simulink library "outp"  (R2021b)
(part 6 of 7)

      link override Signal_Override/_ovrdval: Value=KOUTP_FrUdcMax_V_ovrdval
  VTQD_FrUdcMin_V_Inproc : FVT_lib/outp/OverrideAndLimit  SystemSampleTime=-1  VariantActivationTime=update diagram  Latency=0  AutoFrameSizeCalculation=off
      link override Signal_Limit/_maxval: Value=KOUTP_FrUdcMin_V_maxval
      link override Signal_Limit/_minval: Value=KOUTP_FrUdcMin_V_minval
      link override Signal_Override/_ovrdflg: Value=KOUTP_FrUdcMin_V_ovrdflg
      link override Signal_Override/_ovrdval: Value=KOUTP_FrUdcMin_V_ovrdval
  VTQD_NFricPercTorq_pct_Inproc : FVT_lib/outp/OverrideAndLimit  SystemSampleTime=-1  VariantActivationTime=update diagram  Latency=0  AutoFrameSizeCalculation=off
      link override Signal_Limit/_maxval: Value=KOUTP_NFricPercTorq_pct_maxval
      link override Signal_Limit/_minval: Value=KOUTP_NFricPercTorq_pct_minval
      link override Signal_Override/_ovrdflg: Value=KOUTP_NFricPercTorq_pct_ovrdflg
      link override Signal_Override/_ovrdval: Value=KOUTP_NFricPercTorq_pct_ovrdval
  VTQD_PButtonSta_enum_Inproc : FVT_lib/outp/OverrideAndLimit  SystemSampleTime=-1  VariantActivationTime=update diagram  Latency=0  AutoFrameSizeCalculation=off
      link override Signal_Limit/_maxval: Value=KOUTP_PButtonSta_enum_maxval
      link override Signal_Limit/_minval: Value=KOUTP_PButtonSta_enum_minval
      link override Signal_Override/_ovrdflg: Value=KOUTP_PButtonSta_enum_ovrdflg
      link override Signal_Override/_ovrdval: Value=KOUTP_PButtonSta_enum_ovrdval
  VTQD_PTCSPermSta_flg_Inproc : FVT_lib/outp/OverrideAndLimit  SystemSampleTime=-1  VariantActivationTime=update diagram  Latency=0  AutoFrameSizeCalculation=off
      link override Signal_Limit/_maxval: Value=KOUTP_PTCSPermSta_flg_maxval
      link override Signal_Limit/_minval: Value=KOUTP_PTCSPermSta_flg_minval
      link override Signal_Override/_ovrdflg: Value=KOUTP_PTCSPermSta_flg_ovrdflg
      link override Signal_Override/_ovrdval: Value=KOUTP_PTCSPermSta_flg_ovrdval
  VTQD_ParkBrakeSW_enum_Inproc : FVT_lib/outp/OverrideAndLimit  SystemSampleTime=-1  VariantActivationTime=update diagram  Latency=0  AutoFrameSizeCalculation=off
      link override Signal_Limit/_maxval: Value=KOUTP_ParkBrakeSW_enum_maxval
      link override Signal_Limit/_minval: Value=KOUTP_ParkBrakeSW_enum_minval
      link override Signal_Override/_ovrdflg: Value=KOUTP_ParkBrakeSW_enum_ovrdflg
      link override Signal_Override/_ovrdval: Value=KOUTP_ParkBrakeSW_enum_ovrdval
  VTQD_ParkRequest_flg_Inproc : FVT_lib/outp/OverrideAndLimit  SystemSampleTime=-1  VariantActivationTime=update diagram  Latency=0  AutoFrameSizeCalculation=off
      link override Signal_Limit/_maxval: Value=KOUTP_ParkRequest_flg_maxval
      link override Signal_Limit/_minval: Value=KOUTP_ParkRequest_flg_minval
      link override Signal_Override/_ovrdflg: Value=KOUTP_ParkRequest_flg_ovrdflg
      link override Signal_Override/_ovrdval: Value=KOUTP_ParkRequest_flg_ovrdval
  VTQD_ReBrakeLPReq_flg_Inproc : FVT_lib/outp/OverrideAndLimit  SystemSampleTime=-1  VariantActivationTime=update diagram  Latency=0  AutoFrameSizeCalculation=off
      link override Signal_Limit/_maxval: Value=KOUTP_ReBrakeLPReq_flg_maxval
      link override Signal_Limit/_minval: Value=KOUTP_ReBrakeLPReq_flg_minval
      link override Signal_Override/_ovrdflg: Value=KOUTP_ReBrakeLPReq_flg_ovrdflg
      link override Signal_Override/_ovrdval: Value=KOUTP_ReBrakeLPReq_flg_ovrdval
  VTQD_RetSelNonEng_pct_Inproc : FVT_lib/outp/OverrideAndLimit  SystemSampleTime=-1  VariantActivationTime=update diagram  Latency=0  AutoFrameSizeCalculation=off
      link override Signal_Limit/_maxval: Value=KOUTP_RetSelNonEng_pct_maxval
      link override Signal_Limit/_minval: Value=KOUTP_RetSelNonEng_pct_minval
      link override Signal_Override/_ovrdflg: Value=KOUTP_RetSelNonEng_pct_ovrdflg
      link override Signal_Override/_ovrdval: Value=KOUTP_RetSelNonEng_pct_ovrdval
  VTQD_RgnAbnorSta_flg_Inproc : FVT_lib/outp/OverrideAndLimit  SystemSampleTime=-1  VariantActivationTime=update diagram  Latency=0  AutoFrameSizeCalculation=off
      link override Signal_Limit/_maxval: Value=KOUTP_RgnAbnorSta_flg_maxval
      link override Signal_Limit/_minval: Value=KOUTP_RgnAbnorSta_flg_minval
      link override Signal_Override/_ovrdflg: Value=KOUTP_RgnAbnorSta_flg_ovrdflg
      link override Signal_Override/_ovrdval: Value=KOUTP_RgnAbnorSta_flg_ovrdval
  VTQD_RrActvDmpDisabReq_flg_Inproc : FVT_lib/outp/OverrideAndLimit  SystemSampleTime=-1  VariantActivationTime=update diagram  Latency=0  AutoFrameSizeCalculation=off
      link override Signal_Limit/_maxval: Value=KOUTP_RrActvDmpDisabReq_flg_maxval
      link override Signal_Limit/_minval: Value=KOUTP_RrActvDmpDisabReq_flg_minval
      link override Signal_Override/_ovrdflg: Value=KOUTP_RrActvDmpDisabReq_flg_ovrdflg
      link override Signal_Override/_ovrdval: Value=KOUTP_RrActvDmpDisabReq_flg_ovrdval
  VTQD_RrEDUActTq_Nm_Inproc : FVT_lib/outp/OverrideAndLimit  SystemSampleTime=-1  VariantActivationTime=update diagram  Latency=0  AutoFrameSizeCalculation=off
      link override Signal_Limit/_maxval: Value=KOUTP_RrEDUActTq_Nm_maxval
      link override Signal_Limit/_minval: Value=KOUTP_RrEDUActTq_Nm_minval
      link override Signal_Override/_ovrdflg: Value=KOUTP_RrEDUActTq_Nm_ovrdflg
      link override Signal_Override/_ovrdval: Value=KOUTP_RrEDUActTq_Nm_ovrdval
  VTQD_RrEDUAvailBrkRgnTqV_flg_Inproc : FVT_lib/outp/OverrideAndLimit  SystemSampleTime=-1  VariantActivationTime=update diagram  Latency=0  AutoFrameSizeCalculation=off
      link override Signal_Limit/_maxval: Value=KOUTP_RrEDUAvailBrkRgnTqV_flg_maxval
      link override Signal_Limit/_minval: Value=KOUTP_RrEDUAvailBrkRgnTqV_flg_minval
      link override Signal_Override/_ovrdflg: Value=KOUTP_RrEDUAvailBrkRgnTqV_flg_ovrdflg
      link override Signal_Override/_ovrdval: Value=KOUTP_RrEDUAvailBrkRgnTqV_flg_ovrdval
  VTQD_RrEDUAvailBrkRgnTq_Nm_Inproc : FVT_lib/outp/OverrideAndLimit  SystemSampleTime=-1  VariantActivationTime=update diagram  Latency=0  AutoFrameSizeCalculation=off
      link override Signal_Limit/_maxval: Value=KOUTP_RrEDUAvailBrkRgnTq_Nm_maxval
      link override Signal_Limit/_minval: Value=KOUTP_RrEDUAvailBrkRgnTq_Nm_minval
      link override Signal_Override/_ovrdflg: Value=KOUTP_RrEDUAvailBrkRgnTq_Nm_ovrdflg
      link override Signal_Override/_ovrdval: Value=KOUTP_RrEDUAvailBrkRgnTq_Nm_ovrdval
  VTQD_RrEDURolRgnTq_Nm_Inproc : FVT_lib/outp/OverrideAndLimit  SystemSampleTime=-1  VariantActivationTime=update diagram  Latency=0  AutoFrameSizeCalculation=off
      link override Signal_Limit/_maxval: Value=KOUTP_RrEDURolRgnTq_Nm_maxval
      link override Signal_Limit/_minval: Value=KOUTP_RrEDURolRgnTq_Nm_minval
      link override Signal_Override/_ovrdflg: Value=KOUTP_RrEDURolRgnTq_Nm_ovrdflg
      link override Signal_Override/_ovrdval: Value=KOUTP_RrEDURolRgnTq_Nm_ovrdval
  VTQD_RrEDUSpdValid_flg_Inproc : FVT_lib/outp/OverrideAndLimit  SystemSampleTime=-1  VariantActivationTime=update diagram  Latency=0  AutoFrameSizeCalculation=off
      link override Signal_Limit/_maxval: Value=KOUTP_RrEDUSpdValid_flg_maxval
      link override Signal_Limit/_minval: Value=KOUTP_RrEDUSpdValid_flg_minval
      link override Signal_Override/_ovrdflg: Value=KOUTP_RrEDUSpdValid_flg_ovrdflg
      link override Signal_Override/_ovrdval: Value=KOUTP_RrEDUSpdValid_flg_ovrdval
  VTQD_RrEDUSpd_rpm_Inproc : FVT_lib/outp/OverrideAndLimit  SystemSampleTime=-1  VariantActivationTime=update diagram  Latency=0  AutoFrameSizeCalculation=off
      link override Signal_Limit/_maxval: Value=KOUTP_RrEDUSpd_rpm_maxval
      link override Signal_Limit/_minval: Value=KOUTP_RrEDUSpd_rpm_minval
      link override Signal_Override/_ovrdflg: Value=KOUTP_RrEDUSpd_rpm_ovrdflg
      link override Signal_Override/_ovrdval: Value=KOUTP_RrEDUSpd_rpm_ovrdval
  VTQD_RrIdcMax_A_Inproc : FVT_lib/outp/OverrideAndLimit  SystemSampleTime=-1  VariantActivationTime=update diagram  Latency=0  AutoFrameSizeCalculation=off
      link override Signal_Limit/_maxval: Value=KOUTP_RrIdcMax_A_maxval
      link override Signal_Limit/_minval: Value=KOUTP_RrIdcMax_A_minval
      link override Signal_Override/_ovrdflg: Value=KOUTP_RrIdcMax_A_ovrdflg
      link override Signal_Override/_ovrdval: Value=KOUTP_RrIdcMax_A_ovrdval
  VTQD_RrIdcMin_A_Inproc : FVT_lib/outp/OverrideAndLimit  SystemSampleTime=-1  VariantActivationTime=update diagram  Latency=0  AutoFrameSizeCalculation=off
      link override Signal_Limit/_maxval: Value=KOUTP_RrIdcMin_A_maxval
      link override Signal_Limit/_minval: Value=KOUTP_RrIdcMin_A_minval
      link override Signal_Override/_ovrdflg: Value=KOUTP_RrIdcMin_A_ovrdflg
      link override Signal_Override/_ovrdval: Value=KOUTP_RrIdcMin_A_ovrdval
  VTQD_RrRgnDecrSta_flg_Inproc : FVT_lib/outp/OverrideAndLimit  SystemSampleTime=-1  VariantActivationTime=update diagram  Latency=0  AutoFrameSizeCalculation=off
      link override Signal_Limit/_maxval: Value=KOUTP_RrRgnDecrSta_flg_maxval
      link override Signal_Limit/_minval: Value=KOUTP_RrRgnDecrSta_flg_minval
      link override Signal_Override/_ovrdflg: Value=KOUTP_RrRgnDecrSta_flg_ovrdflg
      link override Signal_Override/_ovrdval: Value=KOUTP_RrRgnDecrSta_flg_ovrdval
  VTQD_RrRgnPermSta_flg_Inproc : FVT_lib/outp/OverrideAndLimit  SystemSampleTime=-1  VariantActivationTime=update diagram  Latency=0  AutoFrameSizeCalculation=off
      link override Signal_Limit/_maxval: Value=KOUTP_RrRgnPermSta_flg_maxval
      link override Signal_Limit/_minval: Value=KOUTP_RrRgnPermSta_flg_minval
      link override Signal_Override/_ovrdflg: Value=KOUTP_RrRgnPermSta_flg_ovrdflg
      link override Signal_Override/_ovrdval: Value=KOUTP_RrRgnPermSta_flg_ovrdval
  VTQD_RrUdcMax_V_Inproc : FVT_lib/outp/OverrideAndLimit  SystemSampleTime=-1  VariantActivationTime=update diagram  Latency=0  AutoFrameSizeCalculation=off
      link override Signal_Limit/_maxval: Value=KOUTP_RrUdcMax_V_maxval
      link override Signal_Limit/_minval: Value=KOUTP_RrUdcMax_V_minval
      link override Signal_Override/_ovrdflg: Value=KOUTP_RrUdcMax_V_ovrdflg
      link override Signal_Override/_ovrdval: Value=KOUTP_RrUdcMax_V_ovrdval
  VTQD_RrUdcMin_V_Inproc : FVT_lib/outp/OverrideAndLimit  SystemSampleTime=-1  VariantActivationTime=update diagram  Latency=0  AutoFrameSizeCalculation=off
      link override Signal_Limit/_maxval: Value=KOUTP_RrUdcMin_V_maxval
      link override Signal_Limit/_minval: Value=KOUTP_RrUdcMin_V_minval
      link override Signal_Override/_ovrdflg: Value=KOUTP_RrUdcMin_V_ovrdflg
      link override Signal_Override/_ovrdval: Value=KOUTP_RrUdcMin_V_ovrdval
  VTQD_SACtrlDev_enum_Inproc : FVT_lib/outp/OverrideAndLimit  SystemSampleTime=-1  VariantActivationTime=update diagram  Latency=0  AutoFrameSizeCalculation=off
      link override Signal_Limit/_maxval: Value=KOUTP_SACtrlDev_enum_maxval
      link override Signal_Limit/_minval: Value=KOUTP_SACtrlDev_enum_minval
      link override Signal_Override/_ovrdflg: Value=KOUTP_SACtrlDev_enum_ovrdflg
      link override Signal_Override/_ovrdval: Value=KOUTP_SACtrlDev_enum_ovrdval
  VTQD_ShiftGearPosn_enum_Inproc : FVT_lib/outp/OverrideAndLimit  SystemSampleTime=-1  VariantActivationTime=update diagram  Latency=0  AutoFrameSizeCalculation=off
      link override Signal_Limit/_maxval: Value=KOUTP_ShiftGearPosn_enum_maxval
      link override Signal_Limit/_minval: Value=KOUTP_ShiftGearPosn_enum_minval
      link override Signal_Override/_ovrdflg: Value=KOUTP_ShiftGearPosn_enum_ovrdflg
      link override Signal_Override/_ovrdval: Value=KOUTP_ShiftGearPosn_enum_ovrdval
  VTQD_ShiftPgs_enum_Inproc : FVT_lib/outp/OverrideAndLimit  SystemSampleTime=-1  VariantActivationTime=update diagram  Latency=0  AutoFrameSizeCalculation=off
      link override Signal_Limit/_maxval: Value=KOUTP_ShiftPgs_enum_maxval
      link override Signal_Limit/_minval: Value=KOUTP_ShiftPgs_enum_minval
      link override Signal_Override/_ovrdflg: Value=KOUTP_ShiftPgs_enum_ovrdflg
      link override Signal_Override/_ovrdval: Value=KOUTP_ShiftPgs_enum_ovrdval
  VTQD_TqSourceFr_enum_Inproc : FVT_lib/outp/OverrideAndLimit  SystemSampleTime=-1  VariantActivationTime=update diagram  Latency=0  AutoFrameSizeCalculation=off
      link override Signal_Limit/_maxval: Value=KOUTP_TqSourceFr_enum_maxval
      link override Signal_Limit/_minval: Value=KOUTP_TqSourceFr_enum_minval
      link override Signal_Override/_ovrdflg: Value=KOUTP_TqSourceFr_enum_ovrdflg
      link override Signal_Override/_ovrdval: Value=KOUTP_TqSourceFr_enum_ovrdval
  VTQD_TqSourceRr_enum_Inproc : FVT_lib/outp/OverrideAndLimit  SystemSampleTime=-1  VariantActivationTime=update diagram  Latency=0  AutoFrameSizeCalculation=off
      link override Signal_Limit/_maxval: Value=KOUTP_TqSourceRr_enum_maxval
      link override Signal_Limit/_minval: Value=KOUTP_TqSourceRr_enum_minval
      link override Signal_Override/_ovrdflg: Value=KOUTP_TqSourceRr_enum_ovrdflg
      link override Signal_Override/_ovrdval: Value=KOUTP_TqSourceRr_enum_ovrdval
  VTQD_VCUVehSpd_kph_Inproc : FVT_lib/outp/OverrideAndLimit  SystemSampleTime=-1  VariantActivationTime=update diagram  Latency=0  AutoFrameSizeCalculation=off
      link override Signal_Limit/_maxval: Value=KOUTP_VCUVehSpd_kph_maxval
      link override Signal_Limit/_minval: Value=KOUTP_VCUVehSpd_kph_minval
      link override Signal_Override/_ovrdflg: Value=KOUTP_VCUVehSpd_kph_ovrdflg
      link override Signal_Override/_ovrdval: Value=KOUTP_VCUVehSpd_kph_ovrdval
  VTQR_FrTMTqReq_Nm_Inproc : FVT_lib/outp/OverrideAndLimit  SystemSampleTime=-1  VariantActivationTime=update diagram  Latency=0  AutoFrameSizeCalculation=off
      link override Signal_Limit/_maxval: Value=KOUTP_FrTMTqReq_Nm_maxval
      link override Signal_Limit/_minval: Value=KOUTP_FrTMTqReq_Nm_minval
      link override Signal_Override/_ovrdflg: Value=KOUTP_FrTMTqReq_Nm_ovrdflg
      link override Signal_Override/_ovrdval: Value=KOUTP_FrTMTqReq_Nm_ovrdval
  VTQR_RrTMTqReq_Nm_Inproc : FVT_lib/outp/OverrideAndLimit  SystemSampleTime=-1  VariantActivationTime=update diagram  Latency=0  AutoFrameSizeCalculation=off
      link override Signal_Limit/_maxval: Value=KOUTP_RrTMTqReq_Nm_maxval
      link override Signal_Limit/_minval: Value=KOUTP_RrTMTqReq_Nm_minval
      link override Signal_Override/_ovrdflg: Value=KOUTP_RrTMTqReq_Nm_ovrdflg
      link override Signal_Override/_ovrdval: Value=KOUTP_RrTMTqReq_Nm_ovrdval
  VV2L_ReqOBCV2LEna_enum_Inproc : FVT_lib/outp/OverrideAndLimit  SystemSampleTime=-1  VariantActivationTime=update diagram  Latency=0  AutoFrameSizeCalculation=off
      link override Signal_Limit/_maxval: Value=KOUTP_ReqOBCV2LEna_enum_maxval
      link override Signal_Limit/_minval: Value=KOUTP_ReqOBCV2LEna_enum_minval
      link override Signal_Override/_ovrdflg: Value=KOUTP_ReqOBCV2LEna_enum_ovrdflg
      link override Signal_Override/_ovrdval: Value=KOUTP_ReqOBCV2LEna_enum_ovrdval
  VV2L_ReqV2LIVIPopup_enum_Inproc : FVT_lib/outp/OverrideAndLimit  SystemSampleTime=-1  VariantActivationTime=update diagram  Latency=0  AutoFrameSizeCalculation=off
      link override Signal_Limit/_maxval: Value=KOUTP_ReqV2LIVIPopup_enum_maxval
      link override Signal_Limit/_minval: Value=KOUTP_ReqV2LIVIPopup_enum_minval
      link override Signal_Override/_ovrdflg: Value=KOUTP_ReqV2LIVIPopup_enum_ovrdflg
      link override Signal_Override/_ovrdval: Value=KOUTP_ReqV2LIVIPopup_enum_ovrdval
  VVMC_ACCComfortBandLower_mps2_Inproc : FVT_lib/outp/OverrideAndLimit  SystemSampleTime=-1  VariantActivationTime=update diagram  Latency=0  AutoFrameSizeCalculation=off
      link override Signal_Limit/_maxval: Value=KOUTP_ACCComfortBandLower_mps2_maxval
      link override Signal_Limit/_minval: Value=KOUTP_ACCComfortBandLower_mps2_minval
      link override Signal_Override/_ovrdflg: Value=KOUTP_ACCComfortBandLower_mps2_ovrdflg
      link override Signal_Override/_ovrdval: Value=KOUTP_ACCComfortBandLower_mps2_ovrdval
  VVMC_ACCComfortBandUpper_mps2_Inproc : FVT_lib/outp/OverrideAndLimit  SystemSampleTime=-1  VariantActivationTime=update diagram  Latency=0  AutoFrameSizeCalculation=off
      link override Signal_Limit/_maxval: Value=KOUTP_ACCComfortBandUpper_mps2_maxval
      link override Signal_Limit/_minval: Value=KOUTP_ACCComfortBandUpper_mps2_minval
      link override Signal_Override/_ovrdflg: Value=KOUTP_ACCComfortBandUpper_mps2_ovrdflg
      link override Signal_Override/_ovrdval: Value=KOUTP_ACCComfortBandUpper_mps2_ovrdval
  VVMC_ACCCtrlAvail_flg_Inproc : FVT_lib/outp/OverrideAndLimit  SystemSampleTime=-1  VariantActivationTime=update diagram  Latency=0  AutoFrameSizeCalculation=off
      link override Signal_Limit/_maxval: Value=KOUTP_ACCCtrlAvail_flg_maxval
      link override Signal_Limit/_minval: Value=KOUTP_ACCCtrlAvail_flg_minval
      link override Signal_Override/_ovrdflg: Value=KOUTP_ACCCtrlAvail_flg_ovrdflg
      link override Signal_Override/_ovrdval: Value=KOUTP_ACCCtrlAvail_flg_ovrdval
  VVMC_ACCJerkLowerLimit_mps3_Inproc : FVT_lib/outp/OverrideAndLimit  SystemSampleTime=-1  VariantActivationTime=update diagram  Latency=0  AutoFrameSizeCalculation=off
      link override Signal_Limit/_maxval: Value=KOUTP_ACCJerkLowerLimit_mps3_maxval
      link override Signal_Limit/_minval: Value=KOUTP_ACCJerkLowerLimit_mps3_minval
      link override Signal_Override/_ovrdflg: Value=KOUTP_ACCJerkLowerLimit_mps3_ovrdflg
      link override Signal_Override/_ovrdval: Value=KOUTP_ACCJerkLowerLimit_mps3_ovrdval
  VVMC_ACCJerkUpperLimit_mps3_Inproc : FVT_lib/outp/OverrideAndLimit  SystemSampleTime=-1  VariantActivationTime=update diagram  Latency=0  AutoFrameSizeCalculation=off
      link override Signal_Limit/_maxval: Value=KOUTP_ACCJerkUpperLimit_mps3_maxval
      link override Signal_Limit/_minval: Value=KOUTP_ACCJerkUpperLimit_mps3_minval
      link override Signal_Override/_ovrdflg: Value=KOUTP_ACCJerkUpperLimit_mps3_ovrdflg
      link override Signal_Override/_ovrdval: Value=KOUTP_ACCJerkUpperLimit_mps3_ovrdval
  VVMC_ACCObjDist_m_Inproc : FVT_lib/outp/OverrideAndLimit  SystemSampleTime=-1  VariantActivationTime=update diagram  Latency=0  AutoFrameSizeCalculation=off
      link override Signal_Limit/_maxval: Value=KOUTP_ACCObjDist_m_maxval
      link override Signal_Limit/_minval: Value=KOUTP_ACCObjDist_m_minval
      link override Signal_Override/_ovrdflg: Value=KOUTP_ACCObjDist_m_ovrdflg
      link override Signal_Override/_ovrdval: Value=KOUTP_ACCObjDist_m_ovrdval
  VVMC_ACCObjDstLvl_enum_Inproc : FVT_lib/outp/OverrideAndLimit  SystemSampleTime=-1  VariantActivationTime=update diagram  Latency=0  AutoFrameSizeCalculation=off
      link override Signal_Limit/_maxval: Value=KOUTP_ACCObjDstLvl_enum_maxval
      link override Signal_Limit/_minval: Value=KOUTP_ACCObjDstLvl_enum_minval
      link override Signal_Override/_ovrdflg: Value=KOUTP_ACCObjDstLvl_enum_ovrdflg
      link override Signal_Override/_ovrdval: Value=KOUTP_ACCObjDstLvl_enum_ovrdval
  VVMC_ACCObjRelSpd_mps_Inproc : FVT_lib/outp/OverrideAndLimit  SystemSampleTime=-1  VariantActivationTime=update diagram  Latency=0  AutoFrameSizeCalculation=off
      link override Signal_Limit/_maxval: Value=KOUTP_ACCObjRelSpd_mps_maxval
      link override Signal_Limit/_minval: Value=KOUTP_ACCObjRelSpd_mps_minval
      link override Signal_Override/_ovrdflg: Value=KOUTP_ACCObjRelSpd_mps_ovrdflg
      link override Signal_Override/_ovrdval: Value=KOUTP_ACCObjRelSpd_mps_ovrdval
  VVMC_ACCPedalOvrd_flg_Inproc : FVT_lib/outp/OverrideAndLimit  SystemSampleTime=-1  VariantActivationTime=update diagram  Latency=0  AutoFrameSizeCalculation=off
      link override Signal_Limit/_maxval: Value=KOUTP_ACCPedalOvrd_flg_maxval
      link override Signal_Limit/_minval: Value=KOUTP_ACCPedalOvrd_flg_minval
      link override Signal_Override/_ovrdflg: Value=KOUTP_ACCPedalOvrd_flg_ovrdflg
      link override Signal_Override/_ovrdval: Value=KOUTP_ACCPedalOvrd_flg_ovrdval
  VVMC_ACCRequiredAccel_mps2_Inproc : FVT_lib/outp/OverrideAndLimit  SystemSampleTime=-1  VariantActivationTime=update diagram  Latency=0  AutoFrameSizeCalculation=off
      link override Signal_Limit/_maxval: Value=KOUTP_ACCRequiredAccel_mps2_maxval
      link override Signal_Limit/_minval: Value=KOUTP_ACCRequiredAccel_mps2_minval
      link override Signal_Override/_ovrdflg: Value=KOUTP_ACCRequiredAccel_mps2_ovrdflg
      link override Signal_Override/_ovrdval: Value=KOUTP_ACCRequiredAccel_mps2_ovrdval
  VVMC_ACCTakeoverReq_flg_Inproc : FVT_lib/outp/OverrideAndLimit  SystemSampleTime=-1  VariantActivationTime=update diagram  Latency=0  AutoFrameSizeCalculation=off
      link override Signal_Limit/_maxval: Value=KOUTP_ACCTakeoverReq_flg_maxval
      link override Signal_Limit/_minval: Value=KOUTP_ACCTakeoverReq_flg_minval
      link override Signal_Override/_ovrdflg: Value=KOUTP_ACCTakeoverReq_flg_ovrdflg
      link override Signal_Override/_ovrdval: Value=KOUTP_ACCTakeoverReq_flg_ovrdval
  VVMC_ACCVehHoldReq_flg_Inproc : FVT_lib/outp/OverrideAndLimit  SystemSampleTime=-1  VariantActivationTime=update diagram  Latency=0  AutoFrameSizeCalculation=off
      link override Signal_Limit/_maxval: Value=KOUTP_ACCVehHoldReq_flg_maxval
      link override Signal_Limit/_minval: Value=KOUTP_ACCVehHoldReq_flg_minval
      link override Signal_Override/_ovrdflg: Value=KOUTP_ACCVehHoldReq_flg_ovrdflg
      link override Signal_Override/_ovrdval: Value=KOUTP_ACCVehHoldReq_flg_ovrdval
  VVMC_ADASACCSta_enum_Inproc : FVT_lib/outp/OverrideAndLimit  SystemSampleTime=-1  VariantActivationTime=update diagram  Latency=0  AutoFrameSizeCalculation=off
      link override Signal_Limit/_maxval: Value=KOUTP_ADASACCSta_enum_maxval
      link override Signal_Limit/_minval: Value=KOUTP_ADASACCSta_enum_minval
      link override Signal_Override/_ovrdflg: Value=KOUTP_ADASACCSta_enum_ovrdflg
      link override Signal_Override/_ovrdval: Value=KOUTP_ADASACCSta_enum_ovrdval
  VVMC_ADASAEBReq_enum_Inproc : FVT_lib/outp/OverrideAndLimit  SystemSampleTime=-1  VariantActivationTime=update diagram  Latency=0  AutoFrameSizeCalculation=off
      link override Signal_Limit/_maxval: Value=KOUTP_ADASAEBReq_enum_maxval
      link override Signal_Limit/_minval: Value=KOUTP_ADASAEBReq_enum_minval
      link override Signal_Override/_ovrdflg: Value=KOUTP_ADASAEBReq_enum_ovrdflg
      link override Signal_Override/_ovrdval: Value=KOUTP_ADASAEBReq_enum_ovrdval
  VVMC_ADASAEBSta_enum_Inproc : FVT_lib/outp/OverrideAndLimit  SystemSampleTime=-1  VariantActivationTime=update diagram  Latency=0  AutoFrameSizeCalculation=off
      link override Signal_Limit/_maxval: Value=KOUTP_ADASAEBSta_enum_maxval
      link override Signal_Limit/_minval: Value=KOUTP_ADASAEBSta_enum_minval
      link override Signal_Override/_ovrdflg: Value=KOUTP_ADASAEBSta_enum_ovrdflg
      link override Signal_Override/_ovrdval: Value=KOUTP_ADASAEBSta_enum_ovrdval
  VVMC_ADASCAMSpdLim_enum_Inproc : FVT_lib/outp/OverrideAndLimit  SystemSampleTime=-1  VariantActivationTime=update diagram  Latency=0  AutoFrameSizeCalculation=off
      link override Signal_Limit/_maxval: Value=KOUTP_ADASCAMSpdLim_enum_maxval
      link override Signal_Limit/_minval: Value=KOUTP_ADASCAMSpdLim_enum_minval
      link override Signal_Override/_ovrdflg: Value=KOUTP_ADASCAMSpdLim_enum_ovrdflg
      link override Signal_Override/_ovrdval: Value=KOUTP_ADASCAMSpdLim_enum_ovrdval
  VVMC_ADASDBSReq_enum_Inproc : FVT_lib/outp/OverrideAndLimit  SystemSampleTime=-1  VariantActivationTime=update diagram  Latency=0  AutoFrameSizeCalculation=off
      link override Signal_Limit/_maxval: Value=KOUTP_ADASDBSReq_enum_maxval
      link override Signal_Limit/_minval: Value=KOUTP_ADASDBSReq_enum_minval
      link override Signal_Override/_ovrdflg: Value=KOUTP_ADASDBSReq_enum_ovrdflg
      link override Signal_Override/_ovrdval: Value=KOUTP_ADASDBSReq_enum_ovrdval
  VVMC_ADASFCWMute_flg_Inproc : FVT_lib/outp/OverrideAndLimit  SystemSampleTime=-1  VariantActivationTime=update diagram  Latency=0  AutoFrameSizeCalculation=off
      link override Signal_Limit/_maxval: Value=KOUTP_ADASFCWMute_flg_maxval
      link override Signal_Limit/_minval: Value=KOUTP_ADASFCWMute_flg_minval
      link override Signal_Override/_ovrdflg: Value=KOUTP_ADASFCWMute_flg_ovrdflg
      link override Signal_Override/_ovrdval: Value=KOUTP_ADASFCWMute_flg_ovrdval
  VVMC_ADASFCWSta_enum_Inproc : FVT_lib/outp/OverrideAndLimit  SystemSampleTime=-1  VariantActivationTime=update diagram  Latency=0  AutoFrameSizeCalculation=off
      link override Signal_Limit/_maxval: Value=KOUTP_ADASFCWSta_enum_maxval
      link override Signal_Limit/_minval: Value=KOUTP_ADASFCWSta_enum_minval
      link override Signal_Override/_ovrdflg: Value=KOUTP_ADASFCWSta_enum_ovrdflg
      link override Signal_Override/_ovrdval: Value=KOUTP_ADASFCWSta_enum_ovrdval
  VVMC_ADASFaultSta_flg_Inproc : FVT_lib/outp/OverrideAndLimit  SystemSampleTime=-1  VariantActivationTime=update diagram  Latency=0  AutoFrameSizeCalculation=off
      link override Signal_Limit/_maxval: Value=KOUTP_ADASFaultSta_flg_maxval
      link override Signal_Limit/_minval: Value=KOUTP_ADASFaultSta_flg_minval
      link override Signal_Override/_ovrdflg: Value=KOUTP_ADASFaultSta_flg_ovrdflg
      link override Signal_Override/_ovrdval: Value=KOUTP_ADASFaultSta_flg_ovrdval
  VVMC_ADASFltWrnReq_flg_Inproc : FVT_lib/outp/OverrideAndLimit  SystemSampleTime=-1  VariantActivationTime=update diagram  Latency=0  AutoFrameSizeCalculation=off
      link override Signal_Limit/_maxval: Value=KOUTP_ADASFltWrnReq_flg_maxval
      link override Signal_Limit/_minval: Value=KOUTP_ADASFltWrnReq_flg_minval
      link override Signal_Override/_ovrdflg: Value=KOUTP_ADASFltWrnReq_flg_ovrdflg
      link override Signal_Override/_ovrdval: Value=KOUTP_ADASFltWrnReq_flg_ovrdval
  VVMC_ADASForceIdle_flg_Inproc : FVT_lib/outp/OverrideAndLimit  SystemSampleTime=-1  VariantActivationTime=update diagram  Latency=0  AutoFrameSizeCalculation=off
      link override Signal_Limit/_maxval: Value=KOUTP_ADASForceIdle_flg_maxval
      link override Signal_Limit/_minval: Value=KOUTP_ADASForceIdle_flg_minval
      link override Signal_Override/_ovrdflg: Value=KOUTP_ADASForceIdle_flg_ovrdflg
      link override Signal_Override/_ovrdval: Value=KOUTP_ADASForceIdle_flg_ovrdval
  VVMC_ADASISASta_enum_Inproc : FVT_lib/outp/OverrideAndLimit  SystemSampleTime=-1  VariantActivationTime=update diagram  Latency=0  AutoFrameSizeCalculation=off
      link override Signal_Limit/_maxval: Value=KOUTP_ADASISASta_enum_maxval
      link override Signal_Limit/_minval: Value=KOUTP_ADASISASta_enum_minval
      link override Signal_Override/_ovrdflg: Value=KOUTP_ADASISASta_enum_ovrdflg
      link override Signal_Override/_ovrdval: Value=KOUTP_ADASISASta_enum_ovrdval
  VVMC_ADASLDWMute_flg_Inproc : FVT_lib/outp/OverrideAndLimit  SystemSampleTime=-1  VariantActivationTime=update diagram  Latency=0  AutoFrameSizeCalculation=off
      link override Signal_Limit/_maxval: Value=KOUTP_ADASLDWMute_flg_maxval
      link override Signal_Limit/_minval: Value=KOUTP_ADASLDWMute_flg_minval
      link override Signal_Override/_ovrdflg: Value=KOUTP_ADASLDWMute_flg_ovrdflg
      link override Signal_Override/_ovrdval: Value=KOUTP_ADASLDWMute_flg_ovrdval
  VVMC_ADASLDWSta_enum_Inproc : FVT_lib/outp/OverrideAndLimit  SystemSampleTime=-1  VariantActivationTime=update diagram  Latency=0  AutoFrameSizeCalculation=off
      link override Signal_Limit/_maxval: Value=KOUTP_ADASLDWSta_enum_maxval
      link override Signal_Limit/_minval: Value=KOUTP_ADASLDWSta_enum_minval
      link override Signal_Override/_ovrdflg: Value=KOUTP_ADASLDWSta_enum_ovrdflg
      link override Signal_Override/_ovrdval: Value=KOUTP_ADASLDWSta_enum_ovrdval
  VVMC_ADASLFCHandsOffWarning_enum_Inproc : FVT_lib/outp/OverrideAndLimit  SystemSampleTime=-1  VariantActivationTime=update diagram  Latency=0  AutoFrameSizeCalculation=off
      link override Signal_Limit/_maxval: Value=KOUTP_ADASLFCHandsOffWarning_enum_maxval
      link override Signal_Limit/_minval: Value=KOUTP_ADASLFCHandsOffWarning_enum_minval
      link override Signal_Override/_ovrdflg: Value=KOUTP_ADASLFCHandsOffWarning_enum_ovrdflg
      link override Signal_Override/_ovrdval: Value=KOUTP_ADASLFCHandsOffWarning_enum_ovrdval
  VVMC_ADASLFCSta_enum_Inproc : FVT_lib/outp/OverrideAndLimit  SystemSampleTime=-1  VariantActivationTime=update diagram  Latency=0  AutoFrameSizeCalculation=off
      link override Signal_Limit/_maxval: Value=KOUTP_ADASLFCSta_enum_maxval
      link override Signal_Limit/_minval: Value=KOUTP_ADASLFCSta_enum_minval
      link override Signal_Override/_ovrdflg: Value=KOUTP_ADASLFCSta_enum_ovrdflg
      link override Signal_Override/_ovrdval: Value=KOUTP_ADASLFCSta_enum_ovrdval
  VVMC_ADASLFCWarnSound_enum_Inproc : FVT_lib/outp/OverrideAndLimit  SystemSampleTime=-1  VariantActivationTime=update diagram  Latency=0  AutoFrameSizeCalculation=off
      link override Signal_Limit/_maxval: Value=KOUTP_ADASLFCWarnSound_enum_maxval
      link override Signal_Limit/_minval: Value=KOUTP_ADASLFCWarnSound_enum_minval
      link override Signal_Override/_ovrdflg: Value=KOUTP_ADASLFCWarnSound_enum_ovrdflg
      link override Signal_Override/_ovrdval: Value=KOUTP_ADASLFCWarnSound_enum_ovrdval
  VVMC_ADASLKASta_enum_Inproc : FVT_lib/outp/OverrideAndLimit  SystemSampleTime=-1  VariantActivationTime=update diagram  Latency=0  AutoFrameSizeCalculation=off
      link override Signal_Limit/_maxval: Value=KOUTP_ADASLKASta_enum_maxval
      link override Signal_Limit/_minval: Value=KOUTP_ADASLKASta_enum_minval
      link override Signal_Override/_ovrdflg: Value=KOUTP_ADASLKASta_enum_ovrdflg
      link override Signal_Override/_ovrdval: Value=KOUTP_ADASLKASta_enum_ovrdval
  VVMC_ADASLaneModeL_enum_Inproc : FVT_lib/outp/OverrideAndLimit  SystemSampleTime=-1  VariantActivationTime=update diagram  Latency=0  AutoFrameSizeCalculation=off
      link override Signal_Limit/_maxval: Value=KOUTP_ADASLaneModeL_enum_maxval
      link override Signal_Limit/_minval: Value=KOUTP_ADASLaneModeL_enum_minval
      link override Signal_Override/_ovrdflg: Value=KOUTP_ADASLaneModeL_enum_ovrdflg
      link override Signal_Override/_ovrdval: Value=KOUTP_ADASLaneModeL_enum_ovrdval
  VVMC_ADASLaneModeR_enum_Inproc : FVT_lib/outp/OverrideAndLimit  SystemSampleTime=-1  VariantActivationTime=update diagram  Latency=0  AutoFrameSizeCalculation=off
      link override Signal_Limit/_maxval: Value=KOUTP_ADASLaneModeR_enum_maxval
      link override Signal_Limit/_minval: Value=KOUTP_ADASLaneModeR_enum_minval
      link override Signal_Override/_ovrdflg: Value=KOUTP_ADASLaneModeR_enum_ovrdflg
      link override Signal_Override/_ovrdval: Value=KOUTP_ADASLaneModeR_enum_ovrdval
  VVMC_ADASLanecurveL_raw32_Inproc : FVT_lib/outp/OverrideAndLimit  SystemSampleTime=-1  VariantActivationTime=update diagram  Latency=0  AutoFrameSizeCalculation=off
      link override Signal_Limit/_maxval: Value=KOUTP_ADASLanecurveL_raw32_maxval
      link override Signal_Limit/_minval: Value=KOUTP_ADASLanecurveL_raw32_minval
      link override Signal_Override/_ovrdflg: Value=KOUTP_ADASLanecurveL_raw32_ovrdflg
      link override Signal_Override/_ovrdval: Value=KOUTP_ADASLanecurveL_raw32_ovrdval
  VVMC_ADASLanecurveR_raw32_Inproc : FVT_lib/outp/OverrideAndLimit  SystemSampleTime=-1  VariantActivationTime=update diagram  Latency=0  AutoFrameSizeCalculation=off
      link override Signal_Limit/_maxval: Value=KOUTP_ADASLanecurveR_raw32_maxval
      link override Signal_Limit/_minval: Value=KOUTP_ADASLanecurveR_raw32_minval
      link override Signal_Override/_ovrdflg: Value=KOUTP_ADASLanecurveR_raw32_ovrdflg
      link override Signal_Override/_ovrdval: Value=KOUTP_ADASLanecurveR_raw32_ovrdval
  VVMC_ADASLanetypeL_enum_Inproc : FVT_lib/outp/OverrideAndLimit  SystemSampleTime=-1  VariantActivationTime=update diagram  Latency=0  AutoFrameSizeCalculation=off
      link override Signal_Limit/_maxval: Value=KOUTP_ADASLanetypeL_enum_maxval
      link override Signal_Limit/_minval: Value=KOUTP_ADASLanetypeL_enum_minval
      link override Signal_Override/_ovrdflg: Value=KOUTP_ADASLanetypeL_enum_ovrdflg
      link override Signal_Override/_ovrdval: Value=KOUTP_ADASLanetypeL_enum_ovrdval
  VVMC_ADASLanetypeR_enum_Inproc : FVT_lib/outp/OverrideAndLimit  SystemSampleTime=-1  VariantActivationTime=update diagram  Latency=0  AutoFrameSizeCalculation=off
      link override Signal_Limit/_maxval: Value=KOUTP_ADASLanetypeR_enum_maxval
      link override Signal_Limit/_minval: Value=KOUTP_ADASLanetypeR_enum_minval
      link override Signal_Override/_ovrdflg: Value=KOUTP_ADASLanetypeR_enum_ovrdflg
      link override Signal_Override/_ovrdval: Value=KOUTP_ADASLanetypeR_enum_ovrdval
  VVMC_ADASSLIFSpdLim_enum_Inproc : FVT_lib/outp/OverrideAndLimit  SystemSampleTime=-1  VariantActivationTime=update diagram  Latency=0  AutoFrameSizeCalculation=off
      link override Signal_Limit/_maxval: Value=KOUTP_ADASSLIFSpdLim_enum_maxval
      link override Signal_Limit/_minval: Value=KOUTP_ADASSLIFSpdLim_enum_minval
      link override Signal_Override/_ovrdflg: Value=KOUTP_ADASSLIFSpdLim_enum_ovrdflg
      link override Signal_Override/_ovrdval: Value=KOUTP_ADASSLIFSpdLim_enum_ovrdval
  VVMC_ADASSLIFSta_enum_Inproc : FVT_lib/outp/OverrideAndLimit  SystemSampleTime=-1  VariantActivationTime=update diagram  Latency=0  AutoFrameSizeCalculation=off
      link override Signal_Limit/_maxval: Value=KOUTP_ADASSLIFSta_enum_maxval
      link override Signal_Limit/_minval: Value=KOUTP_ADASSLIFSta_enum_minval
      link override Signal_Override/_ovrdflg: Value=KOUTP_ADASSLIFSta_enum_ovrdflg
      link override Signal_Override/_ovrdval: Value=KOUTP_ADASSLIFSta_enum_ovrdval
  VVMC_ADASShftPosnReqA_flg_Inproc : FVT_lib/outp/OverrideAndLimit  SystemSampleTime=-1  VariantActivationTime=update diagram  Latency=0  AutoFrameSizeCalculation=off
      link override Signal_Limit/_maxval: Value=KOUTP_ADASShftPosnReqA_flg_maxval
      link override Signal_Limit/_minval: Value=KOUTP_ADASShftPosnReqA_flg_minval
      link override Signal_Override/_ovrdflg: Value=KOUTP_ADASShftPosnReqA_flg_ovrdflg
      link override Signal_Override/_ovrdval: Value=KOUTP_ADASShftPosnReqA_flg_ovrdval
  VVMC_ADASShftPosnReq_enum_Inproc : FVT_lib/outp/OverrideAndLimit  SystemSampleTime=-1  VariantActivationTime=update diagram  Latency=0  AutoFrameSizeCalculation=off
      link override Signal_Limit/_maxval: Value=KOUTP_ADASShftPosnReq_enum_maxval
      link override Signal_Limit/_minval: Value=KOUTP_ADASShftPosnReq_enum_minval
      link override Signal_Override/_ovrdflg: Value=KOUTP_ADASShftPosnReq_enum_ovrdflg
      link override Signal_Override/_ovrdval: Value=KOUTP_ADASShftPosnReq_enum_ovrdval
  VVMC_ADASVehSpdLim_raw32_Inproc : FVT_lib/outp/OverrideAndLimit  SystemSampleTime=-1  VariantActivationTime=update diagram  Latency=0  AutoFrameSizeCalculation=off
      link override Signal_Limit/_maxval: Value=KOUTP_ADASVehSpdLim_raw32_maxval
      link override Signal_Limit/_minval: Value=KOUTP_ADASVehSpdLim_raw32_minval
      link override Signal_Override/_ovrdflg: Value=KOUTP_ADASVehSpdLim_raw32_ovrdflg
      link override Signal_Override/_ovrdval: Value=KOUTP_ADASVehSpdLim_raw32_ovrdval
  VVMC_ADASWarningMsg_enum_Inproc : FVT_lib/outp/OverrideAndLimit  SystemSampleTime=-1  VariantActivationTime=update diagram  Latency=0  AutoFrameSizeCalculation=off
      link override Signal_Limit/_maxval: Value=KOUTP_ADASWarningMsg_enum_maxval
      link override Signal_Limit/_minval: Value=KOUTP_ADASWarningMsg_enum_minval
      link override Signal_Override/_ovrdflg: Value=KOUTP_ADASWarningMsg_enum_ovrdflg
      link override Signal_Override/_ovrdval: Value=KOUTP_ADASWarningMsg_enum_ovrdval
  VVMC_AEBVehHoldReq_flg_Inproc : FVT_lib/outp/OverrideAndLimit  SystemSampleTime=-1  VariantActivationTime=update diagram  Latency=0  AutoFrameSizeCalculation=off
      link override Signal_Limit/_maxval: Value=KOUTP_AEBVehHoldReq_flg_maxval
      link override Signal_Limit/_minval: Value=KOUTP_AEBVehHoldReq_flg_minval
      link override Signal_Override/_ovrdflg: Value=KOUTP_AEBVehHoldReq_flg_ovrdflg
      link override Signal_Override/_ovrdval: Value=KOUTP_AEBVehHoldReq_flg_ovrdval
  VVMC_APSCtrlAvail_flg_Inproc : FVT_lib/outp/OverrideAndLimit  SystemSampleTime=-1  VariantActivationTime=update diagram  Latency=0  AutoFrameSizeCalculation=off
      link override Signal_Limit/_maxval: Value=KOUTP_APSCtrlAvail_flg_maxval
      link override Signal_Limit/_minval: Value=KOUTP_APSCtrlAvail_flg_minval
      link override Signal_Override/_ovrdflg: Value=KOUTP_APSCtrlAvail_flg_ovrdflg
      link override Signal_Override/_ovrdval: Value=KOUTP_APSCtrlAvail_flg_ovrdval
  VVMC_APSDecReqA_flg_Inproc : FVT_lib/outp/OverrideAndLimit  SystemSampleTime=-1  VariantActivationTime=update diagram  Latency=0  AutoFrameSizeCalculation=off
      link override Signal_Limit/_maxval: Value=KOUTP_APSDecReqA_flg_maxval
      link override Signal_Limit/_minval: Value=KOUTP_APSDecReqA_flg_minval
      link override Signal_Override/_ovrdflg: Value=KOUTP_APSDecReqA_flg_ovrdflg
      link override Signal_Override/_ovrdval: Value=KOUTP_APSDecReqA_flg_ovrdval
  VVMC_APSDecReq_mps2_Inproc : FVT_lib/outp/OverrideAndLimit  SystemSampleTime=-1  VariantActivationTime=update diagram  Latency=0  AutoFrameSizeCalculation=off
      link override Signal_Limit/_maxval: Value=KOUTP_APSDecReq_mps2_maxval
      link override Signal_Limit/_minval: Value=KOUTP_APSDecReq_mps2_minval
      link override Signal_Override/_ovrdflg: Value=KOUTP_APSDecReq_mps2_ovrdflg
      link override Signal_Override/_ovrdval: Value=KOUTP_APSDecReq_mps2_ovrdval
  VVMC_APSReq_enum_Inproc : FVT_lib/outp/OverrideAndLimit  SystemSampleTime=-1  VariantActivationTime=update diagram  Latency=0  AutoFrameSizeCalculation=off
      link override Signal_Limit/_maxval: Value=KOUTP_APSReq_enum_maxval
      link override Signal_Limit/_minval: Value=KOUTP_APSReq_enum_minval
      link override Signal_Override/_ovrdflg: Value=KOUTP_APSReq_enum_ovrdflg
      link override Signal_Override/_ovrdval: Value=KOUTP_APSReq_enum_ovrdval
  VVMC_APSStaSys_enum_Inproc : FVT_lib/outp/OverrideAndLimit  SystemSampleTime=-1  VariantActivationTime=update diagram  Latency=0  AutoFrameSizeCalculation=off
      link override Signal_Limit/_maxval: Value=KOUTP_APSStaSys_enum_maxval
      link override Signal_Limit/_minval: Value=KOUTP_APSStaSys_enum_minval
      link override Signal_Override/_ovrdflg: Value=KOUTP_APSStaSys_enum_ovrdflg
      link override Signal_Override/_ovrdval: Value=KOUTP_APSStaSys_enum_ovrdval
  VVMC_AccCalcuPID_mps2_Inproc : FVT_lib/outp/OverrideAndLimit  SystemSampleTime=-1  VariantActivationTime=update diagram  Latency=0  AutoFrameSizeCalculation=off
      link override Signal_Limit/_maxval: Value=KOUTP_AccCalcuPID_mps2_maxval
      link override Signal_Limit/_minval: Value=KOUTP_AccCalcuPID_mps2_minval
      link override Signal_Override/_ovrdflg: Value=KOUTP_AccCalcuPID_mps2_ovrdflg
      link override Signal_Override/_ovrdval: Value=KOUTP_AccCalcuPID_mps2_ovrdval
  VVMC_CCCtrlSta_enum_Inproc : FVT_lib/outp/OverrideAndLimit  SystemSampleTime=-1  VariantActivationTime=update diagram  Latency=0  AutoFrameSizeCalculation=off
      link override Signal_Limit/_maxval: Value=KOUTP_CCCtrlSta_enum_maxval
      link override Signal_Limit/_minval: Value=KOUTP_CCCtrlSta_enum_minval
      link override Signal_Override/_ovrdflg: Value=KOUTP_CCCtrlSta_enum_ovrdflg
      link override Signal_Override/_ovrdval: Value=KOUTP_CCCtrlSta_enum_ovrdval
  VVMC_CCMSASpdWar_flg_Inproc : FVT_lib/outp/OverrideAndLimit  SystemSampleTime=-1  VariantActivationTime=update diagram  Latency=0  AutoFrameSizeCalculation=off
      link override Signal_Limit/_maxval: Value=KOUTP_CCMSASpdWar_flg_maxval
      link override Signal_Limit/_minval: Value=KOUTP_CCMSASpdWar_flg_minval
      link override Signal_Override/_ovrdflg: Value=KOUTP_CCMSASpdWar_flg_ovrdflg
      link override Signal_Override/_ovrdval: Value=KOUTP_CCMSASpdWar_flg_ovrdval
  VVMC_DISCReqAcc_mps2_Inproc : FVT_lib/outp/OverrideAndLimit  SystemSampleTime=-1  VariantActivationTime=update diagram  Latency=0  AutoFrameSizeCalculation=off
      link override Signal_Limit/_maxval: Value=KOUTP_DISCReqAcc_mps2_maxval
      link override Signal_Limit/_minval: Value=KOUTP_DISCReqAcc_mps2_minval
      link override Signal_Override/_ovrdflg: Value=KOUTP_DISCReqAcc_mps2_ovrdflg
      link override Signal_Override/_ovrdval: Value=KOUTP_DISCReqAcc_mps2_ovrdval
  VVMC_FCMACCmode_enum_Inproc : FVT_lib/outp/OverrideAndLimit  SystemSampleTime=-1  VariantActivationTime=update diagram  Latency=0  AutoFrameSizeCalculation=off
      link override Signal_Limit/_maxval: Value=KOUTP_FCMACCmode_enum_maxval
      link override Signal_Limit/_minval: Value=KOUTP_FCMACCmode_enum_minval
      link override Signal_Override/_ovrdflg: Value=KOUTP_FCMACCmode_enum_ovrdflg
      link override Signal_Override/_ovrdval: Value=KOUTP_FCMACCmode_enum_ovrdval
  VVMC_FCMLDWFault_flg_Inproc : FVT_lib/outp/OverrideAndLimit  SystemSampleTime=-1  VariantActivationTime=update diagram  Latency=0  AutoFrameSizeCalculation=off
      link override Signal_Limit/_maxval: Value=KOUTP_FCMLDWFault_flg_maxval
      link override Signal_Limit/_minval: Value=KOUTP_FCMLDWFault_flg_minval
      link override Signal_Override/_ovrdflg: Value=KOUTP_FCMLDWFault_flg_ovrdflg
      link override Signal_Override/_ovrdval: Value=KOUTP_FCMLDWFault_flg_ovrdval
  VVMC_FCMLDWRequest_enum_Inproc : FVT_lib/outp/OverrideAndLimit  SystemSampleTime=-1  VariantActivationTime=update diagram  Latency=0  AutoFrameSizeCalculation=off
      link override Signal_Limit/_maxval: Value=KOUTP_FCMLDWRequest_enum_maxval
      link override Signal_Limit/_minval: Value=KOUTP_FCMLDWRequest_enum_minval
      link override Signal_Override/_ovrdflg: Value=KOUTP_FCMLDWRequest_enum_ovrdflg
      link override Signal_Override/_ovrdval: Value=KOUTP_FCMLDWRequest_enum_ovrdval
  VVMC_FeatArbitrFinal_enum_Inproc : FVT_lib/outp/OverrideAndLimit  SystemSampleTime=-1  VariantActivationTime=update diagram  Latency=0  AutoFrameSizeCalculation=off
      link override Signal_Limit/_maxval: Value=KOUTP_FeatArbitrFinal_enum_maxval
      link override Signal_Limit/_minval: Value=KOUTP_FeatArbitrFinal_enum_minval
      link override Signal_Override/_ovrdflg: Value=KOUTP_FeatArbitrFinal_enum_ovrdflg
      link override Signal_Override/_ovrdval: Value=KOUTP_FeatArbitrFinal_enum_ovrdval
  VVMC_FeatArbitrSta_enum_Inproc : FVT_lib/outp/OverrideAndLimit  SystemSampleTime=-1  VariantActivationTime=update diagram  Latency=0  AutoFrameSizeCalculation=off
      link override Signal_Limit/_maxval: Value=KOUTP_FeatArbitrSta_enum_maxval
      link override Signal_Limit/_minval: Value=KOUTP_FeatArbitrSta_enum_minval
      link override Signal_Override/_ovrdflg: Value=KOUTP_FeatArbitrSta_enum_ovrdflg
      link override Signal_Override/_ovrdval: Value=KOUTP_FeatArbitrSta_enum_ovrdval
  VVMC_FeatReqSpd_kph_Inproc : FVT_lib/outp/OverrideAndLimit  SystemSampleTime=-1  VariantActivationTime=update diagram  Latency=0  AutoFrameSizeCalculation=off
      link override Signal_Limit/_maxval: Value=KOUTP_FeatReqSpd_kph_maxval
      link override Signal_Limit/_minval: Value=KOUTP_FeatReqSpd_kph_minval
      link override Signal_Override/_ovrdflg: Value=KOUTP_FeatReqSpd_kph_ovrdflg
      link override Signal_Override/_ovrdval: Value=KOUTP_FeatReqSpd_kph_ovrdval
  VVMC_FeatSetSpdFinal_raw32_Inproc : FVT_lib/outp/OverrideAndLimit  SystemSampleTime=-1  VariantActivationTime=update diagram  Latency=0  AutoFrameSizeCalculation=off
      link override Signal_Limit/_maxval: Value=KOUTP_FeatSetSpdFinal_raw32_maxval
      link override Signal_Limit/_minval: Value=KOUTP_FeatSetSpdFinal_raw32_minval
      link override Signal_Override/_ovrdflg: Value=KOUTP_FeatSetSpdFinal_raw32_ovrdflg
      link override Signal_Override/_ovrdval: Value=KOUTP_FeatSetSpdFinal_raw32_ovrdval
  VVMC_ForceLowBeam_enum_Inproc : FVT_lib/outp/OverrideAndLimit  SystemSampleTime=-1  VariantActivationTime=update diagram  Latency=0  AutoFrameSizeCalculation=off
      link override Signal_Limit/_maxval: Value=KOUTP_ForceLowBeam_enum_maxval
      link override Signal_Limit/_minval: Value=KOUTP_ForceLowBeam_enum_minval
      link override Signal_Override/_ovrdflg: Value=KOUTP_ForceLowBeam_enum_ovrdflg
      link override Signal_Override/_ovrdval: Value=KOUTP_ForceLowBeam_enum_ovrdval
  VVMC_FrontRearSlipRatioCtrl_flg_Inproc : FVT_lib/outp/OverrideAndLimit  SystemSampleTime=-1  VariantActivationTime=update diagram  Latency=0  AutoFrameSizeCalculation=off
      link override Signal_Limit/_maxval: Value=KOUTP_FrontRearSlipRatioCtrl_flg_maxval
      link override Signal_Limit/_minval: Value=KOUTP_FrontRearSlipRatioCtrl_flg_minval
      link override Signal_Override/_ovrdflg: Value=KOUTP_FrontRearSlipRatioCtrl_flg_ovrdflg
      link override Signal_Override/_ovrdval: Value=KOUTP_FrontRearSlipRatioCtrl_flg_ovrdval
  VVMC_HazardWarningReq_flg_Inproc : FVT_lib/outp/OverrideAndLimit  SystemSampleTime=-1  VariantActivationTime=update diagram  Latency=0  AutoFrameSizeCalculation=off
      link override Signal_Limit/_maxval: Value=KOUTP_HazardWarningReq_flg_maxval
      link override Signal_Limit/_minval: Value=KOUTP_HazardWarningReq_flg_minval
      link override Signal_Override/_ovrdflg: Value=KOUTP_HazardWarningReq_flg_ovrdflg
      link override Signal_Override/_ovrdval: Value=KOUTP_HazardWarningReq_flg_ovrdval
  VVMC_IMUEnaCmd_flg_Inproc : FVT_lib/outp/OverrideAndLimit  SystemSampleTime=-1  VariantActivationTime=update diagram  Latency=0  AutoFrameSizeCalculation=off
      link override Signal_Limit/_maxval: Value=KOUTP_IMUEnaCmd_flg_maxval
      link override Signal_Limit/_minval: Value=KOUTP_IMUEnaCmd_flg_minval
      link override Signal_Override/_ovrdflg: Value=KOUTP_IMUEnaCmd_flg_ovrdflg
      link override Signal_Override/_ovrdval: Value=KOUTP_IMUEnaCmd_flg_ovrdval
  VVMC_ISOAccLimit_mps2_Inproc : FVT_lib/outp/OverrideAndLimit  SystemSampleTime=-1  VariantActivationTime=update diagram  Latency=0  AutoFrameSizeCalculation=off
      link override Signal_Limit/_maxval: Value=KOUTP_ISOAccLimit_mps2_maxval
      link override Signal_Limit/_minval: Value=KOUTP_ISOAccLimit_mps2_minval
      link override Signal_Override/_ovrdflg: Value=KOUTP_ISOAccLimit_mps2_ovrdflg
      link override Signal_Override/_ovrdval: Value=KOUTP_ISOAccLimit_mps2_ovrdval
  VVMC_ISODecLimit_mps2_Inproc : FVT_lib/outp/OverrideAndLimit  SystemSampleTime=-1  VariantActivationTime=update diagram  Latency=0  AutoFrameSizeCalculation=off
      link override Signal_Limit/_maxval: Value=KOUTP_ISODecLimit_mps2_maxval
      link override Signal_Limit/_minval: Value=KOUTP_ISODecLimit_mps2_minval
      link override Signal_Override/_ovrdflg: Value=KOUTP_ISODecLimit_mps2_ovrdflg
      link override Signal_Override/_ovrdval: Value=KOUTP_ISODecLimit_mps2_ovrdval
  VVMC_ISOJerkLimit_mps3_Inproc : FVT_lib/outp/OverrideAndLimit  SystemSampleTime=-1  VariantActivationTime=update diagram  Latency=0  AutoFrameSizeCalculation=off
      link override Signal_Limit/_maxval: Value=KOUTP_ISOJerkLimit_mps3_maxval
      link override Signal_Limit/_minval: Value=KOUTP_ISOJerkLimit_mps3_minval
      link override Signal_Override/_ovrdflg: Value=KOUTP_ISOJerkLimit_mps3_ovrdflg
      link override Signal_Override/_ovrdval: Value=KOUTP_ISOJerkLimit_mps3_ovrdval
  VVMC_JerkPCT_pct_Inproc : FVT_lib/outp/OverrideAndLimit  SystemSampleTime=-1  VariantActivationTime=update diagram  Latency=0  AutoFrameSizeCalculation=off
      link override Signal_Limit/_maxval: Value=KOUTP_JerkPCT_pct_maxval
      link override Signal_Limit/_minval: Value=KOUTP_JerkPCT_pct_minval
      link override Signal_Override/_ovrdflg: Value=KOUTP_JerkPCT_pct_ovrdflg
      link override Signal_Override/_ovrdval: Value=KOUTP_JerkPCT_pct_ovrdval
  VVMC_LKAHODDisplayWarning_flg_Inproc : FVT_lib/outp/OverrideAndLimit  SystemSampleTime=-1  VariantActivationTime=update diagram  Latency=0  AutoFrameSizeCalculation=off
      link override Signal_Limit/_maxval: Value=KOUTP_LKAHODDisplayWarning_flg_maxval
      link override Signal_Limit/_minval: Value=KOUTP_LKAHODDisplayWarning_flg_minval
      link override Signal_Override/_ovrdflg: Value=KOUTP_LKAHODDisplayWarning_flg_ovrdflg
      link override Signal_Override/_ovrdval: Value=KOUTP_LKAHODDisplayWarning_flg_ovrdval
  VVMC_LKAHODSoundWarning_flg_Inproc : FVT_lib/outp/OverrideAndLimit  SystemSampleTime=-1  VariantActivationTime=update diagram  Latency=0  AutoFrameSizeCalculation=off
      link override Signal_Limit/_maxval: Value=KOUTP_LKAHODSoundWarning_flg_maxval
      link override Signal_Limit/_minval: Value=KOUTP_LKAHODSoundWarning_flg_minval
      link override Signal_Override/_ovrdflg: Value=KOUTP_LKAHODSoundWarning_flg_ovrdflg
      link override Signal_Override/_ovrdval: Value=KOUTP_LKAHODSoundWarning_flg_ovrdval
  VVMC_LKAStrToqReq_Nm_Inproc : FVT_lib/outp/OverrideAndLimit  SystemSampleTime=-1  VariantActivationTime=update diagram  Latency=0  AutoFrameSizeCalculation=off
      link override Signal_Limit/_maxval: Value=KOUTP_LKAStrToqReq_Nm_maxval
      link override Signal_Limit/_minval: Value=KOUTP_LKAStrToqReq_Nm_minval
      link override Signal_Override/_ovrdflg: Value=KOUTP_LKAStrToqReq_Nm_ovrdflg
      link override Signal_Override/_ovrdval: Value=KOUTP_LKAStrToqReq_Nm_ovrdval
  VVMC_LKATOIAct_enum_Inproc : FVT_lib/outp/OverrideAndLimit  SystemSampleTime=-1  VariantActivationTime=update diagram  Latency=0  AutoFrameSizeCalculation=off
      link override Signal_Limit/_maxval: Value=KOUTP_LKATOIAct_enum_maxval
      link override Signal_Limit/_minval: Value=KOUTP_LKATOIAct_enum_minval
      link override Signal_Override/_ovrdflg: Value=KOUTP_LKATOIAct_enum_ovrdflg
      link override Signal_Override/_ovrdval: Value=KOUTP_LKATOIAct_enum_ovrdval
  VVMC_LKATOIFault_flg_Inproc : FVT_lib/outp/OverrideAndLimit  SystemSampleTime=-1  VariantActivationTime=update diagram  Latency=0  AutoFrameSizeCalculation=off
      link override Signal_Limit/_maxval: Value=KOUTP_LKATOIFault_flg_maxval
      link override Signal_Limit/_minval: Value=KOUTP_LKATOIFault_flg_minval
      link override Signal_Override/_ovrdflg: Value=KOUTP_LKATOIFault_flg_ovrdflg
      link override Signal_Override/_ovrdval: Value=KOUTP_LKATOIFault_flg_ovrdval
  VVMC_LVDAACCStatusInformation_flg_Inproc : FVT_lib/outp/OverrideAndLimit  SystemSampleTime=-1  VariantActivationTime=update diagram  Latency=0  AutoFrameSizeCalculation=off
      link override Signal_Limit/_maxval: Value=KOUTP_LVDAACCStatusInformation_flg_maxval
      link override Signal_Limit/_minval: Value=KOUTP_LVDAACCStatusInformation_flg_minval
      link override Signal_Override/_ovrdflg: Value=KOUTP_LVDAACCStatusInformation_flg_ovrdflg
      link override Signal_Override/_ovrdval: Value=KOUTP_LVDAACCStatusInformation_flg_ovrdval
  VVMC_LVDADisabled_flg_Inproc : FVT_lib/outp/OverrideAndLimit  SystemSampleTime=-1  VariantActivationTime=update diagram  Latency=0  AutoFrameSizeCalculation=off
      link override Signal_Limit/_maxval: Value=KOUTP_LVDADisabled_flg_maxval
      link override Signal_Limit/_minval: Value=KOUTP_LVDADisabled_flg_minval
      link override Signal_Override/_ovrdflg: Value=KOUTP_LVDADisabled_flg_ovrdflg
      link override Signal_Override/_ovrdval: Value=KOUTP_LVDADisabled_flg_ovrdval
  VVMC_LVDAFailinfo_flg_Inproc : FVT_lib/outp/OverrideAndLimit  SystemSampleTime=-1  VariantActivationTime=update diagram  Latency=0  AutoFrameSizeCalculation=off
      link override Signal_Limit/_maxval: Value=KOUTP_LVDAFailinfo_flg_maxval
      link override Signal_Limit/_minval: Value=KOUTP_LVDAFailinfo_flg_minval
      link override Signal_Override/_ovrdflg: Value=KOUTP_LVDAFailinfo_flg_ovrdflg
      link override Signal_Override/_ovrdval: Value=KOUTP_LVDAFailinfo_flg_ovrdval
  VVMC_LVDAMuteSta_enum_Inproc : FVT_lib/outp/OverrideAndLimit  SystemSampleTime=-1  VariantActivationTime=update diagram  Latency=0  AutoFrameSizeCalculation=off
      link override Signal_Limit/_maxval: Value=KOUTP_LVDAMuteSta_enum_maxval
      link override Signal_Limit/_minval: Value=KOUTP_LVDAMuteSta_enum_minval
      link override Signal_Override/_ovrdflg: Value=KOUTP_LVDAMuteSta_enum_ovrdflg
      link override Signal_Override/_ovrdval: Value=KOUTP_LVDAMuteSta_enum_ovrdval
  VVMC_LVDAWarning_flg_Inproc : FVT_lib/outp/OverrideAndLimit  SystemSampleTime=-1  VariantActivationTime=update diagram  Latency=0  AutoFrameSizeCalculation=off
      link override Signal_Limit/_maxval: Value=KOUTP_LVDAWarning_flg_maxval
      link override Signal_Limit/_minval: Value=KOUTP_LVDAWarning_flg_minval
      link override Signal_Override/_ovrdflg: Value=KOUTP_LVDAWarning_flg_ovrdflg
      link override Signal_Override/_ovrdval: Value=KOUTP_LVDAWarning_flg_ovrdval
  VVMC_LatAccCtrl_flg_Inproc : FVT_lib/outp/OverrideAndLimit  SystemSampleTime=-1  VariantActivationTime=update diagram  Latency=0  AutoFrameSizeCalculation=off
      link override Signal_Limit/_maxval: Value=KOUTP_LatAccCtrl_flg_maxval
      link override Signal_Limit/_minval: Value=KOUTP_LatAccCtrl_flg_minval
      link override Signal_Override/_ovrdflg: Value=KOUTP_LatAccCtrl_flg_ovrdflg
      link override Signal_Override/_ovrdval: Value=KOUTP_LatAccCtrl_flg_ovrdval
  VVMC_LateralCtrl_flg_Inproc : FVT_lib/outp/OverrideAndLimit  SystemSampleTime=-1  VariantActivationTime=update diagram  Latency=0  AutoFrameSizeCalculation=off
      link override Signal_Limit/_maxval: Value=KOUTP_LateralCtrl_flg_maxval
      link override Signal_Limit/_minval: Value=KOUTP_LateralCtrl_flg_minval
      link override Signal_Override/_ovrdflg: Value=KOUTP_LateralCtrl_flg_ovrdflg
      link override Signal_Override/_ovrdval: Value=KOUTP_LateralCtrl_flg_ovrdval
  VVMC_LeftTurnLightReq_flg_Inproc : FVT_lib/outp/OverrideAndLimit  SystemSampleTime=-1  VariantActivationTime=update diagram  Latency=0  AutoFrameSizeCalculation=off
      link override Signal_Limit/_maxval: Value=KOUTP_LeftTurnLightReq_flg_maxval
      link override Signal_Limit/_minval: Value=KOUTP_LeftTurnLightReq_flg_minval
      link override Signal_Override/_ovrdflg: Value=KOUTP_LeftTurnLightReq_flg_ovrdflg
      link override Signal_Override/_ovrdval: Value=KOUTP_LeftTurnLightReq_flg_ovrdval
  VVMC_LimitPCT_pct_Inproc : FVT_lib/outp/OverrideAndLimit  SystemSampleTime=-1  VariantActivationTime=update diagram  Latency=0  AutoFrameSizeCalculation=off
      link override Signal_Limit/_maxval: Value=KOUTP_LimitPCT_pct_maxval
      link override Signal_Limit/_minval: Value=KOUTP_LimitPCT_pct_minval
      link override Signal_Override/_ovrdflg: Value=KOUTP_LimitPCT_pct_ovrdflg
      link override Signal_Override/_ovrdval: Value=KOUTP_LimitPCT_pct_ovrdval
  VVMC_MSACtrlSta_enum_Inproc : FVT_lib/outp/OverrideAndLimit  SystemSampleTime=-1  VariantActivationTime=update diagram  Latency=0  AutoFrameSizeCalculation=off
      link override Signal_Limit/_maxval: Value=KOUTP_MSACtrlSta_enum_maxval
      link override Signal_Limit/_minval: Value=KOUTP_MSACtrlSta_enum_minval
      link override Signal_Override/_ovrdflg: Value=KOUTP_MSACtrlSta_enum_ovrdflg
      link override Signal_Override/_ovrdval: Value=KOUTP_MSACtrlSta_enum_ovrdval
  VVMC_MeterIndSpeed_raw32_Inproc : FVT_lib/outp/OverrideAndLimit  SystemSampleTime=-1  VariantActivationTime=update diagram  Latency=0  AutoFrameSizeCalculation=off
      link override Signal_Limit/_maxval: Value=KOUTP_MeterIndSpeed_raw32_maxval
      link override Signal_Limit/_minval: Value=KOUTP_MeterIndSpeed_raw32_minval
      link override Signal_Override/_ovrdflg: Value=KOUTP_MeterIndSpeed_raw32_ovrdflg
      link override Signal_Override/_ovrdval: Value=KOUTP_MeterIndSpeed_raw32_ovrdval
  VVMC_RearWhlSlipRatioCtrl_flg_Inproc : FVT_lib/outp/OverrideAndLimit  SystemSampleTime=-1  VariantActivationTime=update diagram  Latency=0  AutoFrameSizeCalculation=off
      link override Signal_Limit/_maxval: Value=KOUTP_RearWhlSlipRatioCtrl_flg_maxval
      link override Signal_Limit/_minval: Value=KOUTP_RearWhlSlipRatioCtrl_flg_minval
      link override Signal_Override/_ovrdflg: Value=KOUTP_RearWhlSlipRatioCtrl_flg_ovrdflg
      link override Signal_Override/_ovrdval: Value=KOUTP_RearWhlSlipRatioCtrl_flg_ovrdval
  VVMC_RightTurnLightReq_flg_Inproc : FVT_lib/outp/OverrideAndLimit  SystemSampleTime=-1  VariantActivationTime=update diagram  Latency=0  AutoFrameSizeCalculation=off
      link override Signal_Limit/_maxval: Value=KOUTP_RightTurnLightReq_flg_maxval
      link override Signal_Limit/_minval: Value=KOUTP_RightTurnLightReq_flg_minval
      link override Signal_Override/_ovrdflg: Value=KOUTP_RightTurnLightReq_flg_ovrdflg
      link override Signal_Override/_ovrdval: Value=KOUTP_RightTurnLightReq_flg_ovrdval
  VVMC_SPD2ACCAct_flg_Inproc : FVT_lib/outp/OverrideAndLimit  SystemSampleTime=-1  VariantActivationTime=update diagram  Latency=0  AutoFrameSizeCalculation=off
      link override Signal_Limit/_maxval: Value=KOUTP_SPD2ACCAct_flg_maxval
      link override Signal_Limit/_minval: Value=KOUTP_SPD2ACCAct_flg_minval
      link override Signal_Override/_ovrdflg: Value=KOUTP_SPD2ACCAct_flg_ovrdflg
      link override Signal_Override/_ovrdval: Value=KOUTP_SPD2ACCAct_flg_ovrdval
  VVMC_SafetyCtrl_flg_Inproc : FVT_lib/outp/OverrideAndLimit  SystemSampleTime=-1  VariantActivationTime=update diagram  Latency=0  AutoFrameSizeCalculation=off
      link override Signal_Limit/_maxval: Value=KOUTP_SafetyCtrl_flg_maxval
      link override Signal_Limit/_minval: Value=KOUTP_SafetyCtrl_flg_minval
      link override Signal_Override/_ovrdflg: Value=KOUTP_SafetyCtrl_flg_ovrdflg
      link override Signal_Override/_ovrdval: Value=KOUTP_SafetyCtrl_flg_ovrdval
  VVMC_SingleWhlSlipRatioCtrl_flg_Inproc : FVT_lib/outp/OverrideAndLimit  SystemSampleTime=-1  VariantActivationTime=update diagram  Latency=0  AutoFrameSizeCalculation=off
      link override Signal_Limit/_maxval: Value=KOUTP_SingleWhlSlipRatioCtrl_flg_maxval
      link override Signal_Limit/_minval: Value=KOUTP_SingleWhlSlipRatioCtrl_flg_minval
      link override Signal_Override/_ovrdflg: Value=KOUTP_SingleWhlSlipRatioCtrl_flg_ovrdflg
      link override Signal_Override/_ovrdval: Value=KOUTP_SingleWhlSlipRatioCtrl_flg_ovrdval
  VVMC_TargetType_enum_Inproc : FVT_lib/outp/OverrideAndLimit  SystemSampleTime=-1  VariantActivationTime=update diagram  Latency=0  AutoFrameSizeCalculation=off
      link override Signal_Limit/_maxval: Value=KOUTP_TargetType_enum_maxval
      link override Signal_Limit/_minval: Value=KOUTP_TargetType_enum_minval
      link override Signal_Override/_ovrdflg: Value=KOUTP_TargetType_enum_ovrdflg
      link override Signal_Override/_ovrdval: Value=KOUTP_TargetType_enum_ovrdval
  VVMC_TimeGapCalcu_s_Inproc : FVT_lib/outp/OverrideAndLimit  SystemSampleTime=-1  VariantActivationTime=update diagram  Latency=0  AutoFrameSizeCalculation=off
      link override Signal_Limit/_maxval: Value=KOUTP_TimeGapCalcu_s_maxval
      link override Signal_Limit/_minval: Value=KOUTP_TimeGapCalcu_s_minval
      link override Signal_Override/_ovrdflg: Value=KOUTP_TimeGapCalcu_s_ovrdflg
      link override Signal_Override/_ovrdval: Value=KOUTP_TimeGapCalcu_s_ovrdval
  VVMC_TimeGapLevel_enum_Inproc : FVT_lib/outp/OverrideAndLimit  SystemSampleTime=-1  VariantActivationTime=update diagram  Latency=0  AutoFrameSizeCalculation=off
      link override Signal_Limit/_maxval: Value=KOUTP_TimeGapLevel_enum_maxval
      link override Signal_Limit/_minval: Value=KOUTP_TimeGapLevel_enum_minval
      link override Signal_Override/_ovrdflg: Value=KOUTP_TimeGapLevel_enum_ovrdflg
      link override Signal_Override/_ovrdval: Value=KOUTP_TimeGapLevel_enum_ovrdval
  VVMC_VMCACCCtrlAvail_flg_Inproc : FVT_lib/outp/OverrideAndLimit  SystemSampleTime=-1  VariantActivationTime=update diagram  Latency=0  AutoFrameSizeCalculation=off
      link override Signal_Limit/_maxval: Value=KOUTP_VMCACCCtrlAvail_flg_maxval
      link override Signal_Limit/_minval: Value=KOUTP_VMCACCCtrlAvail_flg_minval
      link override Signal_Override/_ovrdflg: Value=KOUTP_VMCACCCtrlAvail_flg_ovrdflg
      link override Signal_Override/_ovrdval: Value=KOUTP_VMCACCCtrlAvail_flg_ovrdval
  VVMC_VMCAEBCtrlAvail_flg_Inproc : FVT_lib/outp/OverrideAndLimit  SystemSampleTime=-1  VariantActivationTime=update diagram  Latency=0  AutoFrameSizeCalculation=off
      link override Signal_Limit/_maxval: Value=KOUTP_VMCAEBCtrlAvail_flg_maxval
      link override Signal_Limit/_minval: Value=KOUTP_VMCAEBCtrlAvail_flg_minval
      link override Signal_Override/_ovrdflg: Value=KOUTP_VMCAEBCtrlAvail_flg_ovrdflg
      link override Signal_Override/_ovrdval: Value=KOUTP_VMCAEBCtrlAvail_flg_ovrdval
  VVMC_VMCCCCtrlAvail_flg_Inproc : FVT_lib/outp/OverrideAndLimit  SystemSampleTime=-1  VariantActivationTime=update diagram  Latency=0  AutoFrameSizeCalculation=off
      link override Signal_Limit/_maxval: Value=KOUTP_VMCCCCtrlAvail_flg_maxval
      link override Signal_Limit/_minval: Value=KOUTP_VMCCCCtrlAvail_flg_minval
      link override Signal_Override/_ovrdflg: Value=KOUTP_VMCCCCtrlAvail_flg_ovrdflg
      link override Signal_Override/_ovrdval: Value=KOUTP_VMCCCCtrlAvail_flg_ovrdval
  VVMC_VMCMSACtrlAvail_flg_Inproc : FVT_lib/outp/OverrideAndLimit  SystemSampleTime=-1  VariantActivationTime=update diagram  Latency=0  AutoFrameSizeCalculation=off
      link override Signal_Limit/_maxval: Value=KOUTP_VMCMSACtrlAvail_flg_maxval
      link override Signal_Limit/_minval: Value=KOUTP_VMCMSACtrlAvail_flg_minval
      link override Signal_Override/_ovrdflg: Value=KOUTP_VMCMSACtrlAvail_flg_ovrdflg
      link override Signal_Override/_ovrdval: Value=KOUTP_VMCMSACtrlAvail_flg_ovrdval
  VVMC_VehicleSpeed_kph_Inproc : FVT_lib/outp/OverrideAndLimit  SystemSampleTime=-1  VariantActivationTime=update diagram  Latency=0  AutoFrameSizeCalculation=off
      link override Signal_Limit/_maxval: Value=KOUTP_VehicleSpeed_kph_maxval
      link override Signal_Limit/_minval: Value=KOUTP_VehicleSpeed_kph_minval
      link override Signal_Override/_ovrdflg: Value=KOUTP_VehicleSpeed_kph_ovrdflg
      link override Signal_Override/_ovrdval: Value=KOUTP_VehicleSpeed_kph_ovrdval
  VVMC_VehicleSpeed_mph_Inproc : FVT_lib/outp/OverrideAndLimit  SystemSampleTime=-1  VariantActivationTime=update diagram  Latency=0  AutoFrameSizeCalculation=off
      link override Signal_Limit/_maxval: Value=KOUTP_VehicleSpeed_mph_maxval
      link override Signal_Limit/_minval: Value=KOUTP_VehicleSpeed_mph_minval
      link override Signal_Override/_ovrdflg: Value=KOUTP_VehicleSpeed_mph_ovrdflg
      link override Signal_Override/_ovrdval: Value=KOUTP_VehicleSpeed_mph_ovrdval
  VOUTP_HVTHCMSysAvail_enum : Outport
  VOUTP_LVBattVoltSta_enum : Outport  Port=2
  VOUTP_VehHVPwrAvail4THCM_W : Outport  Port=3
  VOUTP_EHPSEnDem_enum : Outport  Port=4
  VOUTP_CACPresWarnSta_flg : Outport  Port=5
  VOUTP_CACTempWarnSta_flg : Outport  Port=6
  VOUTP_EACEnDem_enum : Outport  Port=7
  VOUTP_VehSpeedToAPM_kph : Outport  Port=8
  VOUTP_VehSpeedTimeOut_flg : Outport  Port=9
  VOUTP_FSOffSw_enum : Outport  Port=10
  VOUTP_FSOffSwTimeOut_flg : Outport  Port=11
  VOUTP_ChrgPlugSta_enum : Outport  Port=12
  VOUTP_PASDRMR_cm : Outport  Port=13
  VOUTP_PASDRML_cm : Outport  Port=14
  VOUTP_PASDRCR_cm : Outport  Port=15
  VOUTP_PASDRCL_cm : Outport  Port=16
  VOUTP_PASDFMR_cm : Outport  Port=17
  VOUTP_PASDFML_cm : Outport  Port=18
  VOUTP_PASDFCR_cm : Outport  Port=19
  VOUTP_PASDFCL_cm : Outport  Port=20
  VOUTP_APSDRLR_cm : Outport  Port=21
  VOUTP_APSDRLL_cm : Outport  Port=22
  VOUTP_APSDFLR_cm : Outport  Port=23
  VOUTP_APSDFLL_cm : Outport  Port=24
  VOUTP_PASAFCL_enum : Outport  Port=25
  VOUTP_PASARMR_enum : Outport  Port=26
  VOUTP_PASARML_enum : Outport  Port=27
  VOUTP_PASARCR_enum : Outport  Port=28
  VOUTP_PASARCL_enum : Outport  Port=29
  VOUTP_PASAFMR_enum : Outport  Port=30
  VOUTP_PASAFML_enum : Outport  Port=31
  VOUTP_PASAFCR_enum : Outport  Port=32
  VOUTP_USSStaRMR_flg : Outport  Port=33
  VOUTP_USSStaRML_flg : Outport  Port=34
  VOUTP_USSStaRLR_flg : Outport  Port=35
  VOUTP_USSStaRLL_flg : Outport  Port=36
  VOUTP_USSStaRCR_flg : Outport  Port=37
  VOUTP_USSStaRCL_flg : Outport  Port=38
  VOUTP_USSStaFMR_flg : Outport  Port=39
  VOUTP_USSStaFML_flg : Outport  Port=40
  VOUTP_USSStaFLR_flg : Outport  Port=41
  VOUTP_USSStaFLL_flg : Outport  Port=42
  VOUTP_USSStaFCR_flg : Outport  Port=43
  VOUTP_USSStaFCL_flg : Outport  Port=44
  VOUTP_Chime_enum : Outport  Port=45
  VOUTP_SNSRLayout_enum : Outport  Port=46
  VOUTP_StaFSya_flg : Outport  Port=47
  VOUTP_ModOperation_enum : Outport  Port=48
  VOUTP_BrkPedalPosToAPM_pct : Outport  Port=49
  VOUTP_BrkPedalPosTimeOut_flg : Outport  Port=50
  VOUTP_LFRawWhlSpeed_kph : Outport  Port=51
  VOUTP_LFRawWhlSpeedTimeOut_flg : Outport  Port=52
  VOUTP_RFRawWhlSpeed_kph : Outport  Port=53
  VOUTP_RFRawWhlSpeedTimeOut_flg : Outport  Port=54
  VOUTP_LRRawWhlSpeed_kph : Outport  Port=55
  VOUTP_LRRawWhlSpeedTimeOut_flg : Outport  Port=56
  VOUTP_RRRawWhlSpeed_kph : Outport  Port=57
  VOUTP_RRRawWhlSpeedTimeOut_flg : Outport  Port=58
  VOUTP_LFRawWhlSpeedV_flg : Outport  Port=59
  VOUTP_LFRawWhlSpeedVTimeOut_flg : Outport  Port=60
  VOUTP_RFRawWhlSpeedV_flg : Outport  Port=61
  VOUTP_RFRawWhlSpeedVTimeOut_flg : Outport  Port=62
  VOUTP_LRRawWhlSpeedV_flg : Outport  Port=63
  VOUTP_LRRawWhlSpeedVTimeOut_flg : Outport  Port=64
  VOUTP_RRRawWhlSpeedV_flg : Outport  Port=65
  VOUTP_RRRawWhlSpeedVTimeOut_flg : Outport  Port=66
  VOUTP_LFWhlRotDir_enum : Outport  Port=67
  VOUTP_LFWhlRotDirTimeOut_flg : Outport  Port=68
  VOUTP_RFWhlRotDir_enum : Outport  Port=69
  VOUTP_RFWhlRotDirTimeOut_flg : Outport  Port=70
  VOUTP_LRWhlRotDir_enum : Outport  Port=71
  VOUTP_LRWhlRotDirTimeOut_flg : Outport  Port=72
  VOUTP_RRWhlRotDir_enum : Outport  Port=73
  VOUTP_RRWhlRotDirTimeOut_flg : Outport  Port=74
  VOUTP_LFPulseCountV_flg : Outport  Port=75
  VOUTP_LFPulseCountVTimeOut_flg : Outport  Port=76
  VOUTP_RFPulseCountV_flg : Outport  Port=77
  VOUTP_RFPulseCountVTimeOut_flg : Outport  Port=78
  VOUTP_LRPulseCountV_flg : Outport  Port=79
  VOUTP_LRPulseCountVTimeOut_flg : Outport  Port=80
  VOUTP_RRPulseCountV_flg : Outport  Port=81
  VOUTP_RRPulseCountVTimeOut_flg : Outport  Port=82
  VOUTP_LFPulseCount_enum : Outport  Port=83
  VOUTP_LFPulseCountTimeOut_flg : Outport  Port=84
  VOUTP_RFPulseCount_enum : Outport  Port=85
  VOUTP_RFPulseCountTimeOut_flg : Outport  Port=86
  VOUTP_LRPulseCount_enum : Outport  Port=87
  VOUTP_LRPulseCountTimeOut_flg : Outport  Port=88
  VOUTP_RRPulseCount_enum : Outport  Port=89
  VOUTP_RRPulseCountTimeOut_flg : Outport  Port=90
  VOUTP_ShifterHandleCmd_enum : Outport  Port=91
  VOUTP_ShifterHandleCmdTimeOut_flg : Outport  Port=92
  VOUTP_DriIntend_enum : Outport  Port=93
  VOUTP_DriIntendTimeOut_flg : Outport  Port=94
  VOUTP_EPSAOIControl_enum : Outport  Port=95
  VOUTP_EPSAOIControlTimeOut_flg : Outport  Port=96
  VOUTP_SASAngle_Deg : Outport  Port=97
  VOUTP_SASAngleTimeOut_flg : Outport  Port=98
  VOUTP_SASSpeed_degps : Outport  Port=99
  VOUTP_SASSpeedTimeOut_flg : Outport  Port=100
  VOUTP_SASSpeedValid_flg : Outport  Port=101
  VOUTP_SASSpeedValidTimeOut_flg : Outport  Port=102
  VOUTP_SASCAL_flg : Outport  Port=103
  VOUTP_SASCALTimeOut_flg : Outport  Port=104
  VOUTP_SASV_flg : Outport  Port=105
  VOUTP_SASVTimeOut_flg : Outport  Port=106
  VOUTP_GRADE_Deg : Outport  Port=107
  VOUTP_GRADETimeOut_flg : Outport  Port=108
  VOUTP_YawRate_degps : Outport  Port=109
  VOUTP_YawRateTimeOut_flg : Outport  Port=110
  VOUTP_LatAccel_Gps : Outport  Port=111
  VOUTP_LatAccelTimeOut_flg : Outport  Port=112
  VOUTP_LongAccel_Gps : Outport  Port=113
  VOUTP_LongAccelTimeOut_flg : Outport  Port=114
  VOUTP_MCPressure_bar : Outport  Port=115
  VOUTP_MCPressureTimeOut_flg : Outport  Port=116
  VOUTP_YawRateV_flg : Outport  Port=117
  VOUTP_YawRateVTimeOut_flg : Outport  Port=118
  VOUTP_LatAccelV_flg : Outport  Port=119
  VOUTP_LatAccelVTimeOut_flg : Outport  Port=120
  VOUTP_LongAccelV_flg : Outport  Port=121
  VOUTP_LongAccelVTimeOut_flg : Outport  Port=122
  VOUTP_MCPressureV_bar : Outport  Port=123
  VOUTP_MCPressureVTimeOut_flg : Outport  Port=124
  VOUTP_BrkSwSta_flg : Outport  Port=125
  VOUTP_BrkSwStaTimeOut_flg : Outport  Port=126
  VOUTP_BrkSwV_flg : Outport  Port=127
  VOUTP_BrkSwVTimeOut_flg : Outport  Port=128
  VOUTP_ESCStandstill_flg : Outport  Port=129
  VOUTP_ESCStandstillTimeOut_flg : Outport  Port=130
  VOUTP_ESCAPSSta_enum : Outport  Port=131
  VOUTP_ESCAPSStaTimeOut_flg : Outport  Port=132
  VOUTP_EPBExtReleaseAvail_flg : Outport  Port=133
  VOUTP_EPBExtReleaseAvailTimeOut_flg : Outport  Port=134
  VOUTP_EPBExtApplyAvail_flg : Outport  Port=135
  VOUTP_EPBExtApplyAvailTimeOut_flg : Outport  Port=136
  VOUTP_EPBErrSta_enum : Outport  Port=137
  VOUTP_EPBErrStaTimeOut_flg : Outport  Port=138
  VOUTP_EPBSta_enum : Outport  Port=139
  VOUTP_EPBStaTimeOut_flg : Outport  Port=140
  VOUTP_AVMparkingcancel_enum : Outport  Port=141
  VOUTP_AVMparkingcancelTimeOut_flg : Outport  Port=142
  VOUTP_AVMparkingexcute_enum : Outport  Port=143
  VOUTP_AVMparkingexcuteTimeOut_flg : Outport  Port=144
  VOUTP_AVMParkingmode_enum : Outport  Port=145
  VOUTP_AVMParkingmodeTimeOut_flg : Outport  Port=146
  VOUTP_AVMErrSTA_flg : Outport  Port=147
  VOUTP_AVMErrSTATimeOut_flg : Outport  Port=148
  VOUTP_IVIStatus_flg : Outport  Port=149
  VOUTP_IVIStatusTimeOut_flg : Outport  Port=150
  VOUTP_CAASSw_enum : Outport  Port=151
  VOUTP_CAASSwTimeOut_flg : Outport  Port=152
  VOUTP_IVIScreen_enum : Outport  Port=153
  VOUTP_IVIScreenTimeOut_flg : Outport  Port=154
  VOUTP_ABSActiveToAPM_flg : Outport  Port=155
  VOUTP_ABSActiveTimeOut_flg : Outport  Port=156
  VOUTP_TCSActiveToAPM_flg : Outport  Port=157
  VOUTP_TCSActiveTimeOut_flg : Outport  Port=158
  VOUTP_DriverSeatBeltCmd_flg : Outport  Port=159
  VOUTP_DriverSeatBeltCmdTimeOut_flg : Outport  Port=160
  VOUTP_APSProgressPCT_pct : Outport  Port=161
  VOUTP_APSRQDisplay_enum : Outport  Port=162
  VOUTP_APSSWVer_enum : Outport  Port=163
  VOUTP_APSHWVer_enum : Outport  Port=164
  VOUTP_APSExitCondition_enum : Outport  Port=165
  VOUTP_APSAngleTarget_Deg : Outport  Port=166
  VOUTP_APSVRqEPASCtrl_flg : Outport  Port=167
  VOUTP_APSRqEPASCtrl_flg : Outport  Port=168
  VOUTP_CAASSta_enum : Outport  Port=169
  VOUTP_HornCtrl_flg : Outport  Port=170
  VOUTP_FRHaltBrakeSta_enum : Outport  Port=171
  VOUTP_FRDisIntEmCmd_flg : Outport  Port=172
  VOUTP_FROpenClosePBCmd_enum : Outport  Port=173
  VOUTP_DoorStaSta_enum : Outport  Port=174
  VOUTP_BrakeLamp_flg : Outport  Port=175
  VOUTP_LDRL_flg : Outport  Port=176
  VOUTP_RDRL_flg : Outport  Port=177
  VOUTP_ReverseLamp_flg : Outport  Port=178
  VOUTP_RrFogLamp_flg : Outport  Port=179
  VOUTP_HBeam_flg : Outport  Port=180
  VOUTP_LBeam_flg : Outport  Port=181
  VOUTP_PosLamp_flg : Outport  Port=182
  VOUTP_HazardSW_flg : Outport  Port=183
  VOUTP_LTurnLP_flg : Outport  Port=184
  VOUTP_RTurnLP_flg : Outport  Port=185
  VOUTP_LSMLPCmd_flg : Outport  Port=186
  VOUTP_RSMLPCmd_flg : Outport  Port=187
  VOUTP_TurnLpLActiveCmd_flg : Outport  Port=188
  VOUTP_TurnLpRActiveCmd_flg : Outport  Port=189
  VOUTP_BBuzzerCmd_flg : Outport  Port=190
  VOUTP_FrWiperL_flg : Outport  Port=191
  VOUTP_FrWiperH_flg : Outport  Port=192
  VOUTP_WasherCtrl_enum : Outport  Port=193
  VOUTP_RrRmLampBrightCmd_enum : Outport  Port=194
  VOUTP_WelcomeDemoSta_flg : Outport  Port=195
  VOUTP_FrAtmoLampCmd_flg : Outport  Port=196
  VOUTP_RrAtmoLampCmd_flg : Outport  Port=197
  VOUTP_TgateHDSWLSta_flg : Outport  Port=198
  VOUTP_TgateHDSWRSta_flg : Outport  Port=199
  VOUTP_TgateSWLSta_flg : Outport  Port=200
  VOUTP_TgateSWRSta_flg : Outport  Port=201
  VOUTP_LTgateRelCmd_flg : Outport  Port=202
  VOUTP_RTgateRelCmd_flg : Outport  Port=203
  VOUTP_FDDoorOpen_enum : Outport  Port=204
  VOUTP_FDDoorstate_enum : Outport  Port=205
  VOUTP_ActAPSPosn_pct : Outport  Port=206
  VOUTP_EAPS1MIN_pct : Outport  Port=207
  VOUTP_EAPS2MIN_pct : Outport  Port=208
  VOUTP_DKCTimeSN_cnt : Outport  Port=209
  VOUTP_DKCAuthSta_enum : Outport  Port=210
  VOUTP_DISCTurn_flg : Outport  Port=211
  VOUTP_DISCTargetSpd_kph : Outport  Port=212
  VOUTP_DISCSta_enum : Outport  Port=213
  VOUTP_DISCButtSta_flg : Outport  Port=214
  VOUTP_AllCANTxReq_flg : Outport  Port=215
  VOUTP_NMmTxReq_flg : Outport  Port=216
  VOUTP_Awake_enum : Outport  Port=217
  VOUTP_CSB_flg : Outport  Port=218
  VOUTP_ErrorState_enum : Outport  Port=219
  VOUTP_NodeID_enum : Outport  Port=220
  VOUTP_PNI_flg : Outport  Port=221
  VOUTP_RptMsgReq_flg : Outport  Port=222
  VOUTP_WakeUp_enum : Outport  Port=223
  VOUTP_ActiveWU_flg : Outport  Port=224
  VOUTP_SysNMmSta_enum : Outport  Port=225
  VOUTP_NetworkReq_flg : Outport  Port=226
  VOUTP_PowerUpState_enum : Outport  Port=227
  VOUTP_PowerDownState_enum : Outport  Port=228
  VOUTP_PowerUpFault_enum : Outport  Port=229
  VOUTP_PowerDownFault_enum : Outport  Port=230
  VOUTP_ActiveDischargeReq_flg : Outport  Port=231
  VOUTP_DCDCEnaReq_flg : Outport  Port=232
  VOUTP_DCDCVoltSetpoint_V : Outport  Port=233
  VOUTP_HVBatCnctReq_flg : Outport  Port=234
  VOUTP_HVSysReadyToCharge_enum : Outport  Port=235
  VOUTP_PowerSta_enum : Outport  Port=236
  VOUTP_LVPwrSta_flg : Outport  Port=237
  VOUTP_HVPwrSta_flg : Outport  Port=238
  VOUTP_SysPowerMode_enum : Outport  Port=239
  VOUTP_FrMCUEnaReq_flg : Outport  Port=240
  VOUTP_RrMCUEnaReq_flg : Outport  Port=241
  VOUTP_DrivetrainSelect_enum : Outport  Port=242
  VOUTP_DrSeatSta_enum : Outport  Port=243
  VOUTP_PwrStaSelect_enum : Outport  Port=244
  VOUTP_PwrStaConstraint_enum : Outport  Port=245
  VOUTP_TCountSta_enum : Outport  Port=246
  VOUTP_PwrUpReq_enum : Outport  Port=247
  VOUTP_PwrDownReq_enum : Outport  Port=248
  VOUTP_LowSOCWarn_enum : Outport  Port=249
  VOUTP_ReVehThdChkSta_enum : Outport  Port=250
  VOUTP_LVSysErrPwrOutErr_flg : Outport  Port=251
  VOUTP_EvccAplusPwrUpReq_flg : Outport  Port=252
  VOUTP_PwrStaONTOPopReq_flg : Outport  Port=253
  VOUTP_IVIPwrStaONTOPopT_s : Outport  Port=254
  VOUTP_LVChrgHoldTtimer_s : Outport  Port=255
  VOUTP_LVBattChrgTimeCnt_s : Outport  Port=256
  VOUTP_SilentChkAllowSleep_flg : Outport  Port=257
  VOUTP_TimerAllowSleep_flg : Outport  Port=258
  VOUTP_FDADC12VDetAvg_mV : Outport  Port=259
  VOUTP_PMMAllowECUSleep_flg : Outport  Port=260
  VOUTP_LVSilentChrgSta_enum : Outport  Port=261
  VOUTP_LVSilentChrgReq_flg : Outport  Port=262
  VOUTP_LVSilentChrgLv_enum : Outport  Port=263
  VOUTP_CtrlFrPwrStbA1P_flg : Outport  Port=264
  VOUTP_CtrlFrRC1_flg : Outport  Port=265
  VOUTP_CtrlFrBMSCCUCIR_flg : Outport  Port=266
  VOUTP_CtrlFrEDUINVERTER_flg : Outport  Port=267
  VOUTP_HWResetSta_enum : Outport  Port=268
  VOUTP_CtrlDrPwrStbA2_flg : Outport  Port=269
  VOUTP_PwrStaTOSta_enum : Outport  Port=270
  VOUTP_DCDCRlyDem_enum : Outport  Port=271
  VOUTP_EACRlyDem_enum : Outport  Port=272
  VOUTP_EHPSRlyDem_enum : Outport  Port=273
  VOUTP_DCDCEnDem_enum : Outport  Port=274
  VOUTP_Vehspeed_kph : Outport  Port=275
  VOUTP_SCPBrkSwSta_flg : Outport  Port=276
  VOUTP_AmberWnlmpSta_flg : Outport  Port=277
  VOUTP_ABSWnlmpSta_flg : Outport  Port=278
  VOUTP_HSAFailed_flg : Outport  Port=279
  VOUTP_MeterIndVehSpeed_kph : Outport  Port=280
  VOUTP_ABSFailed_flg : Outport  Port=281
  VOUTP_ABSActive_flg : Outport  Port=282
  VOUTP_HSAActive_flg : Outport  Port=283
  VOUTP_RedWnlmpSta_flg : Outport  Port=284
  VOUTP_BrkPedalPos_pct : Outport  Port=285
  VOUTP_OpenStatusOfDoor1_enum : Outport  Port=286
  VOUTP_OpenStatusOfDoor2_enum : Outport  Port=287
  VOUTP_SeatBeltSwitch_enum : Outport  Port=288
  VOUTP_triggerBAM_flg : Outport  Port=289
  VOUTP_CFGEM1Ctrl_raw : Outport  Port=290
  VOUTP_CFGEM1BAMTSize_raw : Outport  Port=291
  VOUTP_CFGEM1BAMTNum_raw : Outport  Port=292
  VOUTP_CFGEM1BAMRsv_raw : Outport  Port=293
  VOUTP_CFGEM1BAMPGN_raw : Outport  Port=294
  VOUTP_triggerDT_flg : Outport  Port=295
  VOUTP_DTbyte0_raw : Outport  Port=296
  VOUTP_DTbyte1_raw : Outport  Port=297
  VOUTP_DTbyte2_raw : Outport  Port=298
  VOUTP_DTbyte3_raw : Outport  Port=299
  VOUTP_DTbyte4_raw : Outport  Port=300
  VOUTP_DTbyte5_raw : Outport  Port=301
  VOUTP_DTbyte6_raw : Outport  Port=302
  VOUTP_DTbyte7_raw : Outport  Port=303
  VOUTP_HWVer1_cnt : Outport  Port=304
  VOUTP_HWVer2_cnt : Outport  Port=305
  VOUTP_HWVer3_cnt : Outport  Port=306
  VOUTP_CarModel1_cnt : Outport  Port=307
  VOUTP_CarModel2_cnt : Outport  Port=308
  VOUTP_CarModel3_cnt : Outport  Port=309
  VOUTP_ECU1_cnt : Outport  Port=310
  VOUTP_ECU2_cnt : Outport  Port=311
  VOUTP_Major1_cnt : Outport  Port=312
  VOUTP_Major2_cnt : Outport  Port=313
  VOUTP_Minor1_cnt : Outport  Port=314
  VOUTP_Minor2_cnt : Outport  Port=315
  VOUTP_Patch1_cnt : Outport  Port=316
  VOUTP_Patch2_cnt : Outport  Port=317
  VOUTP_Country1_cnt : Outport  Port=318
  VOUTP_Country2_cnt : Outport  Port=319
  VOUTP_Variation_cnt : Outport  Port=320
  VOUTP_Dash1_cnt : Outport  Port=321
  VOUTP_Change1_cnt : Outport  Port=322
  VOUTP_Change2_cnt : Outport  Port=323
  VOUTP_Dash2_cnt : Outport  Port=324
  VOUTP_SHA1_cnt : Outport  Port=325
  VOUTP_SHA2_cnt : Outport  Port=326
  VOUTP_SHA3_cnt : Outport  Port=327
  VOUTP_SHA4_cnt : Outport  Port=328
  VOUTP_SHA5_cnt : Outport  Port=329
  VOUTP_SHA6_cnt : Outport  Port=330
  VOUTP_SHA7_cnt : Outport  Port=331
  VOUTP_SHA8_cnt : Outport  Port=332
  VOUTP_NvWriteReqRisingEdge_flg : Outport  Port=333
  VOUTP_FdcSlpReqRisingEdge_flg : Outport  Port=334
  VOUTP_FdcSlpTime_sec : Outport  Port=335
  VOUTP_PmicBootReason_enum : Outport  Port=336
  VOUTP_WisrBootReason_raw32 : Outport  Port=337
  VOUTP_AcoreRebootCmdACK_flg : Outport  Port=338
  VOUTP_CurrentNmState_enum : Outport  Port=339
  VOUTP_FDCompCmd_rpm : Outport  Port=340
  VOUTP_FDSOV1Cmd_flg : Outport  Port=341
  VOUTP_FDSOV2Cmd_flg : Outport  Port=342
  VOUTP_FDSOV3Cmd_flg : Outport  Port=343
  VOUTP_FDEXV1Cmd_step : Outport  Port=344
  VOUTP_FDEXV2Cmd_step : Outport  Port=345
  VOUTP_FDSOTXVCmd_flg : Outport  Port=346
  VOUTP_FDFWVCmd_flg : Outport  Port=347
  VOUTP_FDTWVCmd_pct : Outport  Port=348
  VOUTP_FDFrWPTCHeatPwrCmd_W : Outport  Port=349
  VOUTP_CoolgFanActDuty_pct : Outport  Port=350
  VOUTP_FDAGSCmd_enum : Outport  Port=351
  VOUTP_FDEWP1Cmd_enum : Outport  Port=352
  VOUTP_FDEWP2Cmd_enum : Outport  Port=353
  VOUTP_FDEWP3Cmd_enum : Outport  Port=354
  VOUTP_FDFrLeAPTCHeatPwrCmd_W : Outport  Port=355
  VOUTP_FDFrRiAPTCHeatPwrCmd_W : Outport  Port=356
  VOUTP_FDRrAPTCHeatPwrCmd_W : Outport  Port=357
  VOUTP_FDBlowerCmd_pct : Outport  Port=358
  VOUTP_BatteryMode_enum : Outport  Port=359
  VOUTP_EDriveMode_enum : Outport  Port=360
  VOUTP_CabinMode_enum : Outport  Port=361
  VOUTP_CCUACLampSts_flg : Outport  Port=362
  VOUTP_CCUAutoLampSts_flg : Outport  Port=363
  VOUTP_CCUACMaxLampSts_flg : Outport  Port=364
  VOUTP_CCUSyncLampSts_flg : Outport  Port=365
  VOUTP_sigAirIntenZon1St_enum : Outport  Port=366
  VOUTP_sigWindDirZon1St_enum : Outport  Port=367
  VOUTP_sigRecircSt_flg : Outport  Port=368
  VOUTP_sigSetTempZon1St_C : Outport  Port=369
  VOUTP_sigSetTempZon2St_C : Outport  Port=370
  VOUTP_sigClntTHvBattOut_C : Outport  Port=371
  VOUTP_sigCbnSolarLeft_W : Outport  Port=372
  VOUTP_sigClntTHvBattIn_C : Outport  Port=373
  VOUTP_sigCbnSolarRight_W : Outport  Port=374
  VOUTP_sigAmbAirT_C : Outport  Port=375
  VOUTP_sigCbnAirT_C : Outport  Port=376
  VOUTP_ACSubMode_enum : Outport  Port=377
  VOUTP_FDRecyAutoCmd_enum : Outport  Port=378
  VOUTP_ACModeMem_enum : Outport  Port=379
  VOUTP_Face_flg : Outport  Port=380
  VOUTP_Foot_flg : Outport  Port=381
  VOUTP_Frost_flg : Outport  Port=382
  VOUTP_FaceM_flg : Outport  Port=383
  VOUTP_FootM_flg : Outport  Port=384
  VOUTP_CCUSyncSts_flg : Outport  Port=385
  VOUTP_ACForceOFF_flg : Outport  Port=386
  VOUTP_RecAutoFlg_flg : Outport  Port=387
  VOUTP_AirIntenZone1M_enum : Outport  Port=388
  VOUTP_fdefog_flg : Outport  Port=389
  VOUTP_sigSetTempZon2StM_C : Outport  Port=390
  VOUTP_FDCTHCMAPTCWarningSta_flg : Outport  Port=391
  VOUTP_LFBatWarn_flg : Outport  Port=392
  VOUTP_RFBatWarn_flg : Outport  Port=393
  VOUTP_LRBatWarn_flg : Outport  Port=394
  VOUTP_RRBatWarn_flg : Outport  Port=395
  VOUTP_LFWheelPress_raw8 : Outport  Port=396
  VOUTP_RFWheelPress_raw8 : Outport  Port=397
  VOUTP_LRWheelPress_raw8 : Outport  Port=398
  VOUTP_RRWheelPress_raw8 : Outport  Port=399
  VOUTP_LFWheelTemp_C : Outport  Port=400
  VOUTP_RFWheelTemp_C : Outport  Port=401
  VOUTP_LRWheelTemp_C : Outport  Port=402
  VOUTP_RRWheelTemp_C : Outport  Port=403
  VOUTP_LFSensorFail_flg : Outport  Port=404
  VOUTP_RFSensorFail_flg : Outport  Port=405
  VOUTP_LRSensorFail_flg : Outport  Port=406
  VOUTP_RRSensorFail_flg : Outport  Port=407
  VOUTP_LFWheelDebug_flg : Outport  Port=408
  VOUTP_LRWheelDebug_flg : Outport  Port=409
  VOUTP_RFWheelDebug_flg : Outport  Port=410
  VOUTP_RRWheelDebug_flg : Outport  Port=411
  VOUTP_TPMSResButtAllow_flg : Outport  Port=412
  VOUTP_TPMSCaliButtAllow_flg : Outport  Port=413
  VOUTP_LFPressIndi_enum : Outport  Port=414
  VOUTP_RFPressIndi_enum : Outport  Port=415
  VOUTP_LRPressIndi_enum : Outport  Port=416
  VOUTP_RRPressIndi_enum : Outport  Port=417
  VOUTP_TPMSWarnIndi_enum : Outport  Port=418
  VOUTP_LFWheelTmpIndi_flg : Outport  Port=419
  VOUTP_RFWheelTmpIndi_flg : Outport  Port=420
  VOUTP_LRWheelTmpIndi_flg : Outport  Port=421
  VOUTP_RRWheelTmpIndi_flg : Outport  Port=422
  VOUTP_LFWheelPSW_raw8 : Outport  Port=423
  VOUTP_LRWheelPSW_raw8 : Outport  Port=424
  VOUTP_RFWheelPSW_raw8 : Outport  Port=425
  VOUTP_RRWheelPSW_raw8 : Outport  Port=426
  VOUTP_CWheelTips_enum : Outport  Port=427
  VOUTP_AutoLTips_enum : Outport  Port=428
  VOUTP_LFSensorMode_flg : Outport  Port=429
  VOUTP_RFSensorMode_flg : Outport  Port=430
  VOUTP_LRSensorMode_flg : Outport  Port=431
  VOUTP_RRSensorMode_flg : Outport  Port=432
  VOUTP_S1ID_raw32 : Outport  Port=433
  VOUTP_S2ID_raw32 : Outport  Port=434
  VOUTP_S3ID_raw32 : Outport  Port=435
  VOUTP_S4ID_raw32 : Outport  Port=436
  VOUTP_S1L_enum : Outport  Port=437
  VOUTP_S2L_enum : Outport  Port=438
  VOUTP_S3L_enum : Outport  Port=439
  VOUTP_S4L_enum : Outport  Port=440
  VOUTP_ALFin_flg : Outport  Port=441
  VOUTP_LFP20_raw8 : Outport  Port=442
  VOUTP_RFP20_raw8 : Outport  Port=443
  VOUTP_LRP20_raw8 : Outport  Port=444
  VOUTP_RRP20_raw8 : Outport  Port=445
  VOUTP_FAT_flg : Outport  Port=446
  VOUTP_IDin_raw32 : Outport  Port=447
  VOUTP_S1WheelDebugALTU_pct : Outport  Port=448
  VOUTP_S2WheelDebugALTU_pct : Outport  Port=449
  VOUTP_S3WheelDebugALTU_pct : Outport  Port=450
  VOUTP_S4WheelDebugALTU_pct : Outport  Port=451
  VOUTP_ID1messageALTU_raw8 : Outport  Port=452
  VOUTP_ID2messageALTU_raw8 : Outport  Port=453
  VOUTP_ID3messageALTU_raw8 : Outport  Port=454
  VOUTP_ID4messageALTU_raw8 : Outport  Port=455
  VOUTP_Chkfin_flg : Outport  Port=456
  VOUTP_SetIDLoc_flg : Outport  Port=457
  VOUTP_TPMSStorge_flg : Outport  Port=458
  VOUTP_ChkStorge_flg : Outport  Port=459
  VOUTP_TPMSResButt_flg : Outport  Port=460
  VOUTP_LFPindi_enum : Outport  Port=461
  VOUTP_RFPind_enum : Outport  Port=462
  VOUTP_LRPindi_enum : Outport  Port=463
  VOUTP_RRPindi_enum : Outport  Port=464
  VOUTP_WriteChkLFID_raw : Outport  Port=465
  VOUTP_WriteChkRFID_raw : Outport  Port=466
  VOUTP_WriteChkLRID_raw : Outport  Port=467
  VOUTP_WriteChkRRID_raw : Outport  Port=468
  VOUTP_WriteChkfinLFID_raw : Outport  Port=469
  VOUTP_WriteChkfinRFID_raw : Outport  Port=470
  VOUTP_WriteChkfinLRID_raw : Outport  Port=471
  VOUTP_WriteChkfinRRID_raw : Outport  Port=472
  VOUTP_Flashchkdatavalid_enum : Outport  Port=473
  VOUTP_Flashdatavalid_enum : Outport  Port=474
  VOUTP_unlearnSfali_flg : Outport  Port=475
  VOUTP_unlearnSfailvalid_enum : Outport  Port=476
  VOUTP_Prepresstempvalid_enum : Outport  Port=477
  VOUTP_FlashS1ID_raw : Outport  Port=478
  VOUTP_FlashS2ID_raw : Outport  Port=479
  VOUTP_FlashS3ID_raw : Outport  Port=480
  VOUTP_FlashS4ID_raw : Outport  Port=481
  VOUTP_FlashIDvalid_enum : Outport  Port=482
  VOUTP_ParkRequest_flg : Outport  Port=483
  VOUTP_TqSourceFr_enum : Outport  Port=484
  VOUTP_TqSourceRr_enum : Outport  Port=485
  VOUTP_FrEDUAvailBrkRgnTq_Nm : Outport  Port=486
  VOUTP_RrEDUAvailBrkRgnTq_Nm : Outport  Port=487
  VOUTP_EVDriveMode_enum : Outport  Port=488
  VOUTP_ShiftGearPosn_enum : Outport  Port=489
  VOUTP_PButtonSta_enum : Outport  Port=490
  VOUTP_FrActvDmpDisabReq_flg : Outport  Port=491
  VOUTP_RrActvDmpDisabReq_flg : Outport  Port=492
  VOUTP_FrRgnDecrSta_flg : Outport  Port=493
  VOUTP_RrRgnDecrSta_flg : Outport  Port=494
  VOUTP_DriverWhlTqDemFr_Nm : Outport  Port=495
  VOUTP_DriverWhlTqDemRr_Nm : Outport  Port=496
  VOUTP_FrEDUActTq_Nm : Outport  Port=497
  VOUTP_RrEDUActTq_Nm : Outport  Port=498
  VOUTP_FrEDURolRgnTq_Nm : Outport  Port=499
  VOUTP_RrEDURolRgnTq_Nm : Outport  Port=500
  VOUTP_FrEDUSpd_rpm : Outport  Port=501
  VOUTP_RrEDUSpd_rpm : Outport  Port=502
  VOUTP_FrEDUSpdValid_flg : Outport  Port=503
  VOUTP_FrEDUAvailBrkRgnTqV_flg : Outport  Port=504
  VOUTP_RrEDUSpdValid_flg : Outport  Port=505
  VOUTP_RrEDUAvailBrkRgnTqV_flg : Outport  Port=506
  VOUTP_RgnAbnorSta_flg : Outport  Port=507
  VOUTP_PTCSPermSta_flg : Outport  Port=508
  VOUTP_FrRgnPermSta_flg : Outport  Port=509
  VOUTP_RrRgnPermSta_flg : Outport  Port=510
  VOUTP_FrIdcMin_A : Outport  Port=511
  VOUTP_FrIdcMax_A : Outport  Port=512
  VOUTP_FrUdcMin_V : Outport  Port=513
  VOUTP_FrUdcMax_V : Outport  Port=514
  VOUTP_RrIdcMin_A : Outport  Port=515
  VOUTP_RrIdcMax_A : Outport  Port=516
  VOUTP_RrUdcMin_V : Outport  Port=517
  VOUTP_RrUdcMax_V : Outport  Port=518
  VOUTP_ReBrakeLPReq_flg : Outport  Port=519
  VOUTP_CreepON_flg : Outport  Port=520
  VOUTP_ActEMpTrq_pct : Outport  Port=521
  VOUTP_ActMaxAvaEMRecpTrq_pct : Outport  Port=522
  VOUTP_ActDriveDirect_enum : Outport  Port=523
  VOUTP_DLEngaged_enum : Outport  Port=524
  VOUTP_EMTrqModeDrvBrk_enum : Outport  Port=525
  VOUTP_ActEMpTrqHrls_pct : Outport  Port=526
  VOUTP_ActEMOutSftSpd_rpm : Outport  Port=527
  VOUTP_DrvDemEMRtapTrq_pct : Outport  Port=528
  VOUTP_SACtrlDev_enum : Outport  Port=529
  VOUTP_RetSelNonEng_pct : Outport  Port=530
  VOUTP_ShiftPgs_enum : Outport  Port=531
  VOUTP_AccPedal1LowSW_enum : Outport  Port=532
  VOUTP_AccPedalPos1_pct : Outport  Port=533
  VOUTP_ParkBrakeSW_enum : Outport  Port=534
  VOUTP_VCUVehSpd_kph : Outport  Port=535
  VOUTP_BrakeSW_enum : Outport  Port=536
  VOUTP_NFricPercTorq_pct : Outport  Port=537
  VOUTP_EMParasLoss_pct : Outport  Port=538
  VOUTP_EEC2MSGCnt_raw : Outport  Port=539
  VOUTP_EEC2MSGCS_raw : Outport  Port=540
  VOUTP_FDCCHAEBSRd4BRSta_enum : Outport  Port=541
  VOUTP_FDCCHAEBSHBSwSta_enum : Outport  Port=542
  VOUTP_FDCCHAEBSHHSwSta_enum : Outport  Port=543
  VOUTP_FDCVCUTUpAStaSta_enum : Outport  Port=544
  VOUTP_FDCVCUDACStatusSta_enum : Outport  Port=545
  VOUTP_FrTMTqReq_Nm : Outport  Port=546
  VOUTP_RrTMTqReq_Nm : Outport  Port=547
  VOUTP_ReqOBCV2LEna_enum : Outport  Port=548
  VOUTP_ReqV2LIVIPopup_enum : Outport  Port=549
  VOUTP_FeatSetSpdFinal_raw32 : Outport  Port=550
  VOUTP_VehicleSpeed_mph : Outport  Port=551
  VOUTP_VehicleSpeed_kph : Outport  Port=552
  VOUTP_MeterIndSpeed_raw32 : Outport  Port=553
  VOUTP_VMCAEBCtrlAvail_flg : Outport  Port=554
  VOUTP_VMCACCCtrlAvail_flg : Outport  Port=555
  VOUTP_VMCCCCtrlAvail_flg : Outport  Port=556
  VOUTP_VMCMSACtrlAvail_flg : Outport  Port=557
  VOUTP_FeatArbitrSta_enum : Outport  Port=558
  VOUTP_FeatReqSpd_kph : Outport  Port=559
  VOUTP_JerkPCT_pct : Outport  Port=560
  VOUTP_LimitPCT_pct : Outport  Port=561
  VOUTP_FrontRearSlipRatioCtrl_flg : Outport  Port=562
  VOUTP_RearWhlSlipRatioCtrl_flg : Outport  Port=563
  VOUTP_SingleWhlSlipRatioCtrl_flg : Outport  Port=564
  VOUTP_LatAccCtrl_flg : Outport  Port=565
  VOUTP_SafetyCtrl_flg : Outport  Port=566
  VOUTP_SPD2ACCAct_flg : Outport  Port=567
  VOUTP_AccCalcuPID_mps2 : Outport  Port=568
  VOUTP_ISOAccLimit_mps2 : Outport  Port=569
  VOUTP_ISODecLimit_mps2 : Outport  Port=570
  VOUTP_ISOJerkLimit_mps3 : Outport  Port=571
  VOUTP_ACCRequiredAccel_mps2 : Outport  Port=572
  VOUTP_DISCReqAcc_mps2 : Outport  Port=573
  VOUTP_FeatArbitrFinal_enum : Outport  Port=574
  VOUTP_LateralCtrl_flg : Outport  Port=575
  VOUTP_ADASLKASta_enum : Outport  Port=576
  VOUTP_LKAStrToqReq_Nm : Outport  Port=577
  VOUTP_LKATOIFault_flg : Outport  Port=578
  VOUTP_LKATOIAct_enum : Outport  Port=579
  VOUTP_ADASAEBReq_enum : Outport  Port=580
  VOUTP_ADASFaultSta_flg : Outport  Port=581
  VOUTP_AEBVehHoldReq_flg : Outport  Port=582
  VOUTP_ACCVehHoldReq_flg : Outport  Port=583
  VOUTP_ADASDBSReq_enum : Outport  Port=584
  VOUTP_ADASACCSta_enum : Outport  Port=585
  VOUTP_ACCObjDist_m : Outport  Port=586
  VOUTP_ACCObjRelSpd_mps : Outport  Port=587
  VOUTP_TimeGapLevel_enum : Outport  Port=588
  VOUTP_ACCJerkUpperLimit_mps3 : Outport  Port=589
  VOUTP_ACCComfortBandUpper_mps2 : Outport  Port=590
  VOUTP_ACCJerkLowerLimit_mps3 : Outport  Port=591
  VOUTP_ACCComfortBandLower_mps2 : Outport  Port=592
  VOUTP_ADASVehSpdLim_raw32 : Outport  Port=593
  VOUTP_ADASShftPosnReqA_flg : Outport  Port=594
  VOUTP_ADASShftPosnReq_enum : Outport  Port=595
  VOUTP_ADASForceIdle_flg : Outport  Port=596
  VOUTP_HazardWarningReq_flg : Outport  Port=597
  VOUTP_RightTurnLightReq_flg : Outport  Port=598
  VOUTP_LeftTurnLightReq_flg : Outport  Port=599
  VOUTP_ADASFCWSta_enum : Outport  Port=600
  VOUTP_ADASLDWSta_enum : Outport  Port=601
  VOUTP_ADASFltWrnReq_flg : Outport  Port=602
  VOUTP_ACCObjDstLvl_enum : Outport  Port=603
  VOUTP_ForceLowBeam_enum : Outport  Port=604
  VOUTP_ACCTakeoverReq_flg : Outport  Port=605
  VOUTP_ADASWarningMsg_enum : Outport  Port=606
  VOUTP_ADASCAMSpdLim_enum : Outport  Port=607
  VOUTP_TargetType_enum : Outport  Port=608
  VOUTP_ADASSLIFSpdLim_enum : Outport  Port=609
  VOUTP_LKAHODDisplayWarning_flg : Outport  Port=610
  VOUTP_LKAHODSoundWarning_flg : Outport  Port=611
  VOUTP_ADASLFCSta_enum : Outport  Port=612
  VOUTP_ADASLaneModeL_enum : Outport  Port=613
  VOUTP_ADASLaneModeR_enum : Outport  Port=614
  VOUTP_ADASSLIFSta_enum : Outport  Port=615
  VOUTP_ADASISASta_enum : Outport  Port=616
  VOUTP_ADASLDWMute_flg : Outport  Port=617
  VOUTP_ADASFCWMute_flg : Outport  Port=618
  VOUTP_ADASLFCHandsOffWarning_enum : Outport  Port=619
  VOUTP_LVDADisabled_flg : Outport  Port=620
  VOUTP_LVDAMuteSta_enum : Outport  Port=621
  VOUTP_LVDAFailinfo_flg : Outport  Port=622
  VOUTP_LVDAWarning_flg : Outport  Port=623
  VOUTP_LVDAACCStatusInformation_flg : Outport  Port=624
  VOUTP_ADASLFCWarnSound_enum : Outport  Port=625
  VOUTP_FCMACCmode_enum : Outport  Port=626
  VOUTP_ADASLanetypeR_enum : Outport  Port=627
  VOUTP_ADASLanetypeL_enum : Outport  Port=628
  VOUTP_ADASLanecurveL_raw32 : Outport  Port=629
  VOUTP_ADASLanecurveR_raw32 : Outport  Port=630
  VOUTP_ADASAEBSta_enum : Outport  Port=631
  VOUTP_FCMLDWRequest_enum : Outport  Port=632
  VOUTP_FCMLDWFault_flg : Outport  Port=633
  VOUTP_ACCCtrlAvail_flg : Outport  Port=634
  VOUTP_ACCPedalOvrd_flg : Outport  Port=635
  VOUTP_TimeGapCalcu_s : Outport  Port=636
  VOUTP_CCCtrlSta_enum : Outport  Port=637
  VOUTP_MSACtrlSta_enum : Outport  Port=638
  VOUTP_APSCtrlAvail_flg : Outport  Port=639
  VOUTP_APSStaSys_enum : Outport  Port=640
  VOUTP_APSDecReqA_flg : Outport  Port=641
  VOUTP_APSDecReq_mps2 : Outport  Port=642
  VOUTP_APSReq_enum : Outport  Port=643
  VOUTP_CCMSASpdWar_flg : Outport  Port=644
  VOUTP_IMUEnaCmd_flg : Outport  Port=645
  wires:
  VACC_HVTHCMSysAvail_enum/1 -> VACC_HVTHCMSysAvail_enum_Inproc/1  "VACC_HVTHCMSysAvail_enum"
  VACC_HVTHCMSysAvail_enum_Inproc/1 -> UnitConverter1/1
  UnitConverter1/1 -> VOUTP_HVTHCMSysAvail_enum/1  "VOUTP_HVTHCMSysAvail_enum"
  VACC_LVBattVoltSta_enum/1 -> VACC_LVBattVoltSta_enum_Inproc/1  "VACC_LVBattVoltSta_enum"
  VACC_LVBattVoltSta_enum_Inproc/1 -> UnitConverter2/1
  UnitConverter2/1 -> VOUTP_LVBattVoltSta_enum/1  "VOUTP_LVBattVoltSta_enum"
  VACC_VehHVPwrAvail4THCM_W/1 -> VACC_VehHVPwrAvail4THCM_W_Inproc/1  "VACC_VehHVPwrAvail4THCM_W"
  VACC_VehHVPwrAvail4THCM_W_Inproc/1 -> UnitConverter3/1
  UnitConverter3/1 -> VOUTP_VehHVPwrAvail4THCM_W/1  "VOUTP_VehHVPwrAvail4THCM_W"
  VACC_EHPSEnDem_enum/1 -> VACC_EHPSEnDem_enum_Inproc/1  "VACC_EHPSEnDem_enum"
  VACC_EHPSEnDem_enum_Inproc/1 -> UnitConverter4/1
  UnitConverter4/1 -> VOUTP_EHPSEnDem_enum/1  "VOUTP_EHPSEnDem_enum"
  VACC_CACPresWarnSta_flg/1 -> VACC_CACPresWarnSta_flg_Inproc/1  "VACC_CACPresWarnSta_flg"
  VACC_CACPresWarnSta_flg_Inproc/1 -> UnitConverter5/1
  UnitConverter5/1 -> VOUTP_CACPresWarnSta_flg/1  "VOUTP_CACPresWarnSta_flg"
  VACC_CACTempWarnSta_flg/1 -> VACC_CACTempWarnSta_flg_Inproc/1  "VACC_CACTempWarnSta_flg"
  VACC_CACTempWarnSta_flg_Inproc/1 -> UnitConverter6/1
  UnitConverter6/1 -> VOUTP_CACTempWarnSta_flg/1  "VOUTP_CACTempWarnSta_flg"
  VACC_EACEnDem_enum/1 -> VACC_EACEnDem_enum_Inproc/1  "VACC_EACEnDem_enum"
  VACC_EACEnDem_enum_Inproc/1 -> UnitConverter7/1
  UnitConverter7/1 -> VOUTP_EACEnDem_enum/1  "VOUTP_EACEnDem_enum"
  VAPM_VehSpeedToAPM_kph/1 -> VAPM_VehSpeedToAPM_kph_Inproc/1  "VAPM_VehSpeedToAPM_kph"
  VAPM_VehSpeedToAPM_kph_Inproc/1 -> UnitConverter8/1
  UnitConverter8/1 -> VOUTP_VehSpeedToAPM_kph/1  "VOUTP_VehSpeedToAPM_kph"
  VAPM_VehSpeedTimeOut_flg/1 -> VAPM_VehSpeedTimeOut_flg_Inproc/1  "VAPM_VehSpeedTimeOut_flg"
  VAPM_VehSpeedTimeOut_flg_Inproc/1 -> UnitConverter9/1
  UnitConverter9/1 -> VOUTP_VehSpeedTimeOut_flg/1  "VOUTP_VehSpeedTimeOut_flg"
  VAPM_FSOffSw_enum/1 -> VAPM_FSOffSw_enum_Inproc/1  "VAPM_FSOffSw_enum"
  VAPM_FSOffSw_enum_Inproc/1 -> UnitConverter10/1
  UnitConverter10/1 -> VOUTP_FSOffSw_enum/1  "VOUTP_FSOffSw_enum"
  VAPM_FSOffSwTimeOut_flg/1 -> VAPM_FSOffSwTimeOut_flg_Inproc/1  "VAPM_FSOffSwTimeOut_flg"
  VAPM_FSOffSwTimeOut_flg_Inproc/1 -> UnitConverter11/1
  UnitConverter11/1 -> VOUTP_FSOffSwTimeOut_flg/1  "VOUTP_FSOffSwTimeOut_flg"
  VAPM_ChrgPlugSta_enum/1 -> VAPM_ChrgPlugSta_enum_Inproc/1  "VAPM_ChrgPlugSta_enum"
  VAPM_ChrgPlugSta_enum_Inproc/1 -> UnitConverter12/1
  UnitConverter12/1 -> VOUTP_ChrgPlugSta_enum/1  "VOUTP_ChrgPlugSta_enum"
  VAPM_PASDRMR_cm/1 -> VAPM_PASDRMR_cm_Inproc/1  "VAPM_PASDRMR_cm"
  VAPM_PASDRMR_cm_Inproc/1 -> UnitConverter13/1
  UnitConverter13/1 -> VOUTP_PASDRMR_cm/1  "VOUTP_PASDRMR_cm"
  VAPM_PASDRML_cm/1 -> VAPM_PASDRML_cm_Inproc/1  "VAPM_PASDRML_cm"
  VAPM_PASDRML_cm_Inproc/1 -> UnitConverter14/1
  UnitConverter14/1 -> VOUTP_PASDRML_cm/1  "VOUTP_PASDRML_cm"
  VAPM_PASDRCR_cm/1 -> VAPM_PASDRCR_cm_Inproc/1  "VAPM_PASDRCR_cm"
  VAPM_PASDRCR_cm_Inproc/1 -> UnitConverter15/1
  UnitConverter15/1 -> VOUTP_PASDRCR_cm/1  "VOUTP_PASDRCR_cm"
  VAPM_PASDRCL_cm/1 -> VAPM_PASDRCL_cm_Inproc/1  "VAPM_PASDRCL_cm"
  VAPM_PASDRCL_cm_Inproc/1 -> UnitConverter16/1
  UnitConverter16/1 -> VOUTP_PASDRCL_cm/1  "VOUTP_PASDRCL_cm"
  VAPM_PASDFMR_cm/1 -> VAPM_PASDFMR_cm_Inproc/1  "VAPM_PASDFMR_cm"
  VAPM_PASDFMR_cm_Inproc/1 -> UnitConverter17/1
  UnitConverter17/1 -> VOUTP_PASDFMR_cm/1  "VOUTP_PASDFMR_cm"
  VAPM_PASDFML_cm/1 -> VAPM_PASDFML_cm_Inproc/1  "VAPM_PASDFML_cm"
  VAPM_PASDFML_cm_Inproc/1 -> UnitConverter18/1
  UnitConverter18/1 -> VOUTP_PASDFML_cm/1  "VOUTP_PASDFML_cm"
  VAPM_PASDFCR_cm/1 -> VAPM_PASDFCR_cm_Inproc/1  "VAPM_PASDFCR_cm"
  VAPM_PASDFCR_cm_Inproc/1 -> UnitConverter19/1
  UnitConverter19/1 -> VOUTP_PASDFCR_cm/1  "VOUTP_PASDFCR_cm"
  VAPM_PASDFCL_cm/1 -> VAPM_PASDFCL_cm_Inproc/1  "VAPM_PASDFCL_cm"
  VAPM_PASDFCL_cm_Inproc/1 -> UnitConverter20/1
  UnitConverter20/1 -> VOUTP_PASDFCL_cm/1  "VOUTP_PASDFCL_cm"
  VAPM_APSDRLR_cm/1 -> VAPM_APSDRLR_cm_Inproc/1  "VAPM_APSDRLR_cm"
  VAPM_APSDRLR_cm_Inproc/1 -> UnitConverter21/1
  UnitConverter21/1 -> VOUTP_APSDRLR_cm/1  "VOUTP_APSDRLR_cm"
  VAPM_APSDRLL_cm/1 -> VAPM_APSDRLL_cm_Inproc/1  "VAPM_APSDRLL_cm"
  VAPM_APSDRLL_cm_Inproc/1 -> UnitConverter22/1
  UnitConverter22/1 -> VOUTP_APSDRLL_cm/1  "VOUTP_APSDRLL_cm"
  VAPM_APSDFLR_cm/1 -> VAPM_APSDFLR_cm_Inproc/1  "VAPM_APSDFLR_cm"
  VAPM_APSDFLR_cm_Inproc/1 -> UnitConverter23/1
  UnitConverter23/1 -> VOUTP_APSDFLR_cm/1  "VOUTP_APSDFLR_cm"
  VAPM_APSDFLL_cm/1 -> VAPM_APSDFLL_cm_Inproc/1  "VAPM_APSDFLL_cm"
  VAPM_APSDFLL_cm_Inproc/1 -> UnitConverter24/1
  UnitConverter24/1 -> VOUTP_APSDFLL_cm/1  "VOUTP_APSDFLL_cm"
  VAPM_PASAFCL_enum/1 -> VAPM_PASAFCL_enum_Inproc/1  "VAPM_PASAFCL_enum"
  VAPM_PASAFCL_enum_Inproc/1 -> UnitConverter25/1
  UnitConverter25/1 -> VOUTP_PASAFCL_enum/1  "VOUTP_PASAFCL_enum"
  VAPM_PASARMR_enum/1 -> VAPM_PASARMR_enum_Inproc/1  "VAPM_PASARMR_enum"
  VAPM_PASARMR_enum_Inproc/1 -> UnitConverter26/1
  UnitConverter26/1 -> VOUTP_PASARMR_enum/1  "VOUTP_PASARMR_enum"
  VAPM_PASARML_enum/1 -> VAPM_PASARML_enum_Inproc/1  "VAPM_PASARML_enum"
  VAPM_PASARML_enum_Inproc/1 -> UnitConverter27/1
  UnitConverter27/1 -> VOUTP_PASARML_enum/1  "VOUTP_PASARML_enum"
  VAPM_PASARCR_enum/1 -> VAPM_PASARCR_enum_Inproc/1  "VAPM_PASARCR_enum"
  VAPM_PASARCR_enum_Inproc/1 -> UnitConverter28/1
  UnitConverter28/1 -> VOUTP_PASARCR_enum/1  "VOUTP_PASARCR_enum"
  VAPM_PASARCL_enum/1 -> VAPM_PASARCL_enum_Inproc/1  "VAPM_PASARCL_enum"
  VAPM_PASARCL_enum_Inproc/1 -> UnitConverter29/1
  UnitConverter29/1 -> VOUTP_PASARCL_enum/1  "VOUTP_PASARCL_enum"
  VAPM_PASAFMR_enum/1 -> VAPM_PASAFMR_enum_Inproc/1  "VAPM_PASAFMR_enum"
  VAPM_PASAFMR_enum_Inproc/1 -> UnitConverter30/1
  UnitConverter30/1 -> VOUTP_PASAFMR_enum/1  "VOUTP_PASAFMR_enum"
  VAPM_PASAFML_enum/1 -> VAPM_PASAFML_enum_Inproc/1  "VAPM_PASAFML_enum"
  VAPM_PASAFML_enum_Inproc/1 -> UnitConverter31/1
  UnitConverter31/1 -> VOUTP_PASAFML_enum/1  "VOUTP_PASAFML_enum"
  VAPM_PASAFCR_enum/1 -> VAPM_PASAFCR_enum_Inproc/1  "VAPM_PASAFCR_enum"
  VAPM_PASAFCR_enum_Inproc/1 -> UnitConverter32/1
  UnitConverter32/1 -> VOUTP_PASAFCR_enum/1  "VOUTP_PASAFCR_enum"
  VAPM_USSStaRMR_flg/1 -> VAPM_USSStaRMR_flg_Inproc/1  "VAPM_USSStaRMR_flg"
  VAPM_USSStaRMR_flg_Inproc/1 -> UnitConverter33/1
  UnitConverter33/1 -> VOUTP_USSStaRMR_flg/1  "VOUTP_USSStaRMR_flg"
  VAPM_USSStaRML_flg/1 -> VAPM_USSStaRML_flg_Inproc/1  "VAPM_USSStaRML_flg"
  VAPM_USSStaRML_flg_Inproc/1 -> UnitConverter34/1
  UnitConverter34/1 -> VOUTP_USSStaRML_flg/1  "VOUTP_USSStaRML_flg"
  VAPM_USSStaRLR_flg/1 -> VAPM_USSStaRLR_flg_Inproc/1  "VAPM_USSStaRLR_flg"
  VAPM_USSStaRLR_flg_Inproc/1 -> UnitConverter35/1
  UnitConverter35/1 -> VOUTP_USSStaRLR_flg/1  "VOUTP_USSStaRLR_flg"
  VAPM_USSStaRLL_flg/1 -> VAPM_USSStaRLL_flg_Inproc/1  "VAPM_USSStaRLL_flg"
  VAPM_USSStaRLL_flg_Inproc/1 -> UnitConverter36/1
  UnitConverter36/1 -> VOUTP_USSStaRLL_flg/1  "VOUTP_USSStaRLL_flg"
  VAPM_USSStaRCR_flg/1 -> VAPM_USSStaRCR_flg_Inproc/1  "VAPM_USSStaRCR_flg"
  VAPM_USSStaRCR_flg_Inproc/1 -> UnitConverter37/1
  UnitConverter37/1 -> VOUTP_USSStaRCR_flg/1  "VOUTP_USSStaRCR_flg"
  VAPM_USSStaRCL_flg/1 -> VAPM_USSStaRCL_flg_Inproc/1  "VAPM_USSStaRCL_flg"
  VAPM_USSStaRCL_flg_Inproc/1 -> UnitConverter38/1
  UnitConverter38/1 -> VOUTP_USSStaRCL_flg/1  "VOUTP_USSStaRCL_flg"
  VAPM_USSStaFMR_flg/1 -> VAPM_USSStaFMR_flg_Inproc/1  "VAPM_USSStaFMR_flg"
  VAPM_USSStaFMR_flg_Inproc/1 -> UnitConverter39/1
  UnitConverter39/1 -> VOUTP_USSStaFMR_flg/1  "VOUTP_USSStaFMR_flg"
  VAPM_USSStaFML_flg/1 -> VAPM_USSStaFML_flg_Inproc/1  "VAPM_USSStaFML_flg"
  VAPM_USSStaFML_flg_Inproc/1 -> UnitConverter40/1
  UnitConverter40/1 -> VOUTP_USSStaFML_flg/1  "VOUTP_USSStaFML_flg"
  VAPM_USSStaFLR_flg/1 -> VAPM_USSStaFLR_flg_Inproc/1  "VAPM_USSStaFLR_flg"
  VAPM_USSStaFLR_flg_Inproc/1 -> UnitConverter41/1
  UnitConverter41/1 -> VOUTP_USSStaFLR_flg/1  "VOUTP_USSStaFLR_flg"
  VAPM_USSStaFLL_flg/1 -> VAPM_USSStaFLL_flg_Inproc/1  "VAPM_USSStaFLL_flg"
  VAPM_USSStaFLL_flg_Inproc/1 -> UnitConverter42/1
  UnitConverter42/1 -> VOUTP_USSStaFLL_flg/1  "VOUTP_USSStaFLL_flg"
  VAPM_USSStaFCR_flg/1 -> VAPM_USSStaFCR_flg_Inproc/1  "VAPM_USSStaFCR_flg"
  VAPM_USSStaFCR_flg_Inproc/1 -> UnitConverter43/1
  UnitConverter43/1 -> VOUTP_USSStaFCR_flg/1  "VOUTP_USSStaFCR_flg"
  VAPM_USSStaFCL_flg/1 -> VAPM_USSStaFCL_flg_Inproc/1  "VAPM_USSStaFCL_flg"
  VAPM_USSStaFCL_flg_Inproc/1 -> UnitConverter44/1
  UnitConverter44/1 -> VOUTP_USSStaFCL_flg/1  "VOUTP_USSStaFCL_flg"
  VAPM_Chime_enum/1 -> VAPM_Chime_enum_Inproc/1  "VAPM_Chime_enum"
  VAPM_Chime_enum_Inproc/1 -> UnitConverter45/1
  UnitConverter45/1 -> VOUTP_Chime_enum/1  "VOUTP_Chime_enum"
  VAPM_SNSRLayout_enum/1 -> VAPM_SNSRLayout_enum_Inproc/1  "VAPM_SNSRLayout_enum"
  VAPM_SNSRLayout_enum_Inproc/1 -> UnitConverter46/1
  UnitConverter46/1 -> VOUTP_SNSRLayout_enum/1  "VOUTP_SNSRLayout_enum"
  VAPM_StaFSya_flg/1 -> VAPM_StaFSya_flg_Inproc/1  "VAPM_StaFSya_flg"
  VAPM_StaFSya_flg_Inproc/1 -> UnitConverter47/1
  UnitConverter47/1 -> VOUTP_StaFSya_flg/1  "VOUTP_StaFSya_flg"
  VAPM_ModOperation_enum/1 -> VAPM_ModOperation_enum_Inproc/1  "VAPM_ModOperation_enum"
  VAPM_ModOperation_enum_Inproc/1 -> UnitConverter48/1
  UnitConverter48/1 -> VOUTP_ModOperation_enum/1  "VOUTP_ModOperation_enum"
  VAPM_BrkPedalPosToAPM_pct/1 -> VAPM_BrkPedalPosToAPM_pct_Inproc/1  "VAPM_BrkPedalPosToAPM_pct"
  VAPM_BrkPedalPosToAPM_pct_Inproc/1 -> UnitConverter49/1
  UnitConverter49/1 -> VOUTP_BrkPedalPosToAPM_pct/1  "VOUTP_BrkPedalPosToAPM_pct"
  VAPM_BrkPedalPosTimeOut_flg/1 -> VAPM_BrkPedalPosTimeOut_flg_Inproc/1  "VAPM_BrkPedalPosTimeOut_flg"
  VAPM_BrkPedalPosTimeOut_flg_Inproc/1 -> UnitConverter50/1
  UnitConverter50/1 -> VOUTP_BrkPedalPosTimeOut_flg/1  "VOUTP_BrkPedalPosTimeOut_flg"
  VAPM_LFRawWhlSpeed_kph/1 -> VAPM_LFRawWhlSpeed_kph_Inproc/1  "VAPM_LFRawWhlSpeed_kph"
  VAPM_LFRawWhlSpeed_kph_Inproc/1 -> UnitConverter51/1
  UnitConverter51/1 -> VOUTP_LFRawWhlSpeed_kph/1  "VOUTP_LFRawWhlSpeed_kph"
  VAPM_LFRawWhlSpeedTimeOut_flg/1 -> VAPM_LFRawWhlSpeedTimeOut_flg_Inproc/1  "VAPM_LFRawWhlSpeedTimeOut_flg"
  VAPM_LFRawWhlSpeedTimeOut_flg_Inproc/1 -> UnitConverter52/1
  UnitConverter52/1 -> VOUTP_LFRawWhlSpeedTimeOut_flg/1  "VOUTP_LFRawWhlSpeedTimeOut_flg"
  VAPM_RFRawWhlSpeed_kph/1 -> VAPM_RFRawWhlSpeed_kph_Inproc/1  "VAPM_RFRawWhlSpeed_kph"
  VAPM_RFRawWhlSpeed_kph_Inproc/1 -> UnitConverter53/1
  UnitConverter53/1 -> VOUTP_RFRawWhlSpeed_kph/1  "VOUTP_RFRawWhlSpeed_kph"
  VAPM_RFRawWhlSpeedTimeOut_flg/1 -> VAPM_RFRawWhlSpeedTimeOut_flg_Inproc/1  "VAPM_RFRawWhlSpeedTimeOut_flg"
  VAPM_RFRawWhlSpeedTimeOut_flg_Inproc/1 -> UnitConverter54/1
  UnitConverter54/1 -> VOUTP_RFRawWhlSpeedTimeOut_flg/1  "VOUTP_RFRawWhlSpeedTimeOut_flg"
  VAPM_LRRawWhlSpeed_kph/1 -> VAPM_LRRawWhlSpeed_kph_Inproc/1  "VAPM_LRRawWhlSpeed_kph"
  VAPM_LRRawWhlSpeed_kph_Inproc/1 -> UnitConverter55/1
  UnitConverter55/1 -> VOUTP_LRRawWhlSpeed_kph/1  "VOUTP_LRRawWhlSpeed_kph"
  VAPM_LRRawWhlSpeedTimeOut_flg/1 -> VAPM_LRRawWhlSpeedTimeOut_flg_Inproc/1  "VAPM_LRRawWhlSpeedTimeOut_flg"
  VAPM_LRRawWhlSpeedTimeOut_flg_Inproc/1 -> UnitConverter56/1
  UnitConverter56/1 -> VOUTP_LRRawWhlSpeedTimeOut_flg/1  "VOUTP_LRRawWhlSpeedTimeOut_flg"
  VAPM_RRRawWhlSpeed_kph/1 -> VAPM_RRRawWhlSpeed_kph_Inproc/1  "VAPM_RRRawWhlSpeed_kph"
  VAPM_RRRawWhlSpeed_kph_Inproc/1 -> UnitConverter57/1
  UnitConverter57/1 -> VOUTP_RRRawWhlSpeed_kph/1  "VOUTP_RRRawWhlSpeed_kph"
  VAPM_RRRawWhlSpeedTimeOut_flg/1 -> VAPM_RRRawWhlSpeedTimeOut_flg_Inproc/1  "VAPM_RRRawWhlSpeedTimeOut_flg"
  VAPM_RRRawWhlSpeedTimeOut_flg_Inproc/1 -> UnitConverter58/1
  UnitConverter58/1 -> VOUTP_RRRawWhlSpeedTimeOut_flg/1  "VOUTP_RRRawWhlSpeedTimeOut_flg"
  VAPM_LFRawWhlSpeedV_flg/1 -> VAPM_LFRawWhlSpeedV_flg_Inproc/1  "VAPM_LFRawWhlSpeedV_flg"
  VAPM_LFRawWhlSpeedV_flg_Inproc/1 -> UnitConverter59/1
  UnitConverter59/1 -> VOUTP_LFRawWhlSpeedV_flg/1  "VOUTP_LFRawWhlSpeedV_flg"
  VAPM_LFRawWhlSpeedVTimeOut_flg/1 -> VAPM_LFRawWhlSpeedVTimeOut_flg_Inproc/1  "VAPM_LFRawWhlSpeedVTimeOut_flg"
  VAPM_LFRawWhlSpeedVTimeOut_flg_Inproc/1 -> UnitConverter60/1
  UnitConverter60/1 -> VOUTP_LFRawWhlSpeedVTimeOut_flg/1  "VOUTP_LFRawWhlSpeedVTimeOut_flg"
  VAPM_RFRawWhlSpeedV_flg/1 -> VAPM_RFRawWhlSpeedV_flg_Inproc/1  "VAPM_RFRawWhlSpeedV_flg"
  VAPM_RFRawWhlSpeedV_flg_Inproc/1 -> UnitConverter61/1
  UnitConverter61/1 -> VOUTP_RFRawWhlSpeedV_flg/1  "VOUTP_RFRawWhlSpeedV_flg"
  VAPM_RFRawWhlSpeedVTimeOut_flg/1 -> VAPM_RFRawWhlSpeedVTimeOut_flg_Inproc/1  "VAPM_RFRawWhlSpeedVTimeOut_flg"
  VAPM_RFRawWhlSpeedVTimeOut_flg_Inproc/1 -> UnitConverter62/1
  UnitConverter62/1 -> VOUTP_RFRawWhlSpeedVTimeOut_flg/1  "VOUTP_RFRawWhlSpeedVTimeOut_flg"
  VAPM_LRRawWhlSpeedV_flg/1 -> VAPM_LRRawWhlSpeedV_flg_Inproc/1  "VAPM_LRRawWhlSpeedV_flg"
  VAPM_LRRawWhlSpeedV_flg_Inproc/1 -> UnitConverter63/1
  UnitConverter63/1 -> VOUTP_LRRawWhlSpeedV_flg/1  "VOUTP_LRRawWhlSpeedV_flg"
  VAPM_LRRawWhlSpeedVTimeOut_flg/1 -> VAPM_LRRawWhlSpeedVTimeOut_flg_Inproc/1  "VAPM_LRRawWhlSpeedVTimeOut_flg"
  VAPM_LRRawWhlSpeedVTimeOut_flg_Inproc/1 -> UnitConverter64/1
  UnitConverter64/1 -> VOUTP_LRRawWhlSpeedVTimeOut_flg/1  "VOUTP_LRRawWhlSpeedVTimeOut_flg"
  VAPM_RRRawWhlSpeedV_flg/1 -> VAPM_RRRawWhlSpeedV_flg_Inproc/1  "VAPM_RRRawWhlSpeedV_flg"
  VAPM_RRRawWhlSpeedV_flg_Inproc/1 -> UnitConverter65/1
  UnitConverter65/1 -> VOUTP_RRRawWhlSpeedV_flg/1  "VOUTP_RRRawWhlSpeedV_flg"
  VAPM_RRRawWhlSpeedVTimeOut_flg/1 -> VAPM_RRRawWhlSpeedVTimeOut_flg_Inproc/1  "VAPM_RRRawWhlSpeedVTimeOut_flg"
  VAPM_RRRawWhlSpeedVTimeOut_flg_Inproc/1 -> UnitConverter66/1
  UnitConverter66/1 -> VOUTP_RRRawWhlSpeedVTimeOut_flg/1  "VOUTP_RRRawWhlSpeedVTimeOut_flg"
  VAPM_LFWhlRotDir_enum/1 -> VAPM_LFWhlRotDir_enum_Inproc/1  "VAPM_LFWhlRotDir_enum"
  VAPM_LFWhlRotDir_enum_Inproc/1 -> UnitConverter67/1
  UnitConverter67/1 -> VOUTP_LFWhlRotDir_enum/1  "VOUTP_LFWhlRotDir_enum"
  VAPM_LFWhlRotDirTimeOut_flg/1 -> VAPM_LFWhlRotDirTimeOut_flg_Inproc/1  "VAPM_LFWhlRotDirTimeOut_flg"
  VAPM_LFWhlRotDirTimeOut_flg_Inproc/1 -> UnitConverter68/1
  UnitConverter68/1 -> VOUTP_LFWhlRotDirTimeOut_flg/1  "VOUTP_LFWhlRotDirTimeOut_flg"
  VAPM_RFWhlRotDir_enum/1 -> VAPM_RFWhlRotDir_enum_Inproc/1  "VAPM_RFWhlRotDir_enum"
  VAPM_RFWhlRotDir_enum_Inproc/1 -> UnitConverter69/1
  UnitConverter69/1 -> VOUTP_RFWhlRotDir_enum/1  "VOUTP_RFWhlRotDir_enum"
  VAPM_RFWhlRotDirTimeOut_flg/1 -> VAPM_RFWhlRotDirTimeOut_flg_Inproc/1  "VAPM_RFWhlRotDirTimeOut_flg"
  VAPM_RFWhlRotDirTimeOut_flg_Inproc/1 -> UnitConverter70/1
  UnitConverter70/1 -> VOUTP_RFWhlRotDirTimeOut_flg/1  "VOUTP_RFWhlRotDirTimeOut_flg"
  VAPM_LRWhlRotDir_enum/1 -> VAPM_LRWhlRotDir_enum_Inproc/1  "VAPM_LRWhlRotDir_enum"
  VAPM_LRWhlRotDir_enum_Inproc/1 -> UnitConverter71/1
  UnitConverter71/1 -> VOUTP_LRWhlRotDir_enum/1  "VOUTP_LRWhlRotDir_enum"
  VAPM_LRWhlRotDirTimeOut_flg/1 -> VAPM_LRWhlRotDirTimeOut_flg_Inproc/1  "VAPM_LRWhlRotDirTimeOut_flg"
  VAPM_LRWhlRotDirTimeOut_flg_Inproc/1 -> UnitConverter72/1
  UnitConverter72/1 -> VOUTP_LRWhlRotDirTimeOut_flg/1  "VOUTP_LRWhlRotDirTimeOut_flg"
  VAPM_RRWhlRotDir_enum/1 -> VAPM_RRWhlRotDir_enum_Inproc/1  "VAPM_RRWhlRotDir_enum"
  VAPM_RRWhlRotDir_enum_Inproc/1 -> UnitConverter73/1
  UnitConverter73/1 -> VOUTP_RRWhlRotDir_enum/1  "VOUTP_RRWhlRotDir_enum"
  VAPM_RRWhlRotDirTimeOut_flg/1 -> VAPM_RRWhlRotDirTimeOut_flg_Inproc/1  "VAPM_RRWhlRotDirTimeOut_flg"
  VAPM_RRWhlRotDirTimeOut_flg_Inproc/1 -> UnitConverter74/1
  UnitConverter74/1 -> VOUTP_RRWhlRotDirTimeOut_flg/1  "VOUTP_RRWhlRotDirTimeOut_flg"
  VAPM_LFPulseCountV_flg/1 -> VAPM_LFPulseCountV_flg_Inproc/1  "VAPM_LFPulseCountV_flg"
  VAPM_LFPulseCountV_flg_Inproc/1 -> UnitConverter75/1
  UnitConverter75/1 -> VOUTP_LFPulseCountV_flg/1  "VOUTP_LFPulseCountV_flg"
  VAPM_LFPulseCountVTimeOut_flg/1 -> VAPM_LFPulseCountVTimeOut_flg_Inproc/1  "VAPM_LFPulseCountVTimeOut_flg"
  VAPM_LFPulseCountVTimeOut_flg_Inproc/1 -> UnitConverter76/1
  UnitConverter76/1 -> VOUTP_LFPulseCountVTimeOut_flg/1  "VOUTP_LFPulseCountVTimeOut_flg"
  VAPM_RFPulseCountV_flg/1 -> VAPM_RFPulseCountV_flg_Inproc/1  "VAPM_RFPulseCountV_flg"
  VAPM_RFPulseCountV_flg_Inproc/1 -> UnitConverter77/1
  UnitConverter77/1 -> VOUTP_RFPulseCountV_flg/1  "VOUTP_RFPulseCountV_flg"
  VAPM_RFPulseCountVTimeOut_flg/1 -> VAPM_RFPulseCountVTimeOut_flg_Inproc/1  "VAPM_RFPulseCountVTimeOut_flg"
  VAPM_RFPulseCountVTimeOut_flg_Inproc/1 -> UnitConverter78/1
  UnitConverter78/1 -> VOUTP_RFPulseCountVTimeOut_flg/1  "VOUTP_RFPulseCountVTimeOut_flg"
  VAPM_LRPulseCountV_flg/1 -> VAPM_LRPulseCountV_flg_Inproc/1  "VAPM_LRPulseCountV_flg"
  VAPM_LRPulseCountV_flg_Inproc/1 -> UnitConverter79/1
  UnitConverter79/1 -> VOUTP_LRPulseCountV_flg/1  "VOUTP_LRPulseCountV_flg"
  VAPM_LRPulseCountVTimeOut_flg/1 -> VAPM_LRPulseCountVTimeOut_flg_Inproc/1  "VAPM_LRPulseCountVTimeOut_flg"
  VAPM_LRPulseCountVTimeOut_flg_Inproc/1 -> UnitConverter80/1
  UnitConverter80/1 -> VOUTP_LRPulseCountVTimeOut_flg/1  "VOUTP_LRPulseCountVTimeOut_flg"
  VAPM_RRPulseCountV_flg/1 -> VAPM_RRPulseCountV_flg_Inproc/1  "VAPM_RRPulseCountV_flg"
  VAPM_RRPulseCountV_flg_Inproc/1 -> UnitConverter81/1
  UnitConverter81/1 -> VOUTP_RRPulseCountV_flg/1  "VOUTP_RRPulseCountV_flg"
  VAPM_RRPulseCountVTimeOut_flg/1 -> VAPM_RRPulseCountVTimeOut_flg_Inproc/1  "VAPM_RRPulseCountVTimeOut_flg"
  VAPM_RRPulseCountVTimeOut_flg_Inproc/1 -> UnitConverter82/1
  UnitConverter82/1 -> VOUTP_RRPulseCountVTimeOut_flg/1  "VOUTP_RRPulseCountVTimeOut_flg"
  VAPM_LFPulseCount_enum/1 -> VAPM_LFPulseCount_enum_Inproc/1  "VAPM_LFPulseCount_enum"
  VAPM_LFPulseCount_enum_Inproc/1 -> UnitConverter83/1
  UnitConverter83/1 -> VOUTP_LFPulseCount_enum/1  "VOUTP_LFPulseCount_enum"
  VAPM_LFPulseCountTimeOut_flg/1 -> VAPM_LFPulseCountTimeOut_flg_Inproc/1  "VAPM_LFPulseCountTimeOut_flg"
  VAPM_LFPulseCountTimeOut_flg_Inproc/1 -> UnitConverter84/1
  UnitConverter84/1 -> VOUTP_LFPulseCountTimeOut_flg/1  "VOUTP_LFPulseCountTimeOut_flg"
  VAPM_RFPulseCount_enum/1 -> VAPM_RFPulseCount_enum_Inproc/1  "VAPM_RFPulseCount_enum"
  VAPM_RFPulseCount_enum_Inproc/1 -> UnitConverter85/1
  UnitConverter85/1 -> VOUTP_RFPulseCount_enum/1  "VOUTP_RFPulseCount_enum"
  VAPM_RFPulseCountTimeOut_flg/1 -> VAPM_RFPulseCountTimeOut_flg_Inproc/1  "VAPM_RFPulseCountTimeOut_flg"
  VAPM_RFPulseCountTimeOut_flg_Inproc/1 -> UnitConverter86/1
  UnitConverter86/1 -> VOUTP_RFPulseCountTimeOut_flg/1  "VOUTP_RFPulseCountTimeOut_flg"
  VAPM_LRPulseCount_enum/1 -> VAPM_LRPulseCount_enum_Inproc/1  "VAPM_LRPulseCount_enum"
  VAPM_LRPulseCount_enum_Inproc/1 -> UnitConverter87/1
  UnitConverter87/1 -> VOUTP_LRPulseCount_enum/1  "VOUTP_LRPulseCount_enum"
  VAPM_LRPulseCountTimeOut_flg/1 -> VAPM_LRPulseCountTimeOut_flg_Inproc/1  "VAPM_LRPulseCountTimeOut_flg"
  VAPM_LRPulseCountTimeOut_flg_Inproc/1 -> UnitConverter88/1
  UnitConverter88/1 -> VOUTP_LRPulseCountTimeOut_flg/1  "VOUTP_LRPulseCountTimeOut_flg"
  VAPM_RRPulseCount_enum/1 -> VAPM_RRPulseCount_enum_Inproc/1  "VAPM_RRPulseCount_enum"
  VAPM_RRPulseCount_enum_Inproc/1 -> UnitConverter89/1
  UnitConverter89/1 -> VOUTP_RRPulseCount_enum/1  "VOUTP_RRPulseCount_enum"
  VAPM_RRPulseCountTimeOut_flg/1 -> VAPM_RRPulseCountTimeOut_flg_Inproc/1  "VAPM_RRPulseCountTimeOut_flg"
  VAPM_RRPulseCountTimeOut_flg_Inproc/1 -> UnitConverter90/1
  UnitConverter90/1 -> VOUTP_RRPulseCountTimeOut_flg/1  "VOUTP_RRPulseCountTimeOut_flg"
  VAPM_ShifterHandleCmd_enum/1 -> VAPM_ShifterHandleCmd_enum_Inproc/1  "VAPM_ShifterHandleCmd_enum"
  VAPM_ShifterHandleCmd_enum_Inproc/1 -> UnitConverter91/1
  UnitConverter91/1 -> VOUTP_ShifterHandleCmd_enum/1  "VOUTP_ShifterHandleCmd_enum"
  VAPM_ShifterHandleCmdTimeOut_flg/1 -> VAPM_ShifterHandleCmdTimeOut_flg_Inproc/1  "VAPM_ShifterHandleCmdTimeOut_flg"
  VAPM_ShifterHandleCmdTimeOut_flg_Inproc/1 -> UnitConverter92/1
  UnitConverter92/1 -> VOUTP_ShifterHandleCmdTimeOut_flg/1  "VOUTP_ShifterHandleCmdTimeOut_flg"
  VAPM_DriIntend_enum/1 -> VAPM_DriIntend_enum_Inproc/1  "VAPM_DriIntend_enum"
  VAPM_DriIntend_enum_Inproc/1 -> UnitConverter93/1
  UnitConverter93/1 -> VOUTP_DriIntend_enum/1  "VOUTP_DriIntend_enum"
  VAPM_DriIntendTimeOut_flg/1 -> VAPM_DriIntendTimeOut_flg_Inproc/1  "VAPM_DriIntendTimeOut_flg"
  VAPM_DriIntendTimeOut_flg_Inproc/1 -> UnitConverter94/1
  UnitConverter94/1 -> VOUTP_DriIntendTimeOut_flg/1  "VOUTP_DriIntendTimeOut_flg"
  VAPM_EPSAOIControl_enum/1 -> VAPM_EPSAOIControl_enum_Inproc/1  "VAPM_EPSAOIControl_enum"
  VAPM_EPSAOIControl_enum_Inproc/1 -> UnitConverter95/1
  UnitConverter95/1 -> VOUTP_EPSAOIControl_enum/1  "VOUTP_EPSAOIControl_enum"
  VAPM_EPSAOIControlTimeOut_flg/1 -> VAPM_EPSAOIControlTimeOut_flg_Inproc/1  "VAPM_EPSAOIControlTimeOut_flg"
  VAPM_EPSAOIControlTimeOut_flg_Inproc/1 -> UnitConverter96/1
  UnitConverter96/1 -> VOUTP_EPSAOIControlTimeOut_flg/1  "VOUTP_EPSAOIControlTimeOut_flg"
  VAPM_SASAngle_Deg/1 -> VAPM_SASAngle_Deg_Inproc/1  "VAPM_SASAngle_Deg"
  VAPM_SASAngle_Deg_Inproc/1 -> UnitConverter97/1
  UnitConverter97/1 -> VOUTP_SASAngle_Deg/1  "VOUTP_SASAngle_Deg"
  VAPM_SASAngleTimeOut_flg/1 -> VAPM_SASAngleTimeOut_flg_Inproc/1  "VAPM_SASAngleTimeOut_flg"
  VAPM_SASAngleTimeOut_flg_Inproc/1 -> UnitConverter98/1
  UnitConverter98/1 -> VOUTP_SASAngleTimeOut_flg/1  "VOUTP_SASAngleTimeOut_flg"
  VAPM_SASSpeed_degps/1 -> VAPM_SASSpeed_degps_Inproc/1  "VAPM_SASSpeed_degps"
  VAPM_SASSpeed_degps_Inproc/1 -> UnitConverter99/1
  UnitConverter99/1 -> VOUTP_SASSpeed_degps/1  "VOUTP_SASSpeed_degps"
  VAPM_SASSpeedTimeOut_flg/1 -> VAPM_SASSpeedTimeOut_flg_Inproc/1  "VAPM_SASSpeedTimeOut_flg"
  VAPM_SASSpeedTimeOut_flg_Inproc/1 -> UnitConverter100/1
  UnitConverter100/1 -> VOUTP_SASSpeedTimeOut_flg/1  "VOUTP_SASSpeedTimeOut_flg"
  VAPM_SASSpeedValid_flg/1 -> VAPM_SASSpeedValid_flg_Inproc/1  "VAPM_SASSpeedValid_flg"
  VAPM_SASSpeedValid_flg_Inproc/1 -> UnitConverter101/1
  UnitConverter101/1 -> VOUTP_SASSpeedValid_flg/1  "VOUTP_SASSpeedValid_flg"
  VAPM_SASSpeedValidTimeOut_flg/1 -> VAPM_SASSpeedValidTimeOut_flg_Inproc/1  "VAPM_SASSpeedValidTimeOut_flg"
  VAPM_SASSpeedValidTimeOut_flg_Inproc/1 -> UnitConverter102/1
  UnitConverter102/1 -> VOUTP_SASSpeedValidTimeOut_flg/1  "VOUTP_SASSpeedValidTimeOut_flg"
  VAPM_SASCAL_flg/1 -> VAPM_SASCAL_flg_Inproc/1  "VAPM_SASCAL_flg"
  VAPM_SASCAL_flg_Inproc/1 -> UnitConverter103/1
  UnitConverter103/1 -> VOUTP_SASCAL_flg/1  "VOUTP_SASCAL_flg"
  VAPM_SASCALTimeOut_flg/1 -> VAPM_SASCALTimeOut_flg_Inproc/1  "VAPM_SASCALTimeOut_flg"
  VAPM_SASCALTimeOut_flg_Inproc/1 -> UnitConverter104/1
  UnitConverter104/1 -> VOUTP_SASCALTimeOut_flg/1  "VOUTP_SASCALTimeOut_flg"
  VAPM_SASV_flg/1 -> VAPM_SASV_flg_Inproc/1  "VAPM_SASV_flg"
  VAPM_SASV_flg_Inproc/1 -> UnitConverter105/1
  UnitConverter105/1 -> VOUTP_SASV_flg/1  "VOUTP_SASV_flg"
  VAPM_SASVTimeOut_flg/1 -> VAPM_SASVTimeOut_flg_Inproc/1  "VAPM_SASVTimeOut_flg"
  VAPM_SASVTimeOut_flg_Inproc/1 -> UnitConverter106/1
  UnitConverter106/1 -> VOUTP_SASVTimeOut_flg/1  "VOUTP_SASVTimeOut_flg"
  VAPM_GRADE_Deg/1 -> VAPM_GRADE_Deg_Inproc/1  "VAPM_GRADE_Deg"
  VAPM_GRADE_Deg_Inproc/1 -> UnitConverter107/1
  UnitConverter107/1 -> VOUTP_GRADE_Deg/1  "VOUTP_GRADE_Deg"
  VAPM_GRADETimeOut_flg/1 -> VAPM_GRADETimeOut_flg_Inproc/1  "VAPM_GRADETimeOut_flg"
  VAPM_GRADETimeOut_flg_Inproc/1 -> UnitConverter108/1
  UnitConverter108/1 -> VOUTP_GRADETimeOut_flg/1  "VOUTP_GRADETimeOut_flg"
  VAPM_YawRate_degps/1 -> VAPM_YawRate_degps_Inproc/1  "VAPM_YawRate_degps"
  VAPM_YawRate_degps_Inproc/1 -> UnitConverter109/1
  UnitConverter109/1 -> VOUTP_YawRate_degps/1  "VOUTP_YawRate_degps"
  VAPM_YawRateTimeOut_flg/1 -> VAPM_YawRateTimeOut_flg_Inproc/1  "VAPM_YawRateTimeOut_flg"
  VAPM_YawRateTimeOut_flg_Inproc/1 -> UnitConverter110/1
  UnitConverter110/1 -> VOUTP_YawRateTimeOut_flg/1  "VOUTP_YawRateTimeOut_flg"
  VAPM_LatAccel_Gps/1 -> VAPM_LatAccel_Gps_Inproc/1  "VAPM_LatAccel_Gps"
  VAPM_LatAccel_Gps_Inproc/1 -> UnitConverter111/1
  UnitConverter111/1 -> VOUTP_LatAccel_Gps/1  "VOUTP_LatAccel_Gps"
  VAPM_LatAccelTimeOut_flg/1 -> VAPM_LatAccelTimeOut_flg_Inproc/1  "VAPM_LatAccelTimeOut_flg"
  VAPM_LatAccelTimeOut_flg_Inproc/1 -> UnitConverter112/1
  UnitConverter112/1 -> VOUTP_LatAccelTimeOut_flg/1  "VOUTP_LatAccelTimeOut_flg"
  VAPM_LongAccel_Gps/1 -> VAPM_LongAccel_Gps_Inproc/1  "VAPM_LongAccel_Gps"
  VAPM_LongAccel_Gps_Inproc/1 -> UnitConverter113/1
  UnitConverter113/1 -> VOUTP_LongAccel_Gps/1  "VOUTP_LongAccel_Gps"
  VAPM_LongAccelTimeOut_flg/1 -> VAPM_LongAccelTimeOut_flg_Inproc/1  "VAPM_LongAccelTimeOut_flg"
  VAPM_LongAccelTimeOut_flg_Inproc/1 -> UnitConverter114/1
  UnitConverter114/1 -> VOUTP_LongAccelTimeOut_flg/1  "VOUTP_LongAccelTimeOut_flg"
  VAPM_MCPressure_bar/1 -> VAPM_MCPressure_bar_Inproc/1  "VAPM_MCPressure_bar"
  VAPM_MCPressure_bar_Inproc/1 -> UnitConverter115/1
  UnitConverter115/1 -> VOUTP_MCPressure_bar/1  "VOUTP_MCPressure_bar"
  VAPM_MCPressureTimeOut_flg/1 -> VAPM_MCPressureTimeOut_flg_Inproc/1  "VAPM_MCPressureTimeOut_flg"
  VAPM_MCPressureTimeOut_flg_Inproc/1 -> UnitConverter116/1
  UnitConverter116/1 -> VOUTP_MCPressureTimeOut_flg/1  "VOUTP_MCPressureTimeOut_flg"
  VAPM_YawRateV_flg/1 -> VAPM_YawRateV_flg_Inproc/1  "VAPM_YawRateV_flg"
  VAPM_YawRateV_flg_Inproc/1 -> UnitConverter117/1
  UnitConverter117/1 -> VOUTP_YawRateV_flg/1  "VOUTP_YawRateV_flg"
  VAPM_YawRateVTimeOut_flg/1 -> VAPM_YawRateVTimeOut_flg_Inproc/1  "VAPM_YawRateVTimeOut_flg"
  VAPM_YawRateVTimeOut_flg_Inproc/1 -> UnitConverter118/1
  UnitConverter118/1 -> VOUTP_YawRateVTimeOut_flg/1  "VOUTP_YawRateVTimeOut_flg"
  VAPM_LatAccelV_flg/1 -> VAPM_LatAccelV_flg_Inproc/1  "VAPM_LatAccelV_flg"
  VAPM_LatAccelV_flg_Inproc/1 -> UnitConverter119/1
  UnitConverter119/1 -> VOUTP_LatAccelV_flg/1  "VOUTP_LatAccelV_flg"
  VAPM_LatAccelVTimeOut_flg/1 -> VAPM_LatAccelVTimeOut_flg_Inproc/1  "VAPM_LatAccelVTimeOut_flg"
  VAPM_LatAccelVTimeOut_flg_Inproc/1 -> UnitConverter120/1
  UnitConverter120/1 -> VOUTP_LatAccelVTimeOut_flg/1  "VOUTP_LatAccelVTimeOut_flg"
  VAPM_LongAccelV_flg/1 -> VAPM_LongAccelV_flg_Inproc/1  "VAPM_LongAccelV_flg"
  VAPM_LongAccelV_flg_Inproc/1 -> UnitConverter121/1
  UnitConverter121/1 -> VOUTP_LongAccelV_flg/1  "VOUTP_LongAccelV_flg"
  VAPM_LongAccelVTimeOut_flg/1 -> VAPM_LongAccelVTimeOut_flg_Inproc/1  "VAPM_LongAccelVTimeOut_flg"
  VAPM_LongAccelVTimeOut_flg_Inproc/1 -> UnitConverter122/1
  UnitConverter122/1 -> VOUTP_LongAccelVTimeOut_flg/1  "VOUTP_LongAccelVTimeOut_flg"
  VAPM_MCPressureV_bar/1 -> VAPM_MCPressureV_bar_Inproc/1  "VAPM_MCPressureV_bar"
  VAPM_MCPressureV_bar_Inproc/1 -> UnitConverter123/1
  UnitConverter123/1 -> VOUTP_MCPressureV_bar/1  "VOUTP_MCPressureV_bar"
  VAPM_MCPressureVTimeOut_flg/1 -> VAPM_MCPressureVTimeOut_flg_Inproc/1  "VAPM_MCPressureVTimeOut_flg"
  VAPM_MCPressureVTimeOut_flg_Inproc/1 -> UnitConverter124/1
  UnitConverter124/1 -> VOUTP_MCPressureVTimeOut_flg/1  "VOUTP_MCPressureVTimeOut_flg"
  VAPM_BrkSwSta_flg/1 -> VAPM_BrkSwSta_flg_Inproc/1  "VAPM_BrkSwSta_flg"
  VAPM_BrkSwSta_flg_Inproc/1 -> UnitConverter125/1
  UnitConverter125/1 -> VOUTP_BrkSwSta_flg/1  "VOUTP_BrkSwSta_flg"
  VAPM_BrkSwStaTimeOut_flg/1 -> VAPM_BrkSwStaTimeOut_flg_Inproc/1  "VAPM_BrkSwStaTimeOut_flg"
  VAPM_BrkSwStaTimeOut_flg_Inproc/1 -> UnitConverter126/1
  UnitConverter126/1 -> VOUTP_BrkSwStaTimeOut_flg/1  "VOUTP_BrkSwStaTimeOut_flg"
  VAPM_BrkSwV_flg/1 -> VAPM_BrkSwV_flg_Inproc/1  "VAPM_BrkSwV_flg"
  VAPM_BrkSwV_flg_Inproc/1 -> UnitConverter127/1
  UnitConverter127/1 -> VOUTP_BrkSwV_flg/1  "VOUTP_BrkSwV_flg"
  VAPM_BrkSwVTimeOut_flg/1 -> VAPM_BrkSwVTimeOut_flg_Inproc/1  "VAPM_BrkSwVTimeOut_flg"
  VAPM_BrkSwVTimeOut_flg_Inproc/1 -> UnitConverter128/1
  UnitConverter128/1 -> VOUTP_BrkSwVTimeOut_flg/1  "VOUTP_BrkSwVTimeOut_flg"
  VAPM_ESCStandstill_flg/1 -> VAPM_ESCStandstill_flg_Inproc/1  "VAPM_ESCStandstill_flg"
  VAPM_ESCStandstill_flg_Inproc/1 -> UnitConverter129/1
  UnitConverter129/1 -> VOUTP_ESCStandstill_flg/1  "VOUTP_ESCStandstill_flg"
  VAPM_ESCStandstillTimeOut_flg/1 -> VAPM_ESCStandstillTimeOut_flg_Inproc/1  "VAPM_ESCStandstillTimeOut_flg"
  VAPM_ESCStandstillTimeOut_flg_Inproc/1 -> UnitConverter130/1
  UnitConverter130/1 -> VOUTP_ESCStandstillTimeOut_flg/1  "VOUTP_ESCStandstillTimeOut_flg"
  VAPM_ESCAPSSta_enum/1 -> VAPM_ESCAPSSta_enum_Inproc/1  "VAPM_ESCAPSSta_enum"
  VAPM_ESCAPSSta_enum_Inproc/1 -> UnitConverter131/1
  UnitConverter131/1 -> VOUTP_ESCAPSSta_enum/1  "VOUTP_ESCAPSSta_enum"
  VAPM_ESCAPSStaTimeOut_flg/1 -> VAPM_ESCAPSStaTimeOut_flg_Inproc/1  "VAPM_ESCAPSStaTimeOut_flg"
  VAPM_ESCAPSStaTimeOut_flg_Inproc/1 -> UnitConverter132/1
  UnitConverter132/1 -> VOUTP_ESCAPSStaTimeOut_flg/1  "VOUTP_ESCAPSStaTimeOut_flg"
  VAPM_EPBExtReleaseAvail_flg/1 -> VAPM_EPBExtReleaseAvail_flg_Inproc/1  "VAPM_EPBExtReleaseAvail_flg"
  VAPM_EPBExtReleaseAvail_flg_Inproc/1 -> UnitConverter133/1
  UnitConverter133/1 -> VOUTP_EPBExtReleaseAvail_flg/1  "VOUTP_EPBExtReleaseAvail_flg"
  VAPM_EPBExtReleaseAvailTimeOut_flg/1 -> VAPM_EPBExtReleaseAvailTimeOut_flg_Inproc/1  "VAPM_EPBExtReleaseAvailTimeOut_flg"
  VAPM_EPBExtReleaseAvailTimeOut_flg_Inproc/1 -> UnitConverter134/1
  UnitConverter134/1 -> VOUTP_EPBExtReleaseAvailTimeOut_flg/1  "VOUTP_EPBExtReleaseAvailTimeOut_flg"
  VAPM_EPBExtApplyAvail_flg/1 -> VAPM_EPBExtApplyAvail_flg_Inproc/1  "VAPM_EPBExtApplyAvail_flg"
  VAPM_EPBExtApplyAvail_flg_Inproc/1 -> UnitConverter135/1
  UnitConverter135/1 -> VOUTP_EPBExtApplyAvail_flg/1  "VOUTP_EPBExtApplyAvail_flg"
  VAPM_EPBExtApplyAvailTimeOut_flg/1 -> VAPM_EPBExtApplyAvailTimeOut_flg_Inproc/1  "VAPM_EPBExtApplyAvailTimeOut_flg"
  VAPM_EPBExtApplyAvailTimeOut_flg_Inproc/1 -> UnitConverter136/1
  UnitConverter136/1 -> VOUTP_EPBExtApplyAvailTimeOut_flg/1  "VOUTP_EPBExtApplyAvailTimeOut_flg"
  VAPM_EPBErrSta_enum/1 -> VAPM_EPBErrSta_enum_Inproc/1  "VAPM_EPBErrSta_enum"
  VAPM_EPBErrSta_enum_Inproc/1 -> UnitConverter137/1
  UnitConverter137/1 -> VOUTP_EPBErrSta_enum/1  "VOUTP_EPBErrSta_enum"
  VAPM_EPBErrStaTimeOut_flg/1 -> VAPM_EPBErrStaTimeOut_flg_Inproc/1  "VAPM_EPBErrStaTimeOut_flg"
  VAPM_EPBErrStaTimeOut_flg_Inproc/1 -> UnitConverter138/1
  UnitConverter138/1 -> VOUTP_EPBErrStaTimeOut_flg/1  "VOUTP_EPBErrStaTimeOut_flg"
  VAPM_EPBSta_enum/1 -> VAPM_EPBSta_enum_Inproc/1  "VAPM_EPBSta_enum"
  VAPM_EPBSta_enum_Inproc/1 -> UnitConverter139/1
  UnitConverter139/1 -> VOUTP_EPBSta_enum/1  "VOUTP_EPBSta_enum"
  VAPM_EPBStaTimeOut_flg/1 -> VAPM_EPBStaTimeOut_flg_Inproc/1  "VAPM_EPBStaTimeOut_flg"
  VAPM_EPBStaTimeOut_flg_Inproc/1 -> UnitConverter140/1
  UnitConverter140/1 -> VOUTP_EPBStaTimeOut_flg/1  "VOUTP_EPBStaTimeOut_flg"
  VAPM_AVMparkingcancel_enum/1 -> VAPM_AVMparkingcancel_enum_Inproc/1  "VAPM_AVMparkingcancel_enum"
  VAPM_AVMparkingcancel_enum_Inproc/1 -> UnitConverter141/1
  UnitConverter141/1 -> VOUTP_AVMparkingcancel_enum/1  "VOUTP_AVMparkingcancel_enum"
  VAPM_AVMparkingcancelTimeOut_flg/1 -> VAPM_AVMparkingcancelTimeOut_flg_Inproc/1  "VAPM_AVMparkingcancelTimeOut_flg"
  VAPM_AVMparkingcancelTimeOut_flg_Inproc/1 -> UnitConverter142/1
  UnitConverter142/1 -> VOUTP_AVMparkingcancelTimeOut_flg/1  "VOUTP_AVMparkingcancelTimeOut_flg"
  VAPM_AVMparkingexcute_enum/1 -> VAPM_AVMparkingexcute_enum_Inproc/1  "VAPM_AVMparkingexcute_enum"
  VAPM_AVMparkingexcute_enum_Inproc/1 -> UnitConverter143/1
  UnitConverter143/1 -> VOUTP_AVMparkingexcute_enum/1  "VOUTP_AVMparkingexcute_enum"
  VAPM_AVMparkingexcuteTimeOut_flg/1 -> VAPM_AVMparkingexcuteTimeOut_flg_Inproc/1  "VAPM_AVMparkingexcuteTimeOut_flg"
  VAPM_AVMparkingexcuteTimeOut_flg_Inproc/1 -> UnitConverter144/1
  UnitConverter144/1 -> VOUTP_AVMparkingexcuteTimeOut_flg/1  "VOUTP_AVMparkingexcuteTimeOut_flg"
  VAPM_AVMParkingmode_enum/1 -> VAPM_AVMParkingmode_enum_Inproc/1  "VAPM_AVMParkingmode_enum"
  VAPM_AVMParkingmode_enum_Inproc/1 -> UnitConverter145/1
  UnitConverter145/1 -> VOUTP_AVMParkingmode_enum/1  "VOUTP_AVMParkingmode_enum"
  VAPM_AVMParkingmodeTimeOut_flg/1 -> VAPM_AVMParkingmodeTimeOut_flg_Inproc/1  "VAPM_AVMParkingmodeTimeOut_flg"
  VAPM_AVMParkingmodeTimeOut_flg_Inproc/1 -> UnitConverter146/1
  UnitConverter146/1 -> VOUTP_AVMParkingmodeTimeOut_flg/1  "VOUTP_AVMParkingmodeTimeOut_flg"
  VAPM_AVMErrSTA_flg/1 -> VAPM_AVMErrSTA_flg_Inproc/1  "VAPM_AVMErrSTA_flg"
  VAPM_AVMErrSTA_flg_Inproc/1 -> UnitConverter147/1
  UnitConverter147/1 -> VOUTP_AVMErrSTA_flg/1  "VOUTP_AVMErrSTA_flg"
  VAPM_AVMErrSTATimeOut_flg/1 -> VAPM_AVMErrSTATimeOut_flg_Inproc/1  "VAPM_AVMErrSTATimeOut_flg"
  VAPM_AVMErrSTATimeOut_flg_Inproc/1 -> UnitConverter148/1
  UnitConverter148/1 -> VOUTP_AVMErrSTATimeOut_flg/1  "VOUTP_AVMErrSTATimeOut_flg"
  VAPM_IVIStatus_flg/1 -> VAPM_IVIStatus_flg_Inproc/1  "VAPM_IVIStatus_flg"
  VAPM_IVIStatus_flg_Inproc/1 -> UnitConverter149/1
  UnitConverter149/1 -> VOUTP_IVIStatus_flg/1  "VOUTP_IVIStatus_flg"
  VAPM_IVIStatusTimeOut_flg/1 -> VAPM_IVIStatusTimeOut_flg_Inproc/1  "VAPM_IVIStatusTimeOut_flg"
  VAPM_IVIStatusTimeOut_flg_Inproc/1 -> UnitConverter150/1
  UnitConverter150/1 -> VOUTP_IVIStatusTimeOut_flg/1  "VOUTP_IVIStatusTimeOut_flg"
  VAPM_CAASSw_enum/1 -> VAPM_CAASSw_enum_Inproc/1  "VAPM_CAASSw_enum"
  VAPM_CAASSw_enum_Inproc/1 -> UnitConverter151/1
  UnitConverter151/1 -> VOUTP_CAASSw_enum/1  "VOUTP_CAASSw_enum"
  VAPM_CAASSwTimeOut_flg/1 -> VAPM_CAASSwTimeOut_flg_Inproc/1  "VAPM_CAASSwTimeOut_flg"
  VAPM_CAASSwTimeOut_flg_Inproc/1 -> UnitConverter152/1
  UnitConverter152/1 -> VOUTP_CAASSwTimeOut_flg/1  "VOUTP_CAASSwTimeOut_flg"
  VAPM_IVIScreen_enum/1 -> VAPM_IVIScreen_enum_Inproc/1  "VAPM_IVIScreen_enum"
  VAPM_IVIScreen_enum_Inproc/1 -> UnitConverter153/1
  UnitConverter153/1 -> VOUTP_IVIScreen_enum/1  "VOUTP_IVIScreen_enum"
  VAPM_IVIScreenTimeOut_flg/1 -> VAPM_IVIScreenTimeOut_flg_Inproc/1  "VAPM_IVIScreenTimeOut_flg"
  VAPM_IVIScreenTimeOut_flg_Inproc/1 -> UnitConverter154/1
  UnitConverter154/1 -> VOUTP_IVIScreenTimeOut_flg/1  "VOUTP_IVIScreenTimeOut_flg"
  VAPM_ABSActiveToAPM_flg/1 -> VAPM_ABSActiveToAPM_flg_Inproc/1  "VAPM_ABSActiveToAPM_flg"
  VAPM_ABSActiveToAPM_flg_Inproc/1 -> UnitConverter155/1
  UnitConverter155/1 -> VOUTP_ABSActiveToAPM_flg/1  "VOUTP_ABSActiveToAPM_flg"
  VAPM_ABSActiveTimeOut_flg/1 -> VAPM_ABSActiveTimeOut_flg_Inproc/1  "VAPM_ABSActiveTimeOut_flg"
  VAPM_ABSActiveTimeOut_flg_Inproc/1 -> UnitConverter156/1
  UnitConverter156/1 -> VOUTP_ABSActiveTimeOut_flg/1  "VOUTP_ABSActiveTimeOut_flg"
  VAPM_TCSActiveToAPM_flg/1 -> VAPM_TCSActiveToAPM_flg_Inproc/1  "VAPM_TCSActiveToAPM_flg"
  VAPM_TCSActiveToAPM_flg_Inproc/1 -> UnitConverter157/1
  UnitConverter157/1 -> VOUTP_TCSActiveToAPM_flg/1  "VOUTP_TCSActiveToAPM_flg"
  VAPM_TCSActiveTimeOut_flg/1 -> VAPM_TCSActiveTimeOut_flg_Inproc/1  "VAPM_TCSActiveTimeOut_flg"
  VAPM_TCSActiveTimeOut_flg_Inproc/1 -> UnitConverter158/1
  UnitConverter158/1 -> VOUTP_TCSActiveTimeOut_flg/1  "VOUTP_TCSActiveTimeOut_flg"
  VAPM_DriverSeatBeltCmd_flg/1 -> VAPM_DriverSeatBeltCmd_flg_Inproc/1  "VAPM_DriverSeatBeltCmd_flg"
  VAPM_DriverSeatBeltCmd_flg_Inproc/1 -> UnitConverter159/1
  UnitConverter159/1 -> VOUTP_DriverSeatBeltCmd_flg/1  "VOUTP_DriverSeatBeltCmd_flg"
  VAPM_DriverSeatBeltCmdTimeOut_flg/1 -> VAPM_DriverSeatBeltCmdTimeOut_flg_Inproc/1  "VAPM_DriverSeatBeltCmdTimeOut_flg"
  VAPM_DriverSeatBeltCmdTimeOut_flg_Inproc/1 -> UnitConverter160/1
  UnitConverter160/1 -> VOUTP_DriverSeatBeltCmdTimeOut_flg/1  "VOUTP_DriverSeatBeltCmdTimeOut_flg"
  VAPM_APSProgressPCT_pct/1 -> VAPM_APSProgressPCT_pct_Inproc/1  "VAPM_APSProgressPCT_pct"
  VAPM_APSProgressPCT_pct_Inproc/1 -> UnitConverter161/1
  UnitConverter161/1 -> VOUTP_APSProgressPCT_pct/1  "VOUTP_APSProgressPCT_pct"
  VAPM_APSRQDisplay_enum/1 -> VAPM_APSRQDisplay_enum_Inproc/1  "VAPM_APSRQDisplay_enum"
  VAPM_APSRQDisplay_enum_Inproc/1 -> UnitConverter162/1
  UnitConverter162/1 -> VOUTP_APSRQDisplay_enum/1  "VOUTP_APSRQDisplay_enum"
  VAPM_APSSWVer_enum/1 -> VAPM_APSSWVer_enum_Inproc/1  "VAPM_APSSWVer_enum"
  VAPM_APSSWVer_enum_Inproc/1 -> UnitConverter163/1
  UnitConverter163/1 -> VOUTP_APSSWVer_enum/1  "VOUTP_APSSWVer_enum"
  VAPM_APSHWVer_enum/1 -> VAPM_APSHWVer_enum_Inproc/1  "VAPM_APSHWVer_enum"
  VAPM_APSHWVer_enum_Inproc/1 -> UnitConverter164/1
  UnitConverter164/1 -> VOUTP_APSHWVer_enum/1  "VOUTP_APSHWVer_enum"
  VAPM_APSExitCondition_enum/1 -> VAPM_APSExitCondition_enum_Inproc/1  "VAPM_APSExitCondition_enum"
  VAPM_APSExitCondition_enum_Inproc/1 -> UnitConverter165/1
  UnitConverter165/1 -> VOUTP_APSExitCondition_enum/1  "VOUTP_APSExitCondition_enum"
  VAPM_APSAngleTarget_Deg/1 -> VAPM_APSAngleTarget_Deg_Inproc/1  "VAPM_APSAngleTarget_Deg"
  VAPM_APSAngleTarget_Deg_Inproc/1 -> UnitConverter166/1
  UnitConverter166/1 -> VOUTP_APSAngleTarget_Deg/1  "VOUTP_APSAngleTarget_Deg"
  VAPM_APSVRqEPASCtrl_flg/1 -> VAPM_APSVRqEPASCtrl_flg_Inproc/1  "VAPM_APSVRqEPASCtrl_flg"
  VAPM_APSVRqEPASCtrl_flg_Inproc/1 -> UnitConverter167/1
  UnitConverter167/1 -> VOUTP_APSVRqEPASCtrl_flg/1  "VOUTP_APSVRqEPASCtrl_flg"
  VAPM_APSRqEPASCtrl_flg/1 -> VAPM_APSRqEPASCtrl_flg_Inproc/1  "VAPM_APSRqEPASCtrl_flg"
  VAPM_APSRqEPASCtrl_flg_Inproc/1 -> UnitConverter168/1
  UnitConverter168/1 -> VOUTP_APSRqEPASCtrl_flg/1  "VOUTP_APSRqEPASCtrl_flg"
  VAPM_CAASSta_enum/1 -> VAPM_CAASSta_enum_Inproc/1  "VAPM_CAASSta_enum"
  VAPM_CAASSta_enum_Inproc/1 -> UnitConverter169/1
  UnitConverter169/1 -> VOUTP_CAASSta_enum/1  "VOUTP_CAASSta_enum"
  VBCM_HornCtrl_flg/1 -> VBCM_HornCtrl_flg_Inproc/1  "VBCM_HornCtrl_flg"
  VBCM_HornCtrl_flg_Inproc/1 -> UnitConverter170/1
  UnitConverter170/1 -> VOUTP_HornCtrl_flg/1  "VOUTP_HornCtrl_flg"
  VBCM_FRHaltBrakeSta_enum/1 -> VBCM_FRHaltBrakeSta_enum_Inproc/1  "VBCM_FRHaltBrakeSta_enum"
  VBCM_FRHaltBrakeSta_enum_Inproc/1 -> UnitConverter171/1
  UnitConverter171/1 -> VOUTP_FRHaltBrakeSta_enum/1  "VOUTP_FRHaltBrakeSta_enum"
  VBCM_FRDisIntEmCmd_flg/1 -> VBCM_FRDisIntEmCmd_flg_Inproc/1  "VBCM_FRDisIntEmCmd_flg"
  VBCM_FRDisIntEmCmd_flg_Inproc/1 -> UnitConverter172/1
  UnitConverter172/1 -> VOUTP_FRDisIntEmCmd_flg/1  "VOUTP_FRDisIntEmCmd_flg"
  VBCM_FROpenClosePBCmd_enum/1 -> VBCM_FROpenClosePBCmd_enum_Inproc/1  "VBCM_FROpenClosePBCmd_enum"
  VBCM_FROpenClosePBCmd_enum_Inproc/1 -> UnitConverter173/1
  UnitConverter173/1 -> VOUTP_FROpenClosePBCmd_enum/1  "VOUTP_FROpenClosePBCmd_enum"
  VBCM_DoorStaSta_enum/1 -> VBCM_DoorStaSta_enum_Inproc/1  "VBCM_DoorStaSta_enum"
  VBCM_DoorStaSta_enum_Inproc/1 -> UnitConverter174/1
  UnitConverter174/1 -> VOUTP_DoorStaSta_enum/1  "VOUTP_DoorStaSta_enum"
  VBCM_BrakeLamp_flg/1 -> VBCM_BrakeLamp_flg_Inproc/1  "VBCM_BrakeLamp_flg"
  VBCM_BrakeLamp_flg_Inproc/1 -> UnitConverter175/1
  UnitConverter175/1 -> VOUTP_BrakeLamp_flg/1  "VOUTP_BrakeLamp_flg"
  VBCM_LDRL_flg/1 -> VBCM_LDRL_flg_Inproc/1  "VBCM_LDRL_flg"
  VBCM_LDRL_flg_Inproc/1 -> UnitConverter176/1
  UnitConverter176/1 -> VOUTP_LDRL_flg/1  "VOUTP_LDRL_flg"
  VBCM_RDRL_flg/1 -> VBCM_RDRL_flg_Inproc/1  "VBCM_RDRL_flg"
  VBCM_RDRL_flg_Inproc/1 -> UnitConverter177/1
  UnitConverter177/1 -> VOUTP_RDRL_flg/1  "VOUTP_RDRL_flg"
  VBCM_ReverseLamp_flg/1 -> VBCM_ReverseLamp_flg_Inproc/1  "VBCM_ReverseLamp_flg"
  VBCM_ReverseLamp_flg_Inproc/1 -> UnitConverter178/1
  UnitConverter178/1 -> VOUTP_ReverseLamp_flg/1  "VOUTP_ReverseLamp_flg"
  VBCM_RrFogLamp_flg/1 -> VBCM_RrFogLamp_flg_Inproc/1  "VBCM_RrFogLamp_flg"
  VBCM_RrFogLamp_flg_Inproc/1 -> UnitConverter179/1
  UnitConverter179/1 -> VOUTP_RrFogLamp_flg/1  "VOUTP_RrFogLamp_flg"
  VBCM_HBeam_flg/1 -> VBCM_HBeam_flg_Inproc/1  "VBCM_HBeam_flg"
  VBCM_HBeam_flg_Inproc/1 -> UnitConverter180/1
  UnitConverter180/1 -> VOUTP_HBeam_flg/1  "VOUTP_HBeam_flg"
  VBCM_LBeam_flg/1 -> VBCM_LBeam_flg_Inproc/1  "VBCM_LBeam_flg"
  VBCM_LBeam_flg_Inproc/1 -> UnitConverter181/1
  UnitConverter181/1 -> VOUTP_LBeam_flg/1  "VOUTP_LBeam_flg"
  VBCM_PosLamp_flg/1 -> VBCM_PosLamp_flg_Inproc/1  "VBCM_PosLamp_flg"
  VBCM_PosLamp_flg_Inproc/1 -> UnitConverter182/1
  UnitConverter182/1 -> VOUTP_PosLamp_flg/1  "VOUTP_PosLamp_flg"
  VBCM_HazardSW_flg/1 -> VBCM_HazardSW_flg_Inproc/1  "VBCM_HazardSW_flg"
  VBCM_HazardSW_flg_Inproc/1 -> UnitConverter183/1
  UnitConverter183/1 -> VOUTP_HazardSW_flg/1  "VOUTP_HazardSW_flg"
  VBCM_LTurnLP_flg/1 -> VBCM_LTurnLP_flg_Inproc/1  "VBCM_LTurnLP_flg"
  VBCM_LTurnLP_flg_Inproc/1 -> UnitConverter184/1
  UnitConverter184/1 -> VOUTP_LTurnLP_flg/1  "VOUTP_LTurnLP_flg"
  VBCM_RTurnLP_flg/1 -> VBCM_RTurnLP_flg_Inproc/1  "VBCM_RTurnLP_flg"
  VBCM_RTurnLP_flg_Inproc/1 -> UnitConverter185/1
  UnitConverter185/1 -> VOUTP_RTurnLP_flg/1  "VOUTP_RTurnLP_flg"
  VBCM_LSMLPCmd_flg/1 -> VBCM_LSMLPCmd_flg_Inproc/1  "VBCM_LSMLPCmd_flg"
  VBCM_LSMLPCmd_flg_Inproc/1 -> UnitConverter186/1
  UnitConverter186/1 -> VOUTP_LSMLPCmd_flg/1  "VOUTP_LSMLPCmd_flg"
  VBCM_RSMLPCmd_flg/1 -> VBCM_RSMLPCmd_flg_Inproc/1  "VBCM_RSMLPCmd_flg"
  VBCM_RSMLPCmd_flg_Inproc/1 -> UnitConverter187/1
  UnitConverter187/1 -> VOUTP_RSMLPCmd_flg/1  "VOUTP_RSMLPCmd_flg"
  VBCM_TurnLpLActiveCmd_flg/1 -> VBCM_TurnLpLActiveCmd_flg_Inproc/1  "VBCM_TurnLpLActiveCmd_flg"
  VBCM_TurnLpLActiveCmd_flg_Inproc/1 -> UnitConverter188/1
  UnitConverter188/1 -> VOUTP_TurnLpLActiveCmd_flg/1  "VOUTP_TurnLpLActiveCmd_flg"
  VBCM_TurnLpRActiveCmd_flg/1 -> VBCM_TurnLpRActiveCmd_flg_Inproc/1  "VBCM_TurnLpRActiveCmd_flg"
  VBCM_TurnLpRActiveCmd_flg_Inproc/1 -> UnitConverter189/1
  UnitConverter189/1 -> VOUTP_TurnLpRActiveCmd_flg/1  "VOUTP_TurnLpRActiveCmd_flg"
  VBCM_BBuzzerCmd_flg/1 -> VBCM_BBuzzerCmd_flg_Inproc/1  "VBCM_BBuzzerCmd_flg"
  VBCM_BBuzzerCmd_flg_Inproc/1 -> UnitConverter190/1
  UnitConverter190/1 -> VOUTP_BBuzzerCmd_flg/1  "VOUTP_BBuzzerCmd_flg"
  VBCM_FrWiperL_flg/1 -> VBCM_FrWiperL_flg_Inproc/1  "VBCM_FrWiperL_flg"
  VBCM_FrWiperL_flg_Inproc/1 -> UnitConverter191/1
  UnitConverter191/1 -> VOUTP_FrWiperL_flg/1  "VOUTP_FrWiperL_flg"
  VBCM_FrWiperH_flg/1 -> VBCM_FrWiperH_flg_Inproc/1  "VBCM_FrWiperH_flg"
  VBCM_FrWiperH_flg_Inproc/1 -> UnitConverter192/1
  UnitConverter192/1 -> VOUTP_FrWiperH_flg/1  "VOUTP_FrWiperH_flg"
  VBCM_WasherCtrl_enum/1 -> VBCM_WasherCtrl_enum_Inproc/1  "VBCM_WasherCtrl_enum"
  VBCM_WasherCtrl_enum_Inproc/1 -> UnitConverter193/1
  UnitConverter193/1 -> VOUTP_WasherCtrl_enum/1  "VOUTP_WasherCtrl_enum"
  VBCM_RrRmLampBrightCmd_enum/1 -> VBCM_RrRmLampBrightCmd_enum_Inproc/1  "VBCM_RrRmLampBrightCmd_enum"
  VBCM_RrRmLampBrightCmd_enum_Inproc/1 -> UnitConverter194/1
  UnitConverter194/1 -> VOUTP_RrRmLampBrightCmd_enum/1  "VOUTP_RrRmLampBrightCmd_enum"
  VBCM_WelcomeDemoSta_flg/1 -> VBCM_WelcomeDemoSta_flg_Inproc/1  "VBCM_WelcomeDemoSta_flg"
  VBCM_WelcomeDemoSta_flg_Inproc/1 -> UnitConverter195/1
  UnitConverter195/1 -> VOUTP_WelcomeDemoSta_flg/1  "VOUTP_WelcomeDemoSta_flg"
  VBCM_FrAtmoLampCmd_flg/1 -> VBCM_FrAtmoLampCmd_flg_Inproc/1  "VBCM_FrAtmoLampCmd_flg"
  VBCM_FrAtmoLampCmd_flg_Inproc/1 -> UnitConverter196/1
  UnitConverter196/1 -> VOUTP_FrAtmoLampCmd_flg/1  "VOUTP_FrAtmoLampCmd_flg"
  VBCM_RrAtmoLampCmd_flg/1 -> VBCM_RrAtmoLampCmd_flg_Inproc/1  "VBCM_RrAtmoLampCmd_flg"
  VBCM_RrAtmoLampCmd_flg_Inproc/1 -> UnitConverter197/1
  UnitConverter197/1 -> VOUTP_RrAtmoLampCmd_flg/1  "VOUTP_RrAtmoLampCmd_flg"
  VBCM_TgateHDSWLSta_flg/1 -> VBCM_TgateHDSWLSta_flg_Inproc/1  "VBCM_TgateHDSWLSta_flg"
  VBCM_TgateHDSWLSta_flg_Inproc/1 -> UnitConverter198/1
  UnitConverter198/1 -> VOUTP_TgateHDSWLSta_flg/1  "VOUTP_TgateHDSWLSta_flg"
  VBCM_TgateHDSWRSta_flg/1 -> VBCM_TgateHDSWRSta_flg_Inproc/1  "VBCM_TgateHDSWRSta_flg"
  VBCM_TgateHDSWRSta_flg_Inproc/1 -> UnitConverter199/1
  UnitConverter199/1 -> VOUTP_TgateHDSWRSta_flg/1  "VOUTP_TgateHDSWRSta_flg"
  VBCM_TgateSWLSta_flg/1 -> VBCM_TgateSWLSta_flg_Inproc/1  "VBCM_TgateSWLSta_flg"
  VBCM_TgateSWLSta_flg_Inproc/1 -> UnitConverter200/1
  UnitConverter200/1 -> VOUTP_TgateSWLSta_flg/1  "VOUTP_TgateSWLSta_flg"
  VBCM_TgateSWRSta_flg/1 -> VBCM_TgateSWRSta_flg_Inproc/1  "VBCM_TgateSWRSta_flg"
  VBCM_TgateSWRSta_flg_Inproc/1 -> UnitConverter201/1
  UnitConverter201/1 -> VOUTP_TgateSWRSta_flg/1  "VOUTP_TgateSWRSta_flg"
  VBCM_LTgateRelCmd_flg/1 -> VBCM_LTgateRelCmd_flg_Inproc/1  "VBCM_LTgateRelCmd_flg"
  VBCM_LTgateRelCmd_flg_Inproc/1 -> UnitConverter202/1
  UnitConverter202/1 -> VOUTP_LTgateRelCmd_flg/1  "VOUTP_LTgateRelCmd_flg"
  VBCM_RTgateRelCmd_flg/1 -> VBCM_RTgateRelCmd_flg_Inproc/1  "VBCM_RTgateRelCmd_flg"
  VBCM_RTgateRelCmd_flg_Inproc/1 -> UnitConverter203/1
  UnitConverter203/1 -> VOUTP_RTgateRelCmd_flg/1  "VOUTP_RTgateRelCmd_flg"
  VBCM_FDDoorOpen_enum/1 -> VBCM_FDDoorOpen_enum_Inproc/1  "VBCM_FDDoorOpen_enum"
  VBCM_FDDoorOpen_enum_Inproc/1 -> UnitConverter204/1
  UnitConverter204/1 -> VOUTP_FDDoorOpen_enum/1  "VOUTP_FDDoorOpen_enum"
  VBCM_FDDoorstate_enum/1 -> VBCM_FDDoorstate_enum_Inproc/1  "VBCM_FDDoorstate_enum"
  VBCM_FDDoorstate_enum_Inproc/1 -> UnitConverter205/1
  UnitConverter205/1 -> VOUTP_FDDoorstate_enum/1  "VOUTP_FDDoorstate_enum"
  VDHP_ActAPSPosn_pct/1 -> VDHP_ActAPSPosn_pct_Inproc/1  "VDHP_ActAPSPosn_pct"
  VDHP_ActAPSPosn_pct_Inproc/1 -> UnitConverter206/1
  UnitConverter206/1 -> VOUTP_ActAPSPosn_pct/1  "VOUTP_ActAPSPosn_pct"
  VDHP_EAPS1MIN_pct/1 -> VDHP_EAPS1MIN_pct_Inproc/1  "VDHP_EAPS1MIN_pct"
  VDHP_EAPS1MIN_pct_Inproc/1 -> UnitConverter207/1
  UnitConverter207/1 -> VOUTP_EAPS1MIN_pct/1  "VOUTP_EAPS1MIN_pct"
  VDHP_EAPS2MIN_pct/1 -> VDHP_EAPS2MIN_pct_Inproc/1  "VDHP_EAPS2MIN_pct"
  VDHP_EAPS2MIN_pct_Inproc/1 -> UnitConverter208/1
  UnitConverter208/1 -> VOUTP_EAPS2MIN_pct/1  "VOUTP_EAPS2MIN_pct"
  VDKC_DKCTimeSN_cnt/1 -> VDKC_DKCTimeSN_cnt_Inproc/1  "VDKC_DKCTimeSN_cnt"
  VDKC_DKCTimeSN_cnt_Inproc/1 -> UnitConverter209/1
  UnitConverter209/1 -> VOUTP_DKCTimeSN_cnt/1  "VOUTP_DKCTimeSN_cnt"
  VDKC_DKCAuthSta_enum/1 -> VDKC_DKCAuthSta_enum_Inproc/1  "VDKC_DKCAuthSta_enum"
  VDKC_DKCAuthSta_enum_Inproc/1 -> UnitConverter210/1
  UnitConverter210/1 -> VOUTP_DKCAuthSta_enum/1  "VOUTP_DKCAuthSta_enum"
  VDSC_DISCTurn_flg/1 -> VDSC_DISCTurn_flg_Inproc/1  "VDSC_DISCTurn_flg"
  VDSC_DISCTurn_flg_Inproc/1 -> UnitConverter211/1
  UnitConverter211/1 -> VOUTP_DISCTurn_flg/1  "VOUTP_DISCTurn_flg"
  VDSC_DISCTargetSpd_kph/1 -> VDSC_DISCTargetSpd_kph_Inproc/1  "VDSC_DISCTargetSpd_kph"
  VDSC_DISCTargetSpd_kph_Inproc/1 -> UnitConverter212/1
  UnitConverter212/1 -> VOUTP_DISCTargetSpd_kph/1  "VOUTP_DISCTargetSpd_kph"
  VDSC_DISCSta_enum/1 -> VDSC_DISCSta_enum_Inproc/1  "VDSC_DISCSta_enum"
  VDSC_DISCSta_enum_Inproc/1 -> UnitConverter213/1
  UnitConverter213/1 -> VOUTP_DISCSta_enum/1  "VOUTP_DISCSta_enum"
  VDSC_DISCButtSta_flg/1 -> VDSC_DISCButtSta_flg_Inproc/1  "VDSC_DISCButtSta_flg"
  VDSC_DISCButtSta_flg_Inproc/1 -> UnitConverter214/1
  UnitConverter214/1 -> VOUTP_DISCButtSta_flg/1  "VOUTP_DISCButtSta_flg"
  VNMM_AllCANTxReq_flg/1 -> VNMM_AllCANTxReq_flg_Inproc/1  "VNMM_AllCANTxReq_flg"
  VNMM_AllCANTxReq_flg_Inproc/1 -> UnitConverter215/1
  UnitConverter215/1 -> VOUTP_AllCANTxReq_flg/1  "VOUTP_AllCANTxReq_flg"
  VNMM_NMmTxReq_flg/1 -> VNMM_NMmTxReq_flg_Inproc/1  "VNMM_NMmTxReq_flg"
  VNMM_NMmTxReq_flg_Inproc/1 -> UnitConverter216/1
  UnitConverter216/1 -> VOUTP_NMmTxReq_flg/1  "VOUTP_NMmTxReq_flg"
  VNMM_Awake_enum/1 -> VNMM_Awake_enum_Inproc/1  "VNMM_Awake_enum"
  VNMM_Awake_enum_Inproc/1 -> UnitConverter217/1
  UnitConverter217/1 -> VOUTP_Awake_enum/1  "VOUTP_Awake_enum"
  VNMM_CSB_flg/1 -> VNMM_CSB_flg_Inproc/1  "VNMM_CSB_flg"
  VNMM_CSB_flg_Inproc/1 -> UnitConverter218/1
  UnitConverter218/1 -> VOUTP_CSB_flg/1  "VOUTP_CSB_flg"
  VNMM_ErrorState_enum/1 -> VNMM_ErrorState_enum_Inproc/1  "VNMM_ErrorState_enum"
  VNMM_ErrorState_enum_Inproc/1 -> UnitConverter219/1
  UnitConverter219/1 -> VOUTP_ErrorState_enum/1  "VOUTP_ErrorState_enum"
  VNMM_NodeID_enum/1 -> VNMM_NodeID_enum_Inproc/1  "VNMM_NodeID_enum"
  VNMM_NodeID_enum_Inproc/1 -> UnitConverter220/1
  UnitConverter220/1 -> VOUTP_NodeID_enum/1  "VOUTP_NodeID_enum"
  VNMM_PNI_flg/1 -> VNMM_PNI_flg_Inproc/1  "VNMM_PNI_flg"
  VNMM_PNI_flg_Inproc/1 -> UnitConverter221/1
  UnitConverter221/1 -> VOUTP_PNI_flg/1  "VOUTP_PNI_flg"
  VNMM_RptMsgReq_flg/1 -> VNMM_RptMsgReq_flg_Inproc/1  "VNMM_RptMsgReq_flg"
  VNMM_RptMsgReq_flg_Inproc/1 -> UnitConverter222/1
  UnitConverter222/1 -> VOUTP_RptMsgReq_flg/1  "VOUTP_RptMsgReq_flg"
  VNMM_WakeUp_enum/1 -> VNMM_WakeUp_enum_Inproc/1  "VNMM_WakeUp_enum"
  VNMM_WakeUp_enum_Inproc/1 -> UnitConverter223/1
  UnitConverter223/1 -> VOUTP_WakeUp_enum/1  "VOUTP_WakeUp_enum"
  VNMM_ActiveWU_flg/1 -> VNMM_ActiveWU_flg_Inproc/1  "VNMM_ActiveWU_flg"
  VNMM_ActiveWU_flg_Inproc/1 -> UnitConverter224/1
  UnitConverter224/1 -> VOUTP_ActiveWU_flg/1  "VOUTP_ActiveWU_flg"
  VNMM_SysNMmSta_enum/1 -> VNMM_SysNMmSta_enum_Inproc/1  "VNMM_SysNMmSta_enum"
  VNMM_SysNMmSta_enum_Inproc/1 -> UnitConverter225/1
  UnitConverter225/1 -> VOUTP_SysNMmSta_enum/1  "VOUTP_SysNMmSta_enum"
